simulink model "Project3_System_partA"  (R2018b)
settings: Solver=VariableStepAuto  StartTime=0.0  StopTime=10  FixedStep=.001  MaxStep=.001  RelTol=1e-6  EnableMultiTasking=on
values from neighbouring files (symbols this model uses):
  Kd = 700    [SimRun.m]
  Kp = 1000    [SimRun.m]
  n = link.inertia*(iwdot) + cross(iw, link.inertia*iw)    [newtonEuler.m]
  points = points3D    [SimRun.m]
  transPercent = 0.025    [SimRun.m]
(part 2 of 4)

== matlab function Project3_System_partA/ABB Arm Dynamics/MATLAB Function ==
  settings: updateMethod=DISCRETE
  data: torque input; theta_ddot output; theta input; theta_dot input
function theta_ddot = fcn(torque, theta, theta_dot )
%#codegen
coder.extrinsic('evalin');
persistent Sim_Exact;

if isempty(Sim_Exact)
    Sim_Exact = evalin('base','Sim_Exact');
end

th1 = theta(1);
th2 = theta(2);
th3 = theta(3);
th4 = theta(4);
th5 = theta(5);
th6 = theta(6);

th_dot1 = theta_dot(1);
th_dot2 = theta_dot(2);
th_dot3 = theta_dot(3);
th_dot4 = theta_dot(4);
th_dot5 = theta_dot(5);
th_dot6 = theta_dot(6);

CFG = zeros(6,1);
M = zeros(6,6);
if Sim_Exact
    CFG =  CFG_vec_exact(th1,th2,th3,th4,th5,th6,th_dot1,th_dot2,th_dot3,th_dot4,th_dot5,th_dot6);
    M = M_mat_exact(th1,th2,th3,th4,th5,th6);
else
    CFG =  CFG_vec_diff(th1,th2,th3,th4,th5,th6,th_dot1,th_dot2,th_dot3,th_dot4,th_dot5,th_dot6);
    M = M_mat_diff(th1,th2,th3,th4,th5,th6);
end

theta_ddot = M^-1 * (torque - CFG);

end

function CFG = CFG_vec_exact(th1,th2,th3,th4,th5,th6,thDot1,thDot2,thDot3,thDot4,thDot5,thDot6)
%CFG_VEC_EXACT
%    CFG = CFG_VEC_EXACT(TH1,TH2,TH3,TH4,TH5,TH6,THDOT1,THDOT2,THDOT3,THDOT4,THDOT5,THDOT6)

%    This function was generated by the Symbolic Math Toolbox version 7.0.
%    21-Nov-2018 15:36:09

t2 = th2+th3;
t3 = sin(t2);
t4 = sin(th6);
t5 = cos(th4);
t6 = cos(t2);
t7 = sin(th4);
t8 = cos(th6);
t9 = cos(th5);
t10 = sin(th1);
t11 = cos(th1);
t12 = sin(th5);
t13 = t6.*t12;
t14 = t3.*t5.*t9;
t15 = t13+t14;
t16 = t7.*t10;
t17 = t5.*t6.*t11;
t18 = t16+t17;
t19 = t9.*t18;
t47 = t3.*t11.*t12;
t20 = t19-t47;
t21 = t5.*t10;
t36 = t6.*t7.*t11;
t22 = t21-t36;
t23 = thDot2+thDot3;
t24 = t11.*t23;
t25 = t5.*t11;
t26 = t6.*t7.*t10;
t27 = t25+t26;
t28 = t27.*thDot5;
t33 = t3.*t10.*thDot4;
t29 = t24-t33;
t30 = t6.*thDot4;
t31 = t3.*t7.*thDot5;
t32 = t30+t31-thDot1;
t34 = t6.*t9;
t95 = t3.*t5.*t12;
t35 = t34-t95;
t37 = t5.*t10.*6.174272671239708e-4;
t49 = t6.*t7.*t11.*6.174272671239708e-4;
t38 = t37-t49;
t39 = t12.*t18.*2.88132724657853e-3;
t40 = t3.*t9.*t11.*2.88132724657853e-3;
t41 = t39+t40;
t42 = t12.*t18;
t43 = t3.*t9.*t11;
t44 = t42+t43;
t45 = t9.*t18.*2.88132724657853e-3;
t50 = t3.*t11.*t12.*2.88132724657853e-3;
t46 = t45-t50;
t48 = t24+t28-t33;
t51 = t7.*t11;
t53 = t5.*t6.*t10;
t52 = t51-t53;
t54 = t12.*t52;
t88 = t3.*t9.*t10;
t55 = t54-t88;
t56 = cos(th2);
t57 = t10.*t23;
t58 = t3.*t11.*thDot4;
t59 = t57+t58;
t60 = t30-thDot1;
t61 = thDot1.^2;
t62 = thDot2.^2;
t63 = cos(th3);
t64 = sin(th2);
t65 = sin(th3);
t66 = thDot3.^2;
t67 = t10.*t64.*thDot1.*thDot2.*(2.7e1./5.0e1);
t68 = t11.*t61.*t64.*t65.*(7.0./1.0e2);
t69 = t11.*t62.*t64.*t65.*(7.0./1.0e2);
t70 = t11.*t64.*t65.*t66.*(7.0./1.0e2);
t71 = t10.*t56.*t65.*thDot1.*thDot2.*(7.0./5.0e1);
t72 = t10.*t63.*t64.*thDot1.*thDot2.*(7.0./5.0e1);
t73 = t10.*t56.*t65.*thDot1.*thDot3.*(7.0./5.0e1);
t74 = t10.*t63.*t64.*thDot1.*thDot3.*(7.0./5.0e1);
t75 = t11.*t64.*t65.*thDot2.*thDot3.*(7.0./5.0e1);
t76 = t6.*7.0;
t77 = t56.*2.7e1;
t78 = t76+t77;
t79 = t11.*t56.*(2.7e1./1.0e2);
t80 = t6.*t11.*(7.0./2.0e2);
t132 = t11.*t78.*(1.0./1.0e2);
t81 = t79+t80-t132;
t82 = t10.*t56.*(2.7e1./1.0e2);
t83 = t6.*t10.*(7.0./2.0e2);
t168 = t10.*t78.*(1.0./1.0e2);
t84 = t82+t83-t168;
t85 = t9.*t52;
t86 = t3.*t10.*t12;
t87 = t85+t86;
t89 = t55.*thDot6;
t90 = t22.*thDot5;
t91 = t8.*t27.*(9.0./2.5e2);
t92 = t12.*t52.*(9.0./1.25e2);
t144 = t4.*t87.*(9.0./2.5e2);
t145 = t3.*t9.*t10.*(9.0./1.25e2);
t93 = t91+t92-t144-t145;
t94 = t24+t28-t33+t89;
t96 = t35.*thDot6;
t97 = t30+t31+t96-thDot1;
t98 = t8.*t22.*(9.0./2.5e2);
t99 = t12.*t18.*(9.0./1.25e2);
t100 = t3.*t9.*t11.*(9.0./1.25e2);
t133 = t4.*t20.*(9.0./2.5e2);
t101 = t98+t99+t100-t133;
t102 = t44.*thDot6;
t103 = t57+t58+t90+t102;
t104 = t4.*t15.*(9.0./2.5e2);
t105 = t6.*t9.*(9.0./1.25e2);
t106 = t3.*t7.*t8.*(9.0./2.5e2);
t147 = t3.*t5.*t12.*(9.0./1.25e2);
t107 = t104+t105+t106-t147;
t108 = t57+t58+t90;
t109 = t59.*thDot1;
t110 = t10.*t23.*thDot1;
t111 = t11.*t56.*t61.*t65.*(1.51e2./5.0e2);
t112 = t11.*t61.*t63.*t64.*(1.51e2./5.0e2);
t113 = t11.*t56.*t62.*t65.*(1.51e2./5.0e2);
t114 = t11.*t62.*t63.*t64.*(1.51e2./5.0e2);
t115 = t11.*t56.*t65.*t66.*(1.51e2./5.0e2);
t116 = t11.*t63.*t64.*t66.*(1.51e2./5.0e2);
t117 = t10.*t56.*t63.*thDot1.*thDot2.*(1.51e2./2.5e2);
t118 = t10.*t56.*t63.*thDot1.*thDot3.*(1.51e2./2.5e2);
t119 = t11.*t56.*t65.*thDot2.*thDot3.*(1.51e2./2.5e2);
t120 = t11.*t63.*t64.*thDot2.*thDot3.*(1.51e2./2.5e2);
t121 = t8.*t15.*6.694531704772773e-4;
t203 = t3.*t4.*t7.*6.694531704772773e-4;
t122 = t121-t203;
t123 = t4.*t15.*3.556381058634072e-4;
t124 = t3.*t7.*t8.*3.556381058634072e-4;
t125 = t123+t124;
t126 = t6.*t9.*6.694531704772773e-4;
t202 = t3.*t5.*t12.*6.694531704772773e-4;
t127 = t126-t202;
t128 = t32.*t59;
t129 = t97.*t108;
t130 = t10.*t23.*(t30-thDot1);
t227 = t60.*t108;
t288 = t32.*t103;
t131 = t109+t110+t128+t129+t130-t227-t288;
t134 = t3.*thDot2.*thDot4;
t135 = t3.*thDot3.*thDot4;
t136 = t3.*t9.*thDot2.*thDot6;
t137 = t3.*t9.*thDot3.*thDot6;
t138 = t6.*t12.*thDot5.*thDot6;
t139 = t5.*t6.*t12.*thDot2.*thDot6;
t140 = t5.*t6.*t12.*thDot3.*thDot6;
t141 = t3.*t5.*t9.*thDot5.*thDot6;
t209 = t6.*t7.*thDot2.*thDot5;
t210 = t6.*t7.*thDot3.*thDot5;
t211 = t3.*t5.*thDot4.*thDot5;
t212 = t3.*t7.*t12.*thDot4.*thDot6;
t142 = t134+t135+t136+t137+t138+t139+t140+t141-t209-t210-t211-t212;
t143 = t94.*t101;
t248 = t93.*t103;
t146 = t143-t248;
t148 = t29.*thDot1;
t149 = t29.*t32;
t150 = t48.*t97;
t151 = t11.*t23.*thDot1;
t152 = t11.*t23.*t60;
t153 = t3.*t11.*t29.*(1.51e2./1.0e3);
t154 = t3.*t10.*t59.*(1.51e2./1.0e3);
t155 = t153+t154;
t156 = t10.*t56.*t61.*(2.7e1./1.0e2);
t157 = t10.*t56.*t62.*(2.7e1./1.0e2);
t158 = t11.*t64.*thDot1.*thDot2.*(2.7e1./5.0e1);
t159 = t3.^2;
t160 = t10.*t56.*t61.*t63.*(7.0./1.0e2);
t161 = t10.*t56.*t62.*t63.*(7.0./1.0e2);
t162 = t10.*t56.*t63.*t66.*(7.0./1.0e2);
t163 = t11.*t56.*t65.*thDot1.*thDot2.*(7.0./5.0e1);
t164 = t11.*t63.*t64.*thDot1.*thDot2.*(7.0./5.0e1);
t165 = t11.*t56.*t65.*thDot1.*thDot3.*(7.0./5.0e1);
t166 = t11.*t63.*t64.*thDot1.*thDot3.*(7.0./5.0e1);
t167 = t10.*t56.*t63.*thDot2.*thDot3.*(7.0./5.0e1);
t169 = t11.*t23.*t81;
t170 = t10.*t23.*t84;
t171 = t169+t170;
t172 = t11.*t56.*t63.*thDot1.*thDot2.*(1.51e2./2.5e2);
t173 = t11.*t56.*t63.*thDot1.*thDot3.*(1.51e2./2.5e2);
t174 = t12.*t52.*6.694531704772773e-4;
t186 = t3.*t9.*t10.*6.694531704772773e-4;
t175 = t174-t186;
t176 = t8.*t87.*6.694531704772773e-4;
t177 = t4.*t27.*6.694531704772773e-4;
t178 = t176+t177;
t179 = t4.*t22;
t180 = t8.*t20;
t181 = t179+t180;
t182 = t8.*t27.*3.556381058634072e-4;
t183 = t4.*t20;
t243 = t8.*t22;
t184 = t183-t243;
t190 = t4.*t87.*3.556381058634072e-4;
t185 = t182-t190;
t187 = t8.*t87;
t188 = t4.*t27;
t189 = t187+t188;
t191 = t8.*t27;
t245 = t4.*t87;
t192 = t191-t245;
t193 = t5.*t11.*6.174272671239708e-4;
t194 = t6.*t7.*t10.*6.174272671239708e-4;
t195 = t193+t194;
t196 = t12.*t52.*2.88132724657853e-3;
t201 = t3.*t9.*t10.*2.88132724657853e-3;
t197 = t196-t201;
t198 = t9.*t52.*2.88132724657853e-3;
t199 = t3.*t10.*t12.*2.88132724657853e-3;
t200 = t198+t199;
t204 = t8.*t15;
t234 = t3.*t4.*t7;
t205 = t204-t234;
t206 = t4.*t15;
t207 = t3.*t7.*t8;
t208 = t206+t207;
t213 = t6.*t9.*2.88132724657853e-3;
t226 = t3.*t5.*t12.*2.88132724657853e-3;
t214 = t213-t226;
t215 = t6.*t12.*2.88132724657853e-3;
t216 = t3.*t5.*t9.*2.88132724657853e-3;
t217 = t215+t216;
t218 = t5.*t10.*1.570529909265897e-1;
t223 = t6.*t7.*t11.*1.570529909265897e-1;
t219 = t218-t223;
t220 = t7.*t10.*1.570529909265897e-1;
t221 = t5.*t6.*t11.*1.570529909265897e-1;
t222 = t220+t221;
t224 = t3.*t6.*t11.*2.386726843794421e-2;
t225 = t148+t151+t152;
t228 = t7.*t11.*1.570529909265897e-1;
t233 = t5.*t6.*t10.*1.570529909265897e-1;
t229 = t228-t233;
t230 = t5.*t11.*1.570529909265897e-1;
t231 = t6.*t7.*t10.*1.570529909265897e-1;
t232 = t230+t231;
t235 = t12.*t18.*6.694531704772773e-4;
t236 = t3.*t9.*t11.*6.694531704772773e-4;
t237 = t235+t236;
t238 = t4.*t22.*6.694531704772773e-4;
t239 = t8.*t20.*6.694531704772773e-4;
t240 = t238+t239;
t241 = t4.*t20.*3.556381058634072e-4;
t244 = t8.*t22.*3.556381058634072e-4;
t242 = t241-t244;
t246 = t3.*t6.*t10.*2.386726843794421e-2;
t247 = t101.*t142;
t249 = t93.*t97;
t274 = t94.*t107;
t250 = t249-t274;
t251 = t97.*t250;
t275 = t48.*t60;
t276 = t32.*t94;
t252 = t148+t149+t150+t151+t152-t275-t276;
t253 = t107.*t252;
t254 = t10.*t56.*t61.*t65.*(1.51e2./5.0e2);
t255 = t10.*t61.*t63.*t64.*(1.51e2./5.0e2);
t256 = t10.*t56.*t62.*t65.*(1.51e2./5.0e2);
t257 = t10.*t62.*t63.*t64.*(1.51e2./5.0e2);
t258 = t10.*t56.*t65.*t66.*(1.51e2./5.0e2);
t259 = t10.*t63.*t64.*t66.*(1.51e2./5.0e2);
t260 = t10.*t61.*t64.*t65.*(7.0./1.0e2);
t261 = t10.*t62.*t64.*t65.*(7.0./1.0e2);
t262 = t10.*t64.*t65.*t66.*(7.0./1.0e2);
t263 = t11.*t64.*t65.*thDot1.*thDot2.*(1.51e2./2.5e2);
t264 = t11.*t64.*t65.*thDot1.*thDot3.*(1.51e2./2.5e2);
t265 = t10.*t56.*t65.*thDot2.*thDot3.*(1.51e2./2.5e2);
t266 = t10.*t63.*t64.*thDot2.*thDot3.*(1.51e2./2.5e2);
t267 = t10.*t64.*t65.*thDot2.*thDot3.*(7.0./5.0e1);
t268 = t6.*t29.*(1.51e2./1.0e3);
t269 = t3.*t10.*t60.*(1.51e2./1.0e3);
t270 = t268+t269;
t271 = t11.*t23.*t159.*thDot4.*(1.51e2./1.0e3);
t272 = t6.*t225.*(1.51e2./1.0e3);
t273 = -t156-t157-t158-t160-t161-t162-t163-t164-t165-t166-t167-t172-t173+t254+t255+t256+t257+t258+t259+t260+t261+t262+t263+t264+t265+t266+t267;
t277 = t156+t157+t158+t160+t161+t162+t163+t164+t165+t166+t167+t172+t173+t247+t251+t253-t254-t255-t256-t257-t258-t259-t260-t261-t262-t263-t264-t265-t266-t267-t103.*t146;
t278 = t277.*pi.*3.6225e-1;
t297 = t59.*t155;
t298 = t60.*t270;
t279 = t156+t157+t158+t160+t161+t162+t163+t164+t165+t166+t167-t260-t261-t262-t267+t271+t272-t297-t298;
t280 = t279.*pi.*6.07775;
t281 = t10.^2;
t282 = t6.^2;
t283 = t11.^2;
t284 = -t91-t92+t144+t145;
t285 = t97.*t101;
t329 = t103.*t107;
t286 = t285-t329;
t287 = t97.*t286;
t289 = t107.*t131;
t290 = t56.^2;
t291 = t64.^2;
t292 = t10.*t11.*t282.*5.532148313430778e-3;
t293 = t10.*t11.*t159.*4.573242605769442e-3;
t407 = t10.*t11.*4.573242605769442e-3;
t294 = t292+t293-t407;
t295 = t103.*t284;
t296 = t143+t295;
t299 = t84.*thDot1;
t345 = t3.*t11.*t23.*(7.0./2.0e2);
t300 = t299-t345;
t301 = t3.*t11.*t23.*thDot1.*(7.0./2.0e2);
t346 = t300.*thDot1;
t347 = t10.*t23.*t171;
t302 = t156+t157+t158+t301-t346-t347;
t303 = t302.*pi.*1.40875;
t304 = t10.*t11.*t290.*1.080250746560099e-1;
t305 = t10.*t11.*t291.*2.873466985849863e-1;
t399 = t10.*t11.*2.873466985849863e-1;
t306 = t304+t305-t399;
t307 = t103.*t296;
t308 = t97.*t284;
t309 = t274+t308;
t310 = t97.*t309;
t311 = -t156-t157-t158-t160-t161-t162-t163-t164-t165-t166-t167-t172-t173-t247-t253+t254+t255+t256+t257+t258+t259+t260+t261+t262+t263+t264+t265+t266+t267+t307+t310;
t312 = t109+t110+t130;
t313 = t29.*t155;
t314 = t6.*t59.*(1.51e2./1.0e3);
t339 = t3.*t11.*t60.*(1.51e2./1.0e3);
t315 = t314-t339;
t316 = t10.*t23.*t159.*thDot4.*(1.51e2./1.0e3);
t324 = t11.*t56.*t61.*(2.7e1./1.0e2);
t325 = t11.*t56.*t62.*(2.7e1./1.0e2);
t330 = t11.*t56.*t61.*t63.*(7.0./1.0e2);
t331 = t11.*t56.*t62.*t63.*(7.0./1.0e2);
t332 = t11.*t56.*t63.*t66.*(7.0./1.0e2);
t333 = t11.*t56.*t63.*thDot2.*thDot3.*(7.0./5.0e1);
t334 = t10.*t64.*t65.*thDot1.*thDot2.*(1.51e2./2.5e2);
t335 = t10.*t64.*t65.*thDot1.*thDot3.*(1.51e2./2.5e2);
t317 = t67+t68+t69+t70+t71+t72+t73+t74+t75+t111+t112+t113+t114+t115+t116+t117+t118+t119+t120-t324-t325-t330-t331-t332-t333-t334-t335;
t318 = t317.*pi.*(1.61e2./2.56e2);
t319 = t81.*thDot1;
t320 = t3.*t10.*t23.*(7.0./2.0e2);
t321 = t319+t320;
t322 = t321.*thDot1;
t323 = t11.*t23.*t171;
t326 = t3.*t10.*t23.*thDot1.*(7.0./2.0e2);
t327 = t142.*t284;
t328 = t94.*t296;
t336 = t67+t68+t69+t70+t71+t72+t73+t74+t75+t111+t112+t113+t114+t115+t116+t117+t118+t119+t120+t287+t289-t324-t325+t327+t328-t330-t331-t332-t333-t334-t335;
t337 = t336.*pi.*3.6225e-1;
t338 = t6.*t312.*(1.51e2./1.0e3);
t342 = t60.*t315;
t340 = t67+t68+t69+t70+t71+t72+t73+t74+t75+t313+t316-t324-t325-t330-t331-t332-t333+t338-t342;
t341 = t340.*pi.*6.07775;
t343 = t318+t337+t341;
t344 = t311.*pi.*3.6225e-1;
t348 = t273.*pi.*(1.61e2./2.56e2);
t349 = t56.*t283.*thDot2.*(2.7e1./2.0e2);
t350 = t56.*t281.*thDot2.*(2.7e1./2.0e2);
t351 = t349+t350;
t352 = t67+t322+t323-t324-t325+t326;
t353 = t352.*pi.*1.40875;
t354 = t7.^2;
t355 = t205.*t240;
t356 = t208.*t242;
t586 = t35.*t237;
t357 = t355+t356-t586;
t358 = t44.*t237;
t359 = t181.*t240;
t360 = t184.*t242;
t361 = t358+t359+t360;
t362 = t103.*t361;
t363 = t55.*t237;
t364 = t189.*t240;
t558 = t192.*t242;
t365 = t363+t364-t558;
t366 = t94.*t365;
t605 = t97.*t357;
t367 = t362+t366-t605;
t368 = t35.*t197;
t369 = t3.*t7.*t195;
t549 = t15.*t200;
t370 = t368+t369-t549;
t371 = -t134-t135+t209+t210+t211;
t372 = t11.*t56.*thDot1.*(2.7e1./2.0e2);
t520 = t10.*t64.*thDot2.*(2.7e1./2.0e2);
t373 = t372-t520;
t374 = t373.*thDot1;
t375 = t11.*t351.*thDot2;
t376 = t374+t375-t10.*t64.*thDot1.*thDot2.*(2.7e1./2.0e2);
t377 = t318+t337+t341+t353-t376.*pi.*1.22259375e1;
t378 = t282.*2.386726843794421e-2;
t379 = t5.^2;
t380 = t159.*t379.*1.570529909265897e-1;
t381 = t159.*t354.*1.570529909265897e-1;
t382 = t378+t380+t381;
t383 = t3.*t7.*t22.*1.570529909265897e-1;
t555 = t3.*t5.*t18.*1.570529909265897e-1;
t384 = t224+t383-t555;
t385 = t3.*t5.*t52.*1.570529909265897e-1;
t557 = t3.*t7.*t27.*1.570529909265897e-1;
t386 = t246+t385-t557;
t387 = t22.*t195;
t388 = t44.*t197;
t389 = t20.*t200;
t390 = t387+t388+t389;
t391 = t44.*t175;
t392 = t178.*t181;
t573 = t184.*t185;
t393 = t391+t392-t573;
t394 = t11.*t23.*(t30-thDot1);
t395 = t159.*t281.*2.386726843794421e-2;
t396 = t27.*t232;
t397 = t52.*t229;
t398 = t395+t396+t397;
t400 = t11.*t306.*thDot2;
t401 = t281.*2.873466985849863e-1;
t402 = t283.*t290.*1.080250746560099e-1;
t403 = t283.*t291.*2.873466985849863e-1;
t404 = t401+t402+t403;
t405 = t11.*t56.*t64.*thDot1.*1.793216239289764e-1;
t406 = t400+t405-t10.*t404.*thDot2;
t408 = t281.*4.573242605769442e-3;
t409 = t282.*t283.*5.532148313430778e-3;
t410 = t159.*t283.*4.573242605769442e-3;
t411 = t408+t409+t410;
t412 = t10.*t23.*t411;
t413 = t3.*t6.*t11.*thDot1.*9.589057076613353e-4;
t610 = t11.*t23.*t294;
t414 = t412+t413-t610;
t415 = t35.*t127;
t416 = t122.*t205;
t417 = t125.*t208;
t418 = t415+t416+t417;
t419 = t122.*t181;
t420 = t125.*t184;
t569 = t44.*t127;
t421 = t419+t420-t569;
t422 = t125.*t192;
t423 = t55.*t127;
t570 = t122.*t189;
t424 = t422+t423-t570;
t425 = t15.*t217;
t426 = t35.*t214;
t427 = t159.*t354.*6.174272671239708e-4;
t428 = t425+t426+t427;
t429 = t44.*t214;
t430 = t3.*t7.*t22.*6.174272671239708e-4;
t563 = t20.*t217;
t431 = t429+t430-t563;
t432 = t55.*t214;
t433 = t3.*t7.*t27.*6.174272671239708e-4;
t565 = t87.*t217;
t434 = t432+t433-t565;
t435 = t27.*t195;
t436 = t87.*t200;
t437 = t55.*t197;
t438 = t435+t436+t437;
t439 = t109+t110+t128+t130-t227;
t440 = t318+t337+t341+t353;
t441 = t55.*t175;
t442 = t178.*t189;
t443 = t185.*t192;
t444 = t441+t442+t443;
t445 = t62.*t64.*(2.7e1./1.0e2);
t446 = t148+t149+t150+t151-t275-t276+t394;
t447 = t3.*t62.*(7.0./1.0e2);
t448 = t3.*t66.*(7.0./1.0e2);
t449 = t3.*thDot2.*thDot3.*(7.0./5.0e1);
t450 = t6.*t62.*(1.51e2./5.0e2);
t451 = t6.*t66.*(1.51e2./5.0e2);
t452 = t6.*thDot2.*thDot3.*(1.51e2./2.5e2);
t453 = t318+t337;
t454 = t18.*t229;
t455 = t22.*t232;
t465 = t10.*t11.*t159.*2.386726843794421e-2;
t456 = t454+t455-t465;
t457 = t148+t151+t394;
t458 = t159.*t283.*2.386726843794421e-2;
t459 = t18.*t222;
t460 = t22.*t219;
t461 = t458+t459+t460;
t462 = t59.*t461;
t463 = t27.*t219;
t464 = t52.*t222;
t466 = -t30+thDot1;
t467 = t3.*t7.*t219;
t604 = t3.*t5.*t222;
t468 = t224+t467-t604;
t469 = t35.*t41;
t470 = t3.*t7.*t38;
t592 = t15.*t46;
t471 = t469+t470-t592;
t472 = t32.*t471;
t473 = t22.*t38;
t474 = t41.*t44;
t475 = t20.*t46;
t476 = t473+t474+t475;
t477 = t108.*t476;
t478 = t27.*t38;
t479 = t46.*t87;
t480 = t41.*t55;
t481 = t478+t479+t480;
t482 = t48.*t481;
t483 = t472+t477+t482;
t484 = t185.*t208;
t485 = t35.*t175;
t572 = t178.*t205;
t486 = t484+t485-t572;
t495 = t10.*t23.*t466;
t487 = t109+t110-t495;
t488 = t6.*t487.*(1.51e2./1.0e3);
t489 = t3.*t11.*t466.*(1.51e2./1.0e3);
t490 = t314+t489;
t491 = t466.*t490;
t492 = t67+t68+t69+t70+t71+t72+t73+t74+t75+t313+t316-t324-t325-t330-t331-t332-t333+t488+t491;
t493 = t492.*pi.*6.07775;
t494 = t108.*t466;
t496 = t10.*t23.*t321;
t497 = t11.*t23.*t84.*thDot1;
t511 = t11.*t23.*t300;
t512 = t10.*t23.*t81.*thDot1;
t498 = t445+t496+t497-t511-t512+4.9e1./5.0;
t499 = t498.*pi.*1.40875;
t500 = t94.*t309;
t501 = t109+t110+t128+t129-t288+t494-t495;
t502 = t445+t447+t448+t449+t450+t451+t452+4.9e1./5.0;
t503 = t502.*pi.*(1.61e2./2.56e2);
t504 = t107.*t501;
t505 = t67+t68+t69+t70+t71+t72+t73+t74+t75+t111+t112+t113+t114+t115+t116+t117+t118+t119+t120+t287-t324-t325+t327+t328-t330-t331-t332-t333-t334-t335+t504;
t506 = t48.*t466;
t516 = t11.*t23.*t466;
t507 = t148+t149+t150+t151-t276+t506-t516;
t508 = t284.*t507;
t521 = t103.*t286;
t522 = t101.*t501;
t509 = t445+t447+t448+t449+t450+t451+t452+t500+t508-t521-t522+4.9e1./5.0;
t510 = t509.*pi.*3.6225e-1;
t513 = t59.*t490;
t523 = t3.*t10.*t466.*(1.51e2./1.0e3);
t514 = t268-t523;
t515 = t29.*t514;
t517 = t10.*t56.*thDot1.*(2.7e1./2.0e2);
t518 = t11.*t64.*thDot2.*(2.7e1./2.0e2);
t519 = t517+t518;
t524 = t148+t151-t516;
t525 = t3.*t10.*t524.*(1.51e2./1.0e3);
t528 = t3.*t11.*t487.*(1.51e2./1.0e3);
t526 = t445+t447+t448+t449+t513+t515+t525-t528+4.9e1./5.0;
t527 = t526.*pi.*6.07775;
t529 = t503+t510+t527;
t530 = t283.*4.573242605769442e-3;
t531 = t281.*t282.*5.532148313430778e-3;
t532 = t159.*t281.*4.573242605769442e-3;
t533 = t530+t531+t532;
t534 = t283.*2.873466985849863e-1;
t535 = t281.*t290.*1.080250746560099e-1;
t536 = t281.*t291.*2.873466985849863e-1;
t537 = t534+t535+t536;
t538 = t3.*t5.*t229;
t591 = t3.*t7.*t232;
t539 = t246+t538-t591;
t540 = t505.*pi.*3.6225e-1;
t541 = t318+t493+t540;
t547 = t107.*t507;
t542 = -t156-t157-t158-t160-t161-t162-t163-t164-t165-t166-t167-t172-t173-t247+t254+t255+t256+t257+t258+t259+t260+t261+t262+t263+t264+t265+t266+t267+t307+t310-t547;
t543 = t6.*t524.*(1.51e2./1.0e3);
t544 = t466.*t514;
t545 = t156+t157+t158+t160+t161+t162+t163+t164+t165+t166+t167-t260-t261-t262-t267+t271-t297+t543+t544;
t546 = t545.*pi.*6.07775;
t548 = t542.*pi.*3.6225e-1;
t550 = t32.*t370;
t551 = t108.*t390;
t552 = t48.*t438;
t553 = t550+t551+t552;
t554 = t348-t546+t548;
t556 = t59.*t384;
t559 = t11.*t537.*thDot2;
t560 = t10.*t56.*t64.*thDot1.*1.793216239289764e-1;
t561 = t559+t560-t10.*t306.*thDot2;
t562 = t32.*t428;
t564 = t108.*t431;
t566 = t48.*t434;
t567 = t562+t564+t566;
t568 = t97.*t418;
t571 = t94.*t424;
t574 = t103.*t393;
t575 = t94.*t444;
t576 = t97.*t486;
t577 = t574+t575+t576;
t578 = t519.*thDot1;
t579 = t10.*t351.*thDot2;
t580 = t11.*t64.*thDot1.*thDot2.*(2.7e1./2.0e2);
t581 = t578+t579+t580;
t582 = t581.*pi.*1.22259375e1;
t583 = t10.*t23.*t294;
t584 = t3.*t6.*t10.*thDot1.*9.589057076613353e-4;
t634 = t11.*t23.*t533;
t585 = t583+t584-t634;
t587 = t463+t464-t465;
t588 = t499+t503+t510+t527;
t589 = t29.*t398;
t590 = t59.*t456;
t593 = t503+t510;
t594 = t11.*t519.*thDot2;
t595 = t594-t10.*t373.*thDot2+4.9e1./5.0;
t596 = t595.*pi.*1.22259375e1;
t597 = t499+t503+t510+t527+t596;
t598 = t282.*4.573242605769442e-3;
t599 = t159.*5.532148313430778e-3;
t600 = t598+t599;
t601 = t290.*2.873466985849863e-1;
t602 = t291.*1.080250746560099e-1;
t603 = t601+t602;
t606 = t382.*t466;
t607 = t29.*t386;
t608 = -t556+t606+t607;
t609 = t148+t149+t151+t506-t516;
t611 = t414.*thDot1;
t632 = t103.*t421;
t612 = t568+t571-t632;
t613 = t103.*t612;
t614 = t108.*t567;
t615 = t109+t110+t128+t494-t495;
t616 = t29.*t587;
t651 = t466.*t468;
t617 = t462+t616-t651;
t618 = t466.*t617;
t619 = t142.*t486;
t620 = t6.*t541.*(1.51e2./1.0e3);
t621 = t3.*t541.*(7.0./2.0e2);
t622 = t107.*t505.*pi.*3.6225e-1;
t623 = t3.*t10.*thDot4.*(1.0./1.0e1);
t624 = t6.*t11.*t529.*(7.0./2.0e2);
t625 = t10.*t23.*t533.*thDot1;
t626 = t11.*t23.*t294.*thDot1;
t627 = t22.*thDot5.*(1.0./1.0e1);
t628 = t361.*t507;
t629 = t461.*t524;
t630 = t476.*t609;
t631 = t48.*t567;
t633 = t44.*thDot6.*(1.0./2.0e1);
t635 = t142.*t357;
t636 = t10.*thDot3.*3.0;
t637 = t348+t548;
t638 = t84.*t588;
t639 = t466.*t539;
t640 = t589+t590+t639;
t641 = t466.*t640;
t642 = t371.*t471;
t643 = t3.*t10.*t529.*(1.51e2./1.0e3);
t644 = t3.*t11.*thDot4.*(1.0./1.0e1);
t645 = t3.*t10.*t593.*(1.51e2./1.0e3);
t646 = t284.*t509.*pi.*3.6225e-1;
t647 = t10.*t23.*t294.*thDot1;
t648 = t11.*t23.*t411.*thDot1;
t649 = t48.*t483;
t650 = t142.*t418;
t652 = t94.*t367;
t653 = t318+t540;
t654 = t3.*t23.*t382.*thDot4;
t655 = t94.*(t568+t571-t632);
t656 = t97.*(t484+t485-t572);
t657 = (t182-t190).*(t191-t245);
t658 = t441+t442+t657;
t659 = t94.*t658;
t660 = t574+t656+t659;
t661 = t398.*t487;
t662 = t438.*t615;
t663 = t6.*t653.*(1.51e2./1.0e3);
t664 = t97.*t367;
t665 = t370.*t371;
t666 = t27.*thDot5.*(1.0./1.0e1);
t667 = t390.*t609;
t668 = t393.*t507;
t669 = t55.*thDot6.*(1.0./2.0e1);
t670 = t32.*t483;
t671 = t101.*t509.*pi.*3.6225e-1;
t672 = t103.*t660;
t673 = t108.*t553;
t674 = t371.*t428;
t675 = t431.*t609;
t676 = t35.*thDot6.*(1.0./2.0e1);
t677 = t3.*t7.*thDot5.*(1.0./1.0e1);
t678 = t101.*t542.*pi.*3.6225e-1;
t679 = t421.*t507;
t680 = t284.*t505.*pi.*3.6225e-1;
t681 = t424.*t501;
CFG = [t649+t650+t652+t654+thDot1.*3.0+t421.*(t148+t149+t150+t151+t152-t32.*(t24+t28+t89-t3.*t10.*thDot4)+(thDot1-t6.*thDot4).*(t24+t28-t3.*t10.*thDot4))+t131.*t424-t225.*t384-t108.*t553-t103.*t577-t312.*t386-t371.*t428+t434.*t439-t6.*thDot4.*(1.0./1.0e1)-t35.*thDot6.*(1.0./2.0e1)-t431.*(t148+t149+t151+t152-t48.*t60)-t59.*(t589+t590-t60.*t539)+t29.*(t462+t29.*(t463+t464-t10.*t11.*t159.*2.386726843794421e-2)+t468.*(t30-thDot1))+t84.*(t318+pi.*(t67+t68+t69+t70+t71+t72+t73+t74+t75+t111+t112+t113+t114+t115+t116+t117+t118+t119+t120+t287+t289-t93.*t142+t94.*t146-t11.*t56.*t61.*(2.7e1./1.0e2)-t11.*t56.*t62.*(2.7e1./1.0e2)-t11.*t56.*t61.*t63.*(7.0./1.0e2)-t11.*t56.*t62.*t63.*(7.0./1.0e2)-t11.*t56.*t63.*t66.*(7.0./1.0e2)-t11.*t56.*t63.*thDot2.*thDot3.*(7.0./5.0e1)-t10.*t64.*t65.*thDot1.*thDot2.*(1.51e2./2.5e2)-t10.*t64.*t65.*thDot1.*thDot3.*(1.51e2./2.5e2)).*3.6225e-1+pi.*(t67+t322+t323+t326-t11.*t56.*t61.*(2.7e1./1.0e2)-t11.*t56.*t62.*(2.7e1./1.0e2)).*1.40875+pi.*(t67+t68+t69+t70+t71+t72+t73+t74+t75+t313+t316-t60.*t315+t6.*(t109+t110+t10.*t23.*t60).*(1.51e2./1.0e3)-t11.*t56.*t61.*(2.7e1./1.0e2)-t11.*t56.*t62.*(2.7e1./1.0e2)-t11.*t56.*t61.*t63.*(7.0./1.0e2)-t11.*t56.*t62.*t63.*(7.0./1.0e2)-t11.*t56.*t63.*t66.*(7.0./1.0e2)-t11.*t56.*t63.*thDot2.*thDot3.*(7.0./5.0e1)).*6.07775)+t81.*(t303-t273.*pi.*(1.61e2./2.56e2)+pi.*(t156+t157+t158+t160+t161+t162+t163+t164+t165+t166+t167+t172+t173+t247+t251+t253-t103.*t146-t10.*t56.*t61.*t65.*(1.51e2./5.0e2)-t10.*t56.*t62.*t65.*(1.51e2./5.0e2)-t10.*t56.*t65.*t66.*(1.51e2./5.0e2)-t10.*t61.*t63.*t64.*(1.51e2./5.0e2)-t10.*t62.*t63.*t64.*(1.51e2./5.0e2)-t10.*t61.*t64.*t65.*(7.0./1.0e2)-t10.*t62.*t64.*t65.*(7.0./1.0e2)-t10.*t63.*t64.*t66.*(1.51e2./5.0e2)-t10.*t64.*t65.*t66.*(7.0./1.0e2)-t10.*t56.*t65.*thDot2.*thDot3.*(1.51e2./2.5e2)-t10.*t63.*t64.*thDot2.*thDot3.*(1.51e2./2.5e2)-t11.*t64.*t65.*thDot1.*thDot2.*(1.51e2./2.5e2)-t10.*t64.*t65.*thDot2.*thDot3.*(7.0./5.0e1)-t11.*t64.*t65.*thDot1.*thDot3.*(1.51e2./2.5e2)).*3.6225e-1+pi.*(t156+t157+t158+t160+t161+t162+t163+t164+t165+t166+t167+t271+t272-t59.*t155-t60.*t270-t10.*t61.*t64.*t65.*(7.0./1.0e2)-t10.*t62.*t64.*t65.*(7.0./1.0e2)-t10.*t64.*t65.*t66.*(7.0./1.0e2)-t10.*t64.*t65.*thDot2.*thDot3.*(7.0./5.0e1)).*6.07775)-t11.*t56.*(t280+t303-t344-t348).*(2.7e1./2.0e2)-t11.*t56.*(t280+t303+t582-t273.*pi.*(1.61e2./2.56e2)-t311.*pi.*3.6225e-1).*(2.7e1./2.0e2)-t3.*t11.*(t344+t348).*(1.51e2./1.0e3)-t101.*t311.*pi.*3.6225e-1+t3.*t11.*(t278+t280-t273.*pi.*(1.61e2./2.56e2)).*(1.51e2./1.0e3)-t6.*t11.*(t278+t280-t273.*pi.*(1.61e2./2.56e2)).*(7.0./2.0e2)+t3.*t10.*t343.*(1.51e2./1.0e3)-t6.*t10.*t343.*(7.0./2.0e2)-t10.*t56.*t377.*(2.7e1./2.0e2)+t11.*t23.*t414+t3.*t10.*t453.*(1.51e2./1.0e3)-t10.*t56.*t440.*(2.7e1./2.0e2)+t10.*t23.*t585-t3.*t7.*thDot5.*(1.0./1.0e1)-t11.*t406.*thDot2-t10.*t561.*thDot2+t284.*pi.*(t67+t68+t69+t70+t71+t72+t73+t74+t75+t111+t112+t113+t114+t115+t116+t117+t118+t119+t120+t287+t289+t327+t328-t11.*t56.*t61.*(2.7e1./1.0e2)-t11.*t56.*t62.*(2.7e1./1.0e2)-t11.*t56.*t61.*t63.*(7.0./1.0e2)-t11.*t56.*t62.*t63.*(7.0./1.0e2)-t11.*t56.*t63.*t66.*(7.0./1.0e2)-t11.*t56.*t63.*thDot2.*thDot3.*(7.0./5.0e1)-t10.*t64.*t65.*thDot1.*thDot2.*(1.51e2./2.5e2)-t10.*t64.*t65.*thDot1.*thDot3.*(1.51e2./2.5e2)).*3.6225e-1+t3.*t6.*t23.*t281.*thDot1.*9.589057076613353e-4+t3.*t6.*t23.*t283.*thDot1.*9.589057076613353e-4-t56.*t64.*t281.*thDot1.*thDot2.*1.793216239289764e-1-t56.*t64.*t283.*thDot1.*thDot2.*1.793216239289764e-1;t10.*(t627+t628+t629+t630+t631+t633+t635+t636+t638+t641+t642+t643+t644+t645+t646+t647+t648+t3.*(t303-t348+t546-t542.*pi.*3.6225e-1).*(7.0./2.0e2)+t64.*(t303-t348+t546-t548+t582).*(2.7e1./2.0e2)-t3.*t554.*(7.0./2.0e2)-t6.*t554.*(1.51e2./1.0e3)-t32.*t553-t29.*t608-t6.*t637.*(1.51e2./1.0e3)-t97.*t577+t94.*t612-t365.*t501-t487.*t587-t481.*t615+t10.*thDot2.*3.0+t561.*thDot1-t585.*thDot1+t64.*(t303-t348+t546-t548).*(2.7e1./2.0e2)-t107.*t542.*pi.*3.6225e-1-t6.*t10.*t529.*(7.0./2.0e2)-t10.*t56.*t588.*(2.7e1./2.0e2)-t10.*t56.*t597.*(2.7e1./2.0e2)-t3.*t23.*t468.*thDot4-t11.*t23.*t600.*thDot1+t10.*t306.*thDot1.*thDot2+t11.*t404.*thDot1.*thDot2-t11.*t603.*thDot1.*thDot2)-t11.*(t611+t613+t614+t618+t619+t620+t621+t622+t623+t624+t625+t626-t81.*(t499+t503+pi.*(t445+t447+t448+t449+t450+t451+t452+t500-t521-t101.*t131+t284.*t446+4.9e1./5.0).*3.6225e-1+pi.*(t445+t447+t448+t449+t29.*t270+t59.*t315-t3.*t11.*t312.*(1.51e2./1.0e3)+t3.*t10.*t457.*(1.51e2./1.0e3)+4.9e1./5.0).*6.07775)+t59.*(t556-t29.*t386+t60.*t382)+t64.*t377.*(2.7e1./2.0e2)+t3.*t440.*(7.0./2.0e2)+t6.*t453.*(1.51e2./1.0e3)-t97.*t367+t64.*t440.*(2.7e1./2.0e2)-t32.*t483+t131.*t444+t312.*t398-t370.*t371-t393.*t446+t438.*t439-t456.*t457-t11.*thDot2.*3.0-t11.*thDot3.*3.0-t27.*thDot5.*(1.0./1.0e1)-t55.*thDot6.*(1.0./2.0e1)-t406.*thDot1-t390.*(t148+t149+t151-t275+t394)-t101.*t509.*pi.*3.6225e-1-t3.*t11.*t529.*(1.51e2./1.0e3)-t3.*t11.*t593.*(1.51e2./1.0e3)+t11.*t56.*t588.*(2.7e1./2.0e2)+t11.*t56.*t597.*(2.7e1./2.0e2)-t3.*t23.*t539.*thDot4-t10.*t23.*t600.*thDot1+t11.*t306.*thDot1.*thDot2+t10.*t537.*thDot1.*thDot2-t10.*t603.*thDot1.*thDot2);t10.*(t627+t628+t629+t630+t631+t633+t635+t636+t638+t641+t642+t643+t644+t645+t646+t647+t648+t655-t3.*t554.*(7.0./2.0e2)-t6.*t554.*(1.51e2./1.0e3)-t32.*t553-t29.*t608-t6.*t637.*(1.51e2./1.0e3)-t97.*t577-t365.*t501-t487.*t587-t481.*t615-t585.*thDot1+t3.*(t303-t348+t546-t548).*(7.0./2.0e2)-t107.*t542.*pi.*3.6225e-1-t6.*t10.*t529.*(7.0./2.0e2)-t3.*t23.*t468.*thDot4-t11.*t23.*t600.*thDot1)-t11.*(t611+t613+t614+t618+t619+t620+t621+t622+t623+t624+t625+t626+t661+t662+t663+t3.*(t318+t353+t493+t540).*(7.0./2.0e2)-t97.*t367-t32.*t483-t59.*t608-t81.*t588-t370.*t371-t393.*t507+t444.*t501-t456.*t524-t390.*t609-t11.*thDot3.*3.0-t27.*thDot5.*(1.0./1.0e1)-t55.*thDot6.*(1.0./2.0e1)-t101.*t509.*pi.*3.6225e-1-t3.*t11.*t529.*(1.51e2./1.0e3)-t3.*t11.*t593.*(1.51e2./1.0e3)-t3.*t23.*t539.*thDot4-t10.*t23.*t600.*thDot1);t6.*(-t649-t650-t652-t654+t672+t673+t674+t675+t676+t677+t678-t29.*t617+t59.*t640+t386.*t487+t384.*t524-t424.*t501-t421.*t507-t434.*t615+t6.*thDot4.*(1.0./1.0e1)-t284.*t505.*pi.*3.6225e-1-t3.*t10.*t541.*(1.51e2./1.0e3)+t3.*t11.*t554.*(1.51e2./1.0e3)+t3.*t11.*t637.*(1.51e2./1.0e3)-t3.*t10.*t653.*(1.51e2./1.0e3))+t3.*t11.*(t627+t628+t629+t630+t631+t633+t635+t641+t642+t643+t644+t645+t646+t655-t6.*t554.*(1.51e2./1.0e3)-t32.*t553-t29.*t608-t6.*t637.*(1.51e2./1.0e3)-t97.*t660-t365.*t501-t487.*t587-t481.*t615-t107.*t542.*pi.*3.6225e-1-t3.*t23.*t468.*thDot4)-t3.*t10.*(-t613-t614-t618-t619-t620-t622-t623-t661-t662-t663+t664+t665+t666+t667+t668+t669+t670+t671+t59.*t608+t456.*t524-t501.*t658+t3.*t11.*t529.*(1.51e2./1.0e3)+t3.*t11.*t593.*(1.51e2./1.0e3)+t3.*t23.*t539.*thDot4);t27.*(-t613-t614-t619-t622-t662+t664+t665+t666+t667+t668+t669+t670+t671-t501.*t658)+t22.*(t627+t628+t630+t631+t633+t635+t642+t646+t655-t32.*t553-t97.*t660-t365.*t501-t481.*t615-t107.*t542.*pi.*3.6225e-1)-t3.*t7.*(t649+t650+t652-t672-t673-t674-t675-t676-t677-t678+t679+t680+t681+t434.*t615);-t55.*(t613+t619+t622-t664-t668-t669-t671+t501.*t658)+t44.*(t628+t633+t635+t646+t655-t97.*t660-t365.*t501-t107.*t542.*pi.*3.6225e-1)-t35.*(t650+t652-t672-t676-t678+t679+t680+t681)];
end
function M = M_mat_exact(th1,th2,th3,th4,th5,th6)
%M_MAT_EXACT
%    M = M_MAT_EXACT(TH1,TH2,TH3,TH4,TH5,TH6)

%    This function was generated by the Symbolic Math Toolbox version 7.0.
%    21-Nov-2018 15:42:48

t3 = th2+th3;
t2 = cos(t3);
t4 = cos(th5);
t5 = sin(t3);
t6 = cos(th4);
t7 = sin(th5);
t8 = cos(th6);
t9 = t2.*t7;
t10 = t4.*t5.*t6;
t11 = t9+t10;
t12 = sin(th4);
t13 = sin(th6);
t14 = cos(th1);
t15 = cos(th2);
t16 = sin(th1);
t17 = t12.*t16;
t18 = t2.*t6.*t14;
t19 = t17+t18;
t20 = t2.*7.0;
t21 = t15.*2.7e1;
t22 = t20+t21;
t23 = t2.*t14.*(7.0./2.0e2);
t24 = t5.*t14.*(1.51e2./5.0e2);
t25 = t2.*t4;
t191 = t5.*t6.*t7;
t26 = t25-t191;
t27 = sin(th2);
t28 = t5.^2;
t29 = t2.*t16.*(7.0./2.0e2);
t30 = t12.*t14;
t44 = t2.*t6.*t16;
t31 = t30-t44;
t32 = t16.*t22.*(1.0./1.0e2);
t33 = t4.*t19;
t64 = t5.*t7.*t14;
t34 = t33-t64;
t35 = t6.*t16;
t66 = t2.*t12.*t14;
t36 = t35-t66;
t37 = t8.*t36.*(9.0./2.5e2);
t38 = t7.*t19.*(9.0./1.25e2);
t39 = t4.*t5.*t14.*(9.0./1.25e2);
t42 = t14.*t22.*(1.0./1.0e2);
t65 = t13.*t34.*(9.0./2.5e2);
t40 = t24+t37+t38+t39-t42-t65;
t41 = t40.*pi.*3.6225e-1;
t43 = t5.*t14.*(1.51e2./1.0e3);
t45 = t4.*t31;
t46 = t5.*t7.*t16;
t47 = t45+t46;
t48 = t6.*t14;
t49 = t2.*t12.*t16;
t50 = t48+t49;
t51 = t8.*t50.*(9.0./2.5e2);
t52 = t7.*t31.*(9.0./1.25e2);
t55 = t5.*t16.*(1.51e2./5.0e2);
t58 = t13.*t47.*(9.0./2.5e2);
t59 = t4.*t5.*t16.*(9.0./1.25e2);
t53 = t32+t51+t52-t55-t58-t59;
t54 = t53.*pi.*3.6225e-1;
t62 = t5.*t16.*(1.51e2./1.0e3);
t56 = t32-t62;
t57 = t56.*pi.*6.07775;
t60 = t32-t55;
t61 = t60.*pi.*(1.61e2./2.56e2);
t63 = t54+t57+t61;
t67 = t23-t42;
t68 = t67.*pi.*1.40875;
t69 = t24-t42;
t70 = t69.*pi.*(1.61e2./2.56e2);
t71 = t42-t43;
t72 = t8.*t11.*6.694531704772773e-4;
t79 = t5.*t12.*t13.*6.694531704772773e-4;
t73 = t72-t79;
t74 = t11.*t13.*3.556381058634072e-4;
t75 = t5.*t8.*t12.*3.556381058634072e-4;
t76 = t74+t75;
t77 = t2.*t4.*6.694531704772773e-4;
t80 = t5.*t6.*t7.*6.694531704772773e-4;
t78 = t77-t80;
t81 = t2.*t4.*2.88132724657853e-3;
t89 = t5.*t6.*t7.*2.88132724657853e-3;
t82 = t81-t89;
t83 = t7.*t19;
t84 = t4.*t5.*t14;
t85 = t83+t84;
t86 = t2.*t7.*2.88132724657853e-3;
t87 = t4.*t5.*t6.*2.88132724657853e-3;
t88 = t86+t87;
t90 = t7.*t31;
t150 = t4.*t5.*t16;
t91 = t90-t150;
t92 = t15.*t16.*(2.7e1./1.0e2);
t93 = t29-t32+t92;
t94 = t2.*t14.*(1.51e2./5.0e2);
t95 = t5.*7.0;
t96 = t27.*2.7e1;
t97 = t95+t96;
t98 = t14.*t97.*(1.0./1.0e2);
t99 = t14.*t15.*(2.7e1./1.0e2);
t100 = t16.*t97.*(1.0./1.0e2);
t101 = t11.*t13.*(9.0./2.5e2);
t102 = t2.*t4.*(9.0./1.25e2);
t103 = t5.*t8.*t12.*(9.0./2.5e2);
t111 = t5.*t6.*t7.*(9.0./1.25e2);
t104 = t101+t102+t103-t111;
t105 = t2.*t16.*(1.51e2./5.0e2);
t106 = t100+t105;
t107 = t106.*pi.*(1.61e2./2.56e2);
t108 = t2.*t16.*(1.51e2./1.0e3);
t109 = t100+t108;
t110 = t109.*pi.*6.07775;
t112 = t16.*t104;
t113 = t100+t105+t112;
t114 = t113.*pi.*3.6225e-1;
t115 = t107+t110+t114;
t116 = t14.*t27.*(2.7e1./1.0e2);
t117 = t5.*t14.*(7.0./2.0e2);
t118 = t116+t117;
t119 = t118.*pi.*1.40875;
t120 = t14.*t104;
t121 = t94+t98+t120;
t122 = t121.*pi.*3.6225e-1;
t123 = t94+t98;
t124 = t123.*pi.*(1.61e2./2.56e2);
t125 = t2.*t14.*(1.51e2./1.0e3);
t126 = t98+t125;
t127 = t126.*pi.*6.07775;
t128 = t5.*t16.*(7.0./2.0e2);
t129 = t16.*t27.*(2.7e1./1.0e2);
t130 = t128+t129;
t131 = t130.*pi.*1.40875;
t132 = t107+t110+t114+t131;
t133 = t122+t124+t127;
t134 = t37+t38+t39-t65;
t135 = t119+t122+t124+t127;
t136 = t13.*t36;
t137 = t8.*t34;
t138 = t136+t137;
t139 = t8.*t36;
t213 = t13.*t34;
t140 = t139-t213;
t141 = t76.*t140;
t142 = t78.*t85;
t212 = t73.*t138;
t143 = t141+t142-t212;
t144 = t8.*t47;
t145 = t13.*t50;
t146 = t144+t145;
t147 = t8.*t50;
t218 = t13.*t47;
t148 = t147-t218;
t149 = t76.*t148;
t151 = t78.*t91;
t217 = t73.*t146;
t152 = t149+t151-t217;
t153 = t82.*t85;
t154 = t5.*t12.*t36.*6.174272671239708e-4;
t214 = t34.*t88;
t155 = t153+t154-t214;
t156 = t82.*t91;
t157 = t5.*t12.*t50.*6.174272671239708e-4;
t206 = t47.*t88;
t158 = t156+t157-t206;
t159 = t5.*t6.*t31.*1.570529909265897e-1;
t160 = t2.*t5.*t16.*2.386726843794421e-2;
t207 = t5.*t12.*t50.*1.570529909265897e-1;
t161 = t159+t160-t207;
t162 = t14.*t161;
t163 = t5.*t12.*t36.*1.570529909265897e-1;
t164 = t2.*t5.*t14.*2.386726843794421e-2;
t205 = t5.*t6.*t19.*1.570529909265897e-1;
t165 = t163+t164-t205;
t166 = t2.*1.51e2;
t167 = t5.*3.5e1;
t168 = t166+t167;
t169 = t23-t42+t99;
t170 = t14.*t168.*(1.0./5.0e2);
t171 = t120+t170;
t172 = t171.*pi.*3.6225e-1;
t173 = t5.*t14.*(7.0./1.0e2);
t174 = t125+t173;
t175 = t174.*pi.*6.07775;
t176 = t14.*t168.*pi.*1.2578125e-3;
t177 = t5.*t14.*pi.*4.930625e-2;
t178 = t172+t175+t176+t177;
t179 = t5.*t16.*(7.0./1.0e2);
t180 = t108+t179;
t181 = t180.*pi.*6.07775;
t182 = t16.*t168.*(1.0./5.0e2);
t183 = t112+t182;
t184 = t183.*pi.*3.6225e-1;
t185 = t16.*t168.*pi.*1.2578125e-3;
t186 = t5.*t16.*pi.*4.930625e-2;
t187 = t181+t184+t185+t186;
t188 = t172+t175+t176;
t189 = t181+t184+t185;
t190 = t11.*t88;
t192 = t26.*t82;
t193 = t12.^2;
t194 = t26.*t78;
t195 = t8.*t11;
t224 = t5.*t12.*t13;
t196 = t195-t224;
t197 = t73.*t196;
t198 = t11.*t13;
t199 = t5.*t8.*t12;
t200 = t198+t199;
t201 = t76.*t200;
t202 = t2.^2;
t203 = t6.^2;
t204 = t28.*t203.*1.570529909265897e-1;
t208 = t51+t52-t58-t59;
t209 = t2.*t208;
t210 = t5.*t16.*t104;
t211 = t209+t210;
t215 = t2.*t134;
t219 = t5.*t14.*t104;
t216 = t215-t219;
t220 = t28.*t193.*6.174272671239708e-4;
t221 = t190+t192+t220;
t222 = t36.*t104;
t228 = t5.*t12.*t134;
t223 = t222-t228;
t225 = t194+t197+t201;
t226 = t50.*t104;
t229 = t5.*t12.*t208;
t227 = t226-t229;
t230 = t26.*t134;
t235 = t85.*t104;
t231 = t230-t235;
t232 = t91.*t104;
t234 = t26.*t208;
t233 = t232-t234;
t236 = t29-t32;
t239 = t236.*pi.*1.40875;
t237 = t54+t57+t61-t239;
t238 = t54+t61;
t240 = t15.*t16.*pi.*1.6505015625;
t242 = t71.*pi.*6.07775;
t241 = t41+t68+t70-t242-t14.*t15.*pi.*1.6505015625;
t243 = t41+t68+t70-t242;
t244 = t41+t70-t242;
t245 = pi.*(t24-t42).*(1.61e2./2.56e2);
t246 = t41+t245;
t247 = t107+t114;
t248 = t16.*t27.*pi.*1.6505015625;
t249 = t107+t110+t114+t131+t248;
t250 = t7.*t19.*6.694531704772773e-4;
t251 = t4.*t5.*t14.*6.694531704772773e-4;
t252 = t250+t251;
t253 = t13.*t36.*6.694531704772773e-4;
t254 = t8.*t34.*6.694531704772773e-4;
t255 = t253+t254;
t256 = t8.*t36.*3.556381058634072e-4;
t257 = t6.*t16.*1.570529909265897e-1;
t279 = t2.*t12.*t14.*1.570529909265897e-1;
t258 = t257-t279;
t259 = t12.*t16.*1.570529909265897e-1;
t260 = t2.*t6.*t14.*1.570529909265897e-1;
t261 = t259+t260;
t262 = t14.^2;
t263 = t16.^2;
t264 = t15.^2;
t265 = t27.^2;
t266 = t15.*(2.7e1./1.0e2);
t267 = 1.550032257728851e2;
t268 = atan(1.51e2./3.5e1);
t269 = t268+th2+th3;
t270 = cos(t269);
t271 = t267.*t270.*(1.0./5.0e2);
t272 = t6.*t16.*6.174272671239708e-4;
t280 = t2.*t12.*t14.*6.174272671239708e-4;
t273 = t272-t280;
t274 = t7.*t19.*2.88132724657853e-3;
t275 = t4.*t5.*t14.*2.88132724657853e-3;
t276 = t274+t275;
t277 = t4.*t19.*2.88132724657853e-3;
t281 = t5.*t7.*t14.*2.88132724657853e-3;
t278 = t277-t281;
t282 = t2.*(7.0./1.0e2);
t290 = t5.*t262.*(1.51e2./1.0e3);
t291 = t5.*t263.*(1.51e2./1.0e3);
t283 = t266+t282-t290-t291;
t284 = t283.*pi.*6.07775;
t285 = t266+t271;
t286 = t285.*pi.*(1.61e2./2.56e2);
t287 = t14.*t169;
t288 = t16.*t93;
t289 = -t266+t287+t288;
t292 = t16.*(t51+t52-t58-t59);
t295 = t14.*t134;
t293 = t266+t271+t292-t295;
t294 = t293.*pi.*3.6225e-1;
t296 = -t51-t52+t58+t59;
t298 = t16.*t296;
t297 = t266+t271-t295-t298;
t299 = t297.*pi.*3.6225e-1;
t300 = t284+t286+t299;
t301 = t12.*t14.*1.570529909265897e-1;
t315 = t2.*t6.*t16.*1.570529909265897e-1;
t302 = t301-t315;
t303 = t6.*t14.*1.570529909265897e-1;
t304 = t2.*t12.*t16.*1.570529909265897e-1;
t305 = t303+t304;
t306 = t7.*t31.*6.694531704772773e-4;
t312 = t4.*t5.*t16.*6.694531704772773e-4;
t307 = t306-t312;
t308 = t8.*t47.*6.694531704772773e-4;
t309 = t13.*t50.*6.694531704772773e-4;
t310 = t308+t309;
t311 = t8.*t50.*3.556381058634072e-4;
t313 = t14.*t27.*pi.*1.6505015625;
t314 = t119+t122+t124+t127+t313;
t316 = t122+t124;
t317 = t14.*t16.*t202.*5.532148313430778e-3;
t318 = t14.*t16.*t28.*4.573242605769442e-3;
t367 = t14.*t16.*4.573242605769442e-3;
t319 = t317+t318-t367;
t320 = t6.*t14.*6.174272671239708e-4;
t321 = t2.*t12.*t16.*6.174272671239708e-4;
t322 = t320+t321;
t323 = t7.*t31.*2.88132724657853e-3;
t331 = t4.*t5.*t16.*2.88132724657853e-3;
t324 = t323-t331;
t325 = t4.*t31.*2.88132724657853e-3;
t326 = t5.*t7.*t16.*2.88132724657853e-3;
t327 = t325+t326;
t328 = t14.*t16.*t264.*1.080250746560099e-1;
t329 = t14.*t16.*t265.*2.873466985849863e-1;
t330 = t328+t329-t14.*t16.*2.873466985849863e-1;
t332 = t286+t299;
t333 = t15.*t262.*(2.7e1./2.0e2);
t334 = t15.*t263.*(2.7e1./2.0e2);
t335 = t333+t334;
t336 = t335.*pi.*1.22259375e1;
t474 = t289.*pi.*1.40875;
t337 = t284+t286+t299-t474;
t338 = t184+t185;
t339 = t85.*t252;
t340 = t138.*t255;
t355 = t13.*t34.*3.556381058634072e-4;
t430 = t256-t355;
t341 = t430.*(t139-t213);
t342 = t339+t340+t341;
t343 = t16.*t342;
t344 = t50.*t258;
t345 = t31.*t261;
t385 = t14.*t16.*t28.*2.386726843794421e-2;
t346 = t344+t345-t385;
t347 = t14.*t346;
t348 = t263.*4.573242605769442e-3;
t349 = t202.*t262.*5.532148313430778e-3;
t350 = t28.*t262.*4.573242605769442e-3;
t351 = t348+t349+t350;
t352 = t16.*t351;
t353 = t91.*t252;
t354 = t146.*t255;
t356 = t5.*(1.51e2./5.0e2);
t357 = t36.*t273;
t358 = t85.*t276;
t359 = t34.*t278;
t360 = t357+t358+t359;
t361 = t16.*t360;
t362 = t28.*t262.*2.386726843794421e-2;
t363 = t19.*t261;
t364 = t36.*t258;
t365 = t362+t363+t364;
t366 = t16.*t365;
t368 = t50.*t273;
t369 = t47.*t278;
t370 = t91.*t276;
t371 = t368+t369+t370;
t372 = t14.*t371;
t373 = t282-t356;
t374 = -t282+t295+t298+t356;
t375 = t374.*pi.*3.6225e-1;
t376 = -t282+t290+t291;
t377 = t376.*pi.*6.07775;
t381 = t373.*pi.*(1.61e2./2.56e2);
t378 = t375+t377-t381;
t379 = t287+t288;
t380 = t379.*pi.*1.40875;
t382 = t375+t377+t380-t381;
t383 = t19.*t302;
t384 = t36.*t305;
t386 = t262.*4.573242605769442e-3;
t387 = t202.*t263.*5.532148313430778e-3;
t388 = t28.*t263.*4.573242605769442e-3;
t389 = t386+t387+t388;
t390 = t14.*t389;
t391 = t85.*t307;
t392 = t138.*t310;
t398 = t13.*t47.*3.556381058634072e-4;
t416 = t311-t398;
t393 = t416.*(t139-t213);
t394 = t391+t392+t393;
t395 = t16.*t394;
t396 = t91.*t307;
t397 = t146.*t310;
t399 = t28.*t263.*2.386726843794421e-2;
t400 = t50.*t305;
t401 = t31.*t302;
t402 = t399+t400+t401;
t403 = t14.*t402;
t404 = t172+t176;
t405 = t36.*t322;
t406 = t85.*t324;
t407 = t34.*t327;
t408 = t405+t406+t407;
t409 = t16.*t408;
t410 = t50.*t322;
t411 = t47.*t327;
t412 = t91.*t324;
t413 = t410+t411+t412;
t414 = t14.*t413;
t415 = t196.*t310;
t417 = t5.*t6.*t302;
t418 = t11.*t327;
t419 = (t147-t218).*(t311-t398);
t420 = t396+t397+t419;
t422 = t2.*t296;
t421 = t210-t422;
t423 = t5.*t16.*t134;
t426 = t5.*t14.*t296;
t424 = t423-t426;
t425 = t383+t384-t385;
t427 = t5.*t6.*t261;
t428 = t11.*t278;
t429 = t196.*t255;
t431 = (t147-t218).*(t256-t355);
t432 = t353+t354+t431;
t433 = t5.*t12.*t296;
t434 = t226+t433;
t435 = t36.*t296;
t436 = t50.*t134;
t437 = t435+t436;
t438 = t26.*t324;
t439 = t5.*t12.*t322;
t440 = -t418+t438+t439;
t441 = t200.*t416;
t442 = t26.*t307;
t443 = t26.*t276;
t444 = t5.*t12.*t273;
t445 = -t428+t443+t444;
t446 = t200.*t430;
t447 = t26.*t252;
t448 = (t139-t213).*(t311-t398);
t449 = t391+t392+t448;
t450 = t26.*t296;
t451 = t232+t450;
t452 = t91.*t134;
t453 = t85.*t296;
t454 = t452+t453;
t455 = (t139-t213).*(t256-t355);
t456 = t339+t340+t455;
t457 = t5.*t243.*(7.0./2.0e2);
t458 = t2.*t244.*(1.51e2./1.0e3);
t459 = t5.*t244.*(7.0./2.0e2);
t460 = t2.*t246.*(1.51e2./1.0e3);
t461 = t40.*t104.*pi.*3.6225e-1;
t462 = t5.*t12.*t258;
t463 = t5.*t237.*(7.0./2.0e2);
t464 = t2.*t63.*(1.51e2./1.0e3);
t465 = t2.*t238.*(1.51e2./1.0e3);
t466 = t5.*t63.*(7.0./2.0e2);
t467 = t53.*t104.*pi.*3.6225e-1;
t468 = t2.*t5.*t16.*2.290836273028288e-2;
t469 = t2.*t247.*(1.51e2./1.0e3);
t470 = t2.*t115.*(1.51e2./1.0e3);
t471 = t5.*t115.*(7.0./2.0e2);
t472 = t14.*t432;
t473 = t5.*t132.*(7.0./2.0e2);
t475 = t104.*t113.*pi.*3.6225e-1;
t476 = t2.*t16.*t300.*(7.0./2.0e2);
t477 = t16.*t425;
t478 = t14.*t420;
t479 = t2.*t133.*(1.51e2./1.0e3);
t480 = t5.*t133.*(7.0./2.0e2);
t481 = t2.*t316.*(1.51e2./1.0e3);
t482 = t5.*t135.*(7.0./2.0e2);
t483 = t2.*t14.*t300.*(7.0./2.0e2);
t484 = t104.*t121.*pi.*3.6225e-1;
t485 = t5.*t178.*(7.0./2.0e2);
t486 = t169.*t382;
t487 = t16.*t449;
t488 = t2.*t188.*(1.51e2./1.0e3);
t489 = t5.*t188.*(7.0./2.0e2);
t490 = t2.*t404.*(1.51e2./1.0e3);
t491 = t134.*t374.*pi.*3.6225e-1;
t492 = t5.*t14.*t378.*(1.51e2./1.0e3);
t493 = t104.*t171.*pi.*3.6225e-1;
t494 = t5.*t14.*(t375-t381).*(1.51e2./1.0e3);
t495 = t2.*t338.*(1.51e2./1.0e3);
t496 = t2.*t189.*(1.51e2./1.0e3);
t497 = t5.*t189.*(7.0./2.0e2);
t498 = t16.*t456;
t499 = t5.*t187.*(7.0./2.0e2);
t500 = t296.*t374.*pi.*3.6225e-1;
t501 = t5.*t16.*t378.*(1.51e2./1.0e3);
t502 = t104.*t183.*pi.*3.6225e-1;
t503 = t5.*t16.*(t375-t381).*(1.51e2./1.0e3);
t504 = t164-t427+t462;
t505 = -t429+t446+t447;
t506 = t104.*t216.*pi.*3.6225e-1;
t507 = t5.*t16.*t346;
t508 = t5.*t16.*t432;
t509 = t2.*t216.*pi.*1.093995e-1;
t510 = t5.*t216.*pi.*2.53575e-2;
t511 = t5.*t16.*t371;
t512 = t93.*t424.*pi.*3.6225e-1;
t513 = t296.*t424.*pi.*3.6225e-1;
t514 = t5.*t16.*t424.*pi.*1.093995e-1;
t515 = -t415+t441+t442;
t566 = t5.*t12.*t305;
t516 = t160+t417-t566;
t517 = t2.*t516;
t518 = t5.*t16.*t420;
t519 = t5.*t16.*t402;
t520 = t5.*t16.*t413;
t521 = t169.*t424.*pi.*3.6225e-1;
t522 = t134.*t424.*pi.*3.6225e-1;
t523 = t5.*t14.*t424.*pi.*1.093995e-1;
t524 = t2.*t421.*pi.*1.093995e-1;
t525 = t5.*t421.*pi.*2.53575e-2;
t526 = t104.*t421.*pi.*3.6225e-1;
t527 = t36.*t408;
t528 = t50.*t413;
t529 = t36.*t449;
t530 = t50.*t420;
t531 = t2.*t434.*pi.*1.093995e-1;
t532 = t169.*t437.*pi.*3.6225e-1;
t533 = t5.*t434.*pi.*2.53575e-2;
t534 = t134.*t437.*pi.*3.6225e-1;
t535 = t5.*t12.*t440;
t536 = t104.*t434.*pi.*3.6225e-1;
t537 = t5.*t14.*t437.*pi.*1.093995e-1;
t538 = t36.*t360;
t539 = t50.*t371;
t540 = t36.*t456;
t541 = t50.*t432;
t542 = t2.*t223.*pi.*1.093995e-1;
t543 = t5.*t223.*pi.*2.53575e-2;
t544 = t93.*t437.*pi.*3.6225e-1;
t545 = t296.*t437.*pi.*3.6225e-1;
t546 = t5.*t12.*t445;
t547 = t104.*t223.*pi.*3.6225e-1;
t548 = t5.*t16.*t437.*pi.*1.093995e-1;
t549 = t85.*t449;
t550 = t91.*t420;
t551 = t169.*t454.*pi.*3.6225e-1;
t552 = t2.*t451.*pi.*1.093995e-1;
t553 = t5.*t451.*pi.*2.53575e-2;
t554 = t134.*t454.*pi.*3.6225e-1;
t555 = t104.*t451.*pi.*3.6225e-1;
t556 = t5.*t14.*t454.*pi.*1.093995e-1;
t557 = t85.*t456;
t558 = t91.*t432;
t559 = t93.*t454.*pi.*3.6225e-1;
t560 = t296.*t454.*pi.*3.6225e-1;
t561 = t5.*t16.*t454.*pi.*1.093995e-1;
t562 = t202.*2.386726843794421e-2;
t563 = t28.*t193.*1.576704181937136e-1;
t564 = t5.*t14.*t246.*(1.51e2./1.0e3);
t565 = t40.*t134.*pi.*3.6225e-1;
t567 = t5.*t14.*t247.*(1.51e2./1.0e3);
t568 = t5.*t14.*t115.*(1.51e2./1.0e3);
t569 = t113.*t134.*pi.*3.6225e-1;
t570 = t16.*t143;
t571 = t14.*t152;
t572 = t16.*t155;
t573 = t14.*t158;
t574 = t16.*t165;
t575 = t134.*t183.*pi.*3.6225e-1;
t576 = t5.*t14.*t338.*(1.51e2./1.0e3);
t577 = t5.*t14.*t189.*(1.51e2./1.0e3);
t578 = t28.*t193.*1.570529909265897e-1;
t579 = t204+t562+t578;
t580 = t5.*t16.*t158;
t581 = t134.*t223.*pi.*3.6225e-1;
t582 = t5.*t14.*t223.*pi.*1.093995e-1;
t583 = t5.*t12.*(-t429+t446+t447);
t584 = t5.*t12.*(-t415+t441+t442);
t585 = t26.*(-t415+t441+t442);
t586 = t26.*(-t429+t446+t447);
t587 = t121.*t296.*pi.*3.6225e-1;
t588 = t171.*t296.*pi.*3.6225e-1;
t589 = t104.*pi.*(t210-t422).*3.6225e-1;
t590 = t2.*t221;
t591 = t2.*t225;
t592 = t5.*t14.*(t141+t142-t212);
t593 = t5.*t14.*t155;
t594 = t134.*t216.*pi.*3.6225e-1;
t595 = t36.*(t141+t142-t212);
t596 = t36.*t155;
t597 = t50.*(t149+t151-t217);
t598 = t50.*t158;
t599 = t5.*t12.*t221;
t600 = t5.*t12.*t225;
t601 = t296.*t434.*pi.*3.6225e-1;
t602 = t26.*t225;
t603 = t91.*t152;
t604 = t85.*t143;
t605 = t134.*t231.*pi.*3.6225e-1;
t606 = t296.*t451.*pi.*3.6225e-1;
t607 = t549+t550+t554+t555+t585;
t608 = t557+t558+t560+t586-t104.*t231.*pi.*3.6225e-1;
M = reshape([t28.*5.532148313430778e-3+t190+t192+t194+t197+t201+t202.*2.844051104371366e-2+t204+t264.*2.873466985849863e-1+t265.*1.080250746560099e-1+t563+t564+t565+pi.*1.16725e-1-t93.*(t54+t57-t236.*pi.*1.40875+pi.*(t32-t5.*t16.*(1.51e2./5.0e2)).*(1.61e2./2.56e2))+(t23+t99-t14.*t22.*(1.0./1.0e2)).*(t41+pi.*(t23-t14.*t22.*(1.0./1.0e2)).*1.40875+pi.*(t24-t14.*t22.*(1.0./1.0e2)).*(1.61e2./2.56e2)+pi.*(t43-t14.*t22.*(1.0./1.0e2)).*6.07775)-t14.*t15.*(t41+t68+t70-t71.*pi.*6.07775).*(2.7e1./2.0e2)+t208.*pi.*(t32+t51+t52-t55-t58-t59).*3.6225e-1+t15.*t16.*(t54+t57+t61+t240-t236.*pi.*1.40875).*(2.7e1./2.0e2)-t2.*t14.*(t41+t70-t71.*pi.*6.07775).*(7.0./2.0e2)+t5.*t14.*(t41+t70-t71.*pi.*6.07775).*(1.51e2./1.0e3)+t2.*t16.*t63.*(7.0./2.0e2)-t5.*t16.*t63.*(1.51e2./1.0e3)-t5.*t16.*t238.*(1.51e2./1.0e3)+t15.*t16.*t237.*(2.7e1./2.0e2)-t14.*t15.*t241.*(2.7e1./2.0e2),t16.*(t427+t428+t429+t457+t458+t459+t460+t461+t27.*t241.*(2.7e1./2.0e2)+t27.*t243.*(2.7e1./2.0e2)-t26.*t252-t26.*t276-t200.*(t256-t13.*t34.*3.556381058634072e-4)-t2.*t5.*t14.*2.290836273028288e-2-t14.*t15.*t27.*1.793216239289764e-1-t5.*t12.*t258-t5.*t12.*t273)+t14.*(t415+t417+t418+t463+t464+t465+t466+t467+t468+t27.*t237.*(2.7e1./2.0e2)-t26.*t307-t26.*t324-t200.*(t311-t13.*t47.*3.556381058634072e-4)+t27.*(t54+t57+t61-t239+t240).*(2.7e1./2.0e2)+t15.*t16.*t27.*1.793216239289764e-1-t5.*t12.*t305-t5.*t12.*t322),t16.*(t427+t428+t429-t443-t444-t447+t457+t458+t459+t460+t461-t462-t200.*(t256-t355)-t2.*t5.*t14.*2.290836273028288e-2)+t14.*(t415+t417+t418-t438-t439-t442+t463+t464+t465+t466+t467+t468-t200.*(t311-t398)-t5.*t12.*t305),-t2.*(t190+t192+t194+t197+t201+t204+t562+t563+t564+t565-t53.*t296.*pi.*3.6225e-1-t5.*t16.*t63.*(1.51e2./1.0e3)-t5.*t16.*t238.*(1.51e2./1.0e3)+t5.*t14.*t244.*(1.51e2./1.0e3))-t5.*t14.*(t164-t427-t428-t429+t443+t444+t446+t447-t458-t460-t461+t462)-t5.*t16.*(t160+t415+t417+t418-t438-t439-t441-t442+t464+t465+t467-t566),-t50.*(-t415-t418+t438+t439+t441+t442-t467)-t36.*(-t428-t429+t443+t444+t446+t447-t461)-t5.*t12.*(t190+t192+t194+t197+t201+t220+t565-t53.*t296.*pi.*3.6225e-1),-t26.*(t194+t197+t201+t565-t53.*t296.*pi.*3.6225e-1)+t91.*(t415-t441-t442+t104.*pi.*(t32+t51+t52-t55-t58-t59).*3.6225e-1)+t85.*(t429-t446-t447+t461),t162+t567+t568+t569-t16.*t143-t14.*t152-t16.*t155-t14.*t158-t16.*t165-t93.*t135+t132.*t169+t121.*t208.*pi.*3.6225e-1-t2.*t14.*t115.*(7.0./2.0e2)+t2.*t16.*t133.*(7.0./2.0e2)-t5.*t16.*t133.*(1.51e2./1.0e3)-t14.*t15.*t132.*(2.7e1./2.0e2)+t15.*t16.*t135.*(2.7e1./2.0e2)-t14.*t15.*t249.*(2.7e1./2.0e2)-t5.*t16.*t316.*(1.51e2./1.0e3)+t15.*t16.*t314.*(2.7e1./2.0e2),t16.*(t343+t347+t352+t361+t366+t372+t469+t470+t471+t473+t475+t476+t16.*(t263.*2.873466985849863e-1+t262.*t264.*1.080250746560099e-1+t262.*t265.*2.873466985849863e-1)+t27.*t132.*(2.7e1./2.0e2)+t27.*t249.*(2.7e1./2.0e2)-t14.*t319-t14.*t330-t93.*(t284+t286-t289.*pi.*1.40875+pi.*(t266+t271-t14.*t134+t16.*t208).*3.6225e-1)+t14.*(t353+t354+(t147-t218).*(t256-t13.*t34.*3.556381058634072e-4))+t15.*t16.*(t284+t286+t294-t289.*pi.*1.40875).*(2.7e1./2.0e2)-t296.*t297.*pi.*3.6225e-1+t15.*t16.*(t284+t286+t294+t336-t289.*pi.*1.40875).*(2.7e1./2.0e2)-t5.*t16.*t300.*(1.51e2./1.0e3)-t5.*t16.*t332.*(1.51e2./1.0e3))+t14.*(t390+t395+t403+t409+t414+t479+t480+t481+t482+t483+t484+t14.*(t262.*2.873466985849863e-1+t263.*t264.*1.080250746560099e-1+t263.*t265.*2.873466985849863e-1)+t27.*t135.*(2.7e1./2.0e2)-t16.*t319+t27.*t314.*(2.7e1./2.0e2)-t16.*t330-t169.*t337+t16.*(t383+t384-t14.*t16.*t28.*2.386726843794421e-2)+t14.*(t396+t397+(t147-t218).*(t311-t13.*t47.*3.556381058634072e-4))-t134.*t297.*pi.*3.6225e-1+t14.*t15.*(t284+t286+t299+t336-t289.*pi.*1.40875).*(2.7e1./2.0e2)-t5.*t14.*t300.*(1.51e2./1.0e3)-t5.*t14.*t332.*(1.51e2./1.0e3)+t14.*t15.*t337.*(2.7e1./2.0e2)),t16.*(t347+t352+t361+t366+t372+t469+t470+t471+t472+t473+t475+t476+t498-t14.*t319-t93.*t337-t296.*t297.*pi.*3.6225e-1-t5.*t16.*t300.*(1.51e2./1.0e3)-t5.*t16.*t332.*(1.51e2./1.0e3))+t14.*(t390+t403+t409+t414+t477+t478+t479+t480+t481+t482+t483+t484+t487-t16.*t319-t169.*t337-t134.*t297.*pi.*3.6225e-1-t5.*t14.*t300.*(1.51e2./1.0e3)-t5.*t14.*t332.*(1.51e2./1.0e3)),t2.*(-t162-t567-t568-t569+t570+t571+t572+t573+t574+t587+t5.*t16.*t133.*(1.51e2./1.0e3)+t5.*t16.*t316.*(1.51e2./1.0e3))+t5.*t14.*(t347+t361+t366+t372+t469+t470+t472+t475+t498-t296.*t297.*pi.*3.6225e-1-t5.*t16.*t300.*(1.51e2./1.0e3)-t5.*t16.*t332.*(1.51e2./1.0e3))-t5.*t16.*(t403+t409+t414+t477+t478+t479+t481+t484+t487-t134.*t297.*pi.*3.6225e-1-t5.*t14.*t300.*(1.51e2./1.0e3)-t5.*t14.*t332.*(1.51e2./1.0e3)),t50.*(t409+t414+t478+t484+t487-t134.*t297.*pi.*3.6225e-1)+t36.*(t361+t372+t472+t475+t498-t296.*t297.*pi.*3.6225e-1)+t5.*t12.*(-t569+t570+t571+t572+t573+t587),t91.*(t478+t484+t487-t134.*t297.*pi.*3.6225e-1)+t85.*(t472+t475+t498-t296.*t297.*pi.*3.6225e-1)+t26.*(-t569+t570+t571+t587),t162+t575+t576+t577-t16.*t143-t14.*t152-t16.*t155-t14.*t158-t16.*t165-t93.*t178+t169.*t187+t171.*t208.*pi.*3.6225e-1-t2.*t14.*t189.*(7.0./2.0e2)+t2.*t16.*t188.*(7.0./2.0e2)-t5.*t16.*t188.*(1.51e2./1.0e3)+t15.*t16.*t178.*(2.7e1./1.0e2)-t14.*t15.*t187.*(2.7e1./1.0e2)-t5.*t16.*t404.*(1.51e2./1.0e3),t14.*(t390+t395+t403+t409+t414+t477+t478+t485+t486+t488+t489+t490+t491+t492+t493+t494+t27.*t178.*(2.7e1./1.0e2)-t16.*t319-t2.*t14.*t378.*(7.0./2.0e2)-t14.*t15.*t382.*(2.7e1./1.0e2))+t16.*(t343+t347+t352+t361+t366+t372+t472+t495+t496+t497+t499+t500+t501+t502+t503+t27.*t187.*(2.7e1./1.0e2)-t14.*t319+t93.*(t375+t377+t380-t373.*pi.*(1.61e2./2.56e2))-t2.*t16.*t378.*(7.0./2.0e2)-t15.*t16.*t382.*(2.7e1./1.0e2)),t16.*(t347+t352+t361+t366+t372+t472+t495+t496+t497+t498+t499+t500+t501+t502+t503-t14.*t319+t93.*t382-t2.*t16.*t378.*(7.0./2.0e2))+t14.*(t390+t403+t409+t414+t477+t478+t485+t486+t487+t488+t489+t490+t491+t492+t493+t494-t16.*t319-t2.*t14.*t378.*(7.0./2.0e2)),t2.*(-t162+t570+t571+t572+t573+t574-t575-t576-t577+t588+t5.*t16.*t188.*(1.51e2./1.0e3)+t5.*t16.*t404.*(1.51e2./1.0e3))+t5.*t14.*(t347+t361+t366+t372+t472+t495+t496+t498+t500+t501+t502+t503)-t5.*t16.*(t403+t409+t414+t477+t478+t487+t488+t490+t491+t492+t493+t494),t36.*(t361+t372+t472+t498+t500+t502)+t50.*(t409+t414+t478+t487+t491+t493)+t5.*t12.*(t570+t571+t572+t573-t575+t588),t91.*(t478+t487+t491+t493)+t85.*(t472+t498+t500+t502)+t26.*(t570+t571-t575+t588),t580-t2.*t221-t2.*t225-t2.*t579+t5.*t16.*(t149+t151-t217)+t93.*t211.*pi.*3.6225e-1-t134.*t216.*pi.*3.6225e-1-t169.*t216.*pi.*3.6225e-1-t208.*t211.*pi.*3.6225e-1-t5.*t14.*t143-t5.*t14.*t155-t5.*t16.*t161-t5.*t14.*t165-t2.*t16.*t211.*pi.*1.267875e-2+t2.*t14.*t216.*pi.*1.267875e-2-t5.*t14.*t216.*pi.*1.093995e-1-t15.*t16.*t211.*pi.*9.78075e-2+t14.*t15.*t216.*pi.*9.78075e-2+t5.*t16.*pi.*(t209+t210).*1.093995e-1,-t16.*(t506+t507+t508+t509+t510+t511+t512+t513+t514-t2.*t445-t2.*t504-t2.*t505+t27.*t216.*pi.*9.78075e-2-t5.*t14.*t360-t5.*t14.*t365-t5.*t14.*(t339+t340+t140.*t430)-t2.*t16.*t424.*pi.*1.267875e-2-t15.*t16.*t424.*pi.*9.78075e-2)-t14.*(t517+t518+t519+t520+t521+t522+t523+t524+t525+t526-t2.*t440-t2.*t515+t27.*t421.*pi.*9.78075e-2-t5.*t14.*t408-t5.*t14.*t425-t5.*t14.*(t391+t392+t140.*t416)-t2.*t14.*t424.*pi.*1.267875e-2-t14.*t15.*t424.*pi.*9.78075e-2),-t16.*(t506+t507+t508+t509+t510+t511+t512+t513+t514-t2.*t445-t2.*t504-t2.*t505-t5.*t14.*t360-t5.*t14.*t365-t5.*t14.*t456-t2.*t16.*t424.*pi.*1.267875e-2)-t14.*(t517+t518+t519+t520+t521+t522+t523+t524+t525+t526-t2.*t440-t2.*t515-t5.*t14.*t408-t5.*t14.*t425-t5.*t14.*t449-t2.*t14.*t424.*pi.*1.267875e-2),t2.*(-t580+t590+t591+t592+t593+t594+t2.*t579-t296.*t421.*pi.*3.6225e-1-t5.*t16.*t152+t5.*t16.*t161+t5.*t14.*t165+t5.*t14.*t216.*pi.*1.093995e-1-t5.*t16.*t421.*pi.*1.093995e-1)+t5.*t16.*(t517+t518+t519+t520+t522+t523+t589-t2.*t440-t2.*t515-t5.*t14.*t408-t5.*t14.*t425-t5.*t14.*t449+t2.*pi.*(t210-t422).*1.093995e-1)-t5.*t14.*(t506+t507+t508+t509+t511+t513+t514-t2.*t445-t2.*t504-t2.*t505-t5.*t14.*t360-t5.*t14.*t365-t5.*t14.*t456),-t36.*(t506+t508+t511+t513-t2.*t445-t2.*t505-t5.*t14.*t360-t5.*t14.*t456)-t50.*(t518+t520+t522+t589-t2.*t440-t2.*t515-t5.*t14.*t408-t5.*t14.*t449)+t5.*t12.*(-t580+t590+t591+t592+t593+t594-t296.*t421.*pi.*3.6225e-1-t5.*t16.*t152),-t85.*(t506+t508+t513-t2.*t505-t5.*t14.*t456)-t91.*(t518+t522+t589-t2.*t515-t5.*t14.*t449)+t26.*(t591+t592+t594-t296.*t421.*pi.*3.6225e-1-t5.*t16.*t152),t581+t582-t36.*t143-t36.*t155-t50.*t152-t50.*t158+t227.*pi.*(t51+t52-t58-t59).*3.6225e-1-t93.*t227.*pi.*3.6225e-1+t169.*t223.*pi.*3.6225e-1-t5.*t12.*t221-t5.*t12.*t225-t2.*t14.*t223.*pi.*1.267875e-2+t2.*t16.*t227.*pi.*1.267875e-2-t5.*t16.*t227.*pi.*1.093995e-1-t14.*t15.*t223.*pi.*9.78075e-2+t15.*t16.*t227.*pi.*9.78075e-2,t16.*(t538+t539+t540+t541+t542+t543+t544+t545+t546+t547+t548+t27.*t223.*pi.*9.78075e-2+t5.*t12.*t505-t2.*t16.*t437.*pi.*1.267875e-2-t15.*t16.*t437.*pi.*9.78075e-2)+t14.*(t527+t528+t529+t530+t531+t532+t533+t534+t535+t536+t537+t27.*t434.*pi.*9.78075e-2+t5.*t12.*t515-t2.*t14.*t437.*pi.*1.267875e-2-t14.*t15.*t437.*pi.*9.78075e-2),t14.*(t527+t528+t529+t530+t531+t532+t533+t534+t535+t536+t537+t584-t2.*t14.*t437.*pi.*1.267875e-2)+t16.*(t538+t539+t540+t541+t542+t543+t544+t545+t546+t547+t548+t583-t2.*t16.*t437.*pi.*1.267875e-2),t2.*(-t581-t582+t595+t596+t597+t598+t599+t600+t601+t5.*t16.*t434.*pi.*1.093995e-1)-t5.*t16.*(t527+t528+t529+t530+t531+t534+t535+t536+t537+t584)+t5.*t14.*(t538+t539+t540+t541+t542+t545+t546+t547+t548+t583),t50.*(t527+t528+t529+t530+t534+t535+t536+t584)+t36.*(t538+t539+t540+t541+t545+t546+t547+t583)+t5.*t12.*(-t581+t595+t596+t597+t598+t599+t600+t601),t91.*(t529+t530+t534+t536+t584)+t85.*(t540+t541+t545+t547+t583)+t26.*(-t581+t600+t601+t36.*t143+t50.*t152),-t85.*t143-t91.*t152-t26.*t225+t233.*pi.*(t51+t52-t58-t59).*3.6225e-1-t93.*t233.*pi.*3.6225e-1-t134.*t231.*pi.*3.6225e-1-t169.*t231.*pi.*3.6225e-1-t5.*t14.*t231.*pi.*1.093995e-1+t2.*t16.*t233.*pi.*1.267875e-2-t5.*t16.*t233.*pi.*1.093995e-1+t15.*t16.*t233.*pi.*9.78075e-2+t2.*t14.*pi.*(t230-t235).*1.267875e-2+t14.*t15.*pi.*(t230-t235).*9.78075e-2,t16.*(t557+t558+t559+t560+t561+t26.*t505-t2.*t231.*pi.*1.093995e-1-t5.*t231.*pi.*2.53575e-2-t27.*t231.*pi.*9.78075e-2-t104.*t231.*pi.*3.6225e-1-t2.*t16.*t454.*pi.*1.267875e-2-t15.*t16.*t454.*pi.*9.78075e-2)+t14.*(t549+t550+t551+t552+t553+t554+t555+t556+t26.*t515+t27.*t451.*pi.*9.78075e-2-t2.*t14.*t454.*pi.*1.267875e-2-t14.*t15.*t454.*pi.*9.78075e-2),t14.*(t549+t550+t551+t552+t553+t554+t555+t556+t585-t2.*t14.*t454.*pi.*1.267875e-2)+t16.*(t557+t558+t559+t560+t561+t586-t2.*t231.*pi.*1.093995e-1-t5.*t231.*pi.*2.53575e-2-t104.*t231.*pi.*3.6225e-1-t2.*t16.*t454.*pi.*1.267875e-2),t2.*(t602+t603+t604+t605+t606+t5.*t14.*t231.*pi.*1.093995e-1+t5.*t16.*t451.*pi.*1.093995e-1)+t5.*t14.*(t557+t558+t560+t561+t586-t2.*t231.*pi.*1.093995e-1-t104.*t231.*pi.*3.6225e-1)-t5.*t16.*(t549+t550+t552+t554+t555+t556+t585),t36.*t608+t50.*t607+t5.*t12.*(t602+t603+t604+t605+t606),t85.*t608+t91.*t607+t26.*(t602+t603+t604+t605+t606)],[6,6]);
end

function M = M_mat_diff(th1,th2,th3,th4,th5,th6)
%M_MAT_DIFF
%    M = M_MAT_DIFF(TH1,TH2,TH3,TH4,TH5,TH6)

%    This function was generated by the Symbolic Math Toolbox version 7.0.
%    21-Nov-2018 16:46:40

t2 = th2+th3;
t3 = cos(t2);
t4 = sin(th5);
t5 = sin(t2);
t6 = cos(th4);
t7 = cos(th5);
t8 = sin(th1);
t9 = sin(th4);
t10 = t8.*t9;
t11 = cos(th1);
t12 = t3.*t6.*t11;
t13 = t10+t12;
t14 = sin(th6);
t15 = t6.*t8;
t40 = t3.*t9.*t11;
t16 = t15-t40;
t17 = cos(th6);
t18 = t7.*t13;
t39 = t4.*t5.*t11;
t19 = t18-t39;
t20 = cos(th2);
t21 = t9.*t11;
t26 = t3.*t6.*t8;
t22 = t21-t26;
t23 = t7.*t22;
t24 = t4.*t5.*t8;
t25 = t23+t24;
t27 = t6.*t11;
t28 = t3.*t8.*t9;
t29 = t27+t28;
t30 = sin(th2);
t31 = sin(th3);
t32 = cos(th3);
t33 = t17.*t25.*1.2484505755283e-3;
t34 = t7.*t22.*2.409929378080134e-3;
t35 = t17.*t29.*3.850433196866315e-2;
t36 = t4.*t22.*8.028971461054102e-2;
t37 = t14.*t29.*1.2484505755283e-3;
t38 = t4.*t5.*t8.*2.409929378080134e-3;
t41 = t16.*t17.*3.850433196866315e-2;
t42 = t14.*t16.*1.2484505755283e-3;
t43 = t17.*t19.*1.2484505755283e-3;
t44 = t6.*t8.*6.84614609275178e-2;
t45 = t7.*t13.*2.409929378080134e-3;
t46 = t4.*t13.*8.028971461054102e-2;
t47 = t5.*t7.*t11.*8.028971461054102e-2;
t48 = t5.*t8.*4.915167130564437e-3;
t49 = t3.*t8.*3.689996292735745e-2;
t50 = t6.*t11.*6.84614609275178e-2;
t51 = t3.*t6.*t8.*2.272477191789019e-2;
t52 = t3.*t8.*t9.*6.84614609275178e-2;
t53 = t8.*t20.*t32.*1.85449568806793;
t54 = t11.*t30.*3.219519910626345e-4;
t55 = t3.*t11.*1.618000866946239e-1;
t56 = t5.*t11.*3.813159268614815;
t57 = t11.*t30.*t31.*1.85449568806793;
t58 = t11.*1.25890039900759e-2;
t59 = t8.*8.018329442092692e-2;
t63 = t14.*t19.*3.850433196866315e-2;
t64 = t8.*t9.*2.272477191789019e-2;
t65 = t3.*t6.*t11.*2.272477191789019e-2;
t66 = t3.*t9.*t11.*6.84614609275178e-2;
t67 = t4.*t5.*t11.*2.409929378080134e-3;
t68 = t11.*t20.*t32.*1.85449568806793;
t83 = t11.*t20.*1.247534853861598e1;
t84 = t11.*t30.*1.227529861371644e-2;
t60 = t41+t42+t43+t44+t45+t46+t47+t55+t56+t57+t58+t59-t63-t64-t65-t66-t67-t68-t83-t84;
t61 = t11.*5.164630050170653e-3;
t62 = t8.*6.271590127205854e-2;
t69 = t3.*t4;
t70 = t5.*t6.*t7;
t71 = t69+t70;
t72 = t3.*t7;
t392 = t4.*t5.*t6;
t73 = t72-t392;
t74 = t11.*5.391415465873457e-3;
t75 = t6.*t11.*3.104999007011269e-3;
t76 = t8.*t20.*8.455164471901305e-1;
t77 = t9.*t11.*1.865719029901695e-3;
t78 = t3.*t8.*t9.*3.104999007011269e-3;
t79 = t8.*t20.*t32.*2.191879307959464e-1;
t88 = t14.*t25.*3.850433196866315e-2;
t115 = t5.*t7.*t8.*8.028971461054102e-2;
t443 = t8.*6.104217881481557e-4;
t444 = t5.*t8.*9.450145625450081e-1;
t445 = t8.*t30.*t31.*2.191879307959464e-1;
t446 = t3.*t6.*t8.*1.865719029901695e-3;
t80 = t33+t34+t35+t36+t37+t38+t74+t75+t76+t77+t78+t79-t88-t115-t443-t444-t445-t446;
t81 = t3.*t9.*t11.*3.439231171461361e-3;
t82 = t8.*3.038635549296489e-3;
t85 = t5.*t7.*t8.*2.061478095729509e-3;
t86 = t11.*1.960554684600962e-3;
t87 = t6.*t11.*2.265025256144936e-4;
t89 = t8.*t20.*3.074667945623095e-1;
t90 = t9.*t11.*6.784571152745185e-4;
t91 = t4.*t22.*8.440206545624689e-2;
t92 = t3.*t8.*t9.*2.265025256144936e-4;
t93 = t8.*t20.*t32.*7.970632707682899e-2;
t94 = t5.^2;
t95 = t3.*t11.*3.689996292735745e-2;
t96 = t5.*t11.*4.915167130564437e-3;
t97 = t11.*4.310799465649219e-3;
t98 = t8.*3.807418306592183e-2;
t99 = t5.*t11.*3.791607093361699;
t100 = t11.*t30.*t31.*1.547905453732908;
t101 = t11.*2.219760847427988e-4;
t102 = t8.*1.960554684600962e-3;
t103 = t6.*t8.*2.265025256144936e-4;
t104 = t8.*t9.*6.784571152745185e-4;
t105 = t4.*t13.*8.440206545624689e-2;
t106 = t5.*t11.*3.436486650567527e-1;
t107 = t11.*t30.*t31.*7.970632707682899e-2;
t108 = t3.*t6.*t11.*6.784571152745185e-4;
t109 = t5.*t7.*t11.*8.440206545624689e-2;
t110 = t4.*t5.*t11.*1.199966622536514e-4;
t111 = t6.*t11.*3.439231171461361e-3;
t112 = t3.*t8.*t9.*3.439231171461361e-3;
t113 = t11.*3.807418306592183e-2;
t114 = t8.*t20.*5.971038255043736;
t116 = t8.*t20.*t32.*1.547905453732908;
t117 = t11.*6.271590127205854e-2;
t118 = t8.*t20.*7.153708691033507;
t119 = t4.*t13.*2.061478095729509e-3;
t120 = t5.*t7.*t11.*2.061478095729509e-3;
t121 = t11.*6.104217881481557e-4;
t122 = t8.*5.391415465873457e-3;
t123 = t6.*t8.*3.104999007011269e-3;
t124 = t8.*t9.*1.865719029901695e-3;
t125 = t5.*t11.*9.450145625450081e-1;
t126 = t11.*t30.*t31.*2.191879307959464e-1;
t127 = t3.*t6.*t11.*1.865719029901695e-3;
t462 = t11.*t20.*8.455164471901305e-1;
t463 = t3.*t9.*t11.*3.104999007011269e-3;
t464 = t11.*t20.*t32.*2.191879307959464e-1;
t128 = t41+t42+t43+t45+t46+t47-t63-t67+t121+t122+t123+t124+t125+t126+t127-t462-t463-t464;
t129 = t11.*3.038635549296489e-3;
t130 = t8.*t20.*1.247534853861598e1;
t131 = t8.*t30.*1.227529861371644e-2;
t132 = t11.*8.018329442092692e-2;
t441 = t9.*t11.*2.272477191789019e-2;
t454 = t5.*t8.*3.813159268614815;
t455 = t3.*t8.*1.618000866946239e-1;
t456 = t8.*t30.*t31.*1.85449568806793;
t457 = t8.*1.25890039900759e-2;
t133 = t33+t34+t35+t36+t37+t38+t50+t51+t52+t53-t88-t115+t130+t131+t132-t441-t454-t455-t456-t457;
t134 = t3.*t6.*t8.*1.294017156131404e-3;
t350 = t5.*t8.*1.497952838441835e-1;
t351 = t9.*t11.*1.294017156131404e-3;
t135 = t111+t112+t134-t350-t351;
t136 = t3.*3.014583803046025e-1;
t166 = t5.*t6.*5.951618727895023e-4;
t137 = t136-t166;
t138 = t5.*t9.*1.986944558488843e-4;
t139 = t3.*t4.*1.052644841177257e-4;
t140 = t5.*t6.*t7.*1.052644841177257e-4;
t141 = t138+t139+t140;
t142 = t11.*t141.*1.139953928995173;
t143 = t5.*1.259578569946919e15;
t144 = t30.*4.858818610819424e15;
t145 = t143+t144;
t146 = t14.*t71.*3.37770948362828e-2;
t147 = t3.*t7.*7.403989170917124e-2;
t148 = t5.*t9.*t17.*3.37770948362828e-2;
t149 = t5.*t9.*t14.*1.095176343335877e-3;
t174 = t17.*t71.*1.095176343335877e-3;
t175 = t4.*t5.*t6.*7.403989170917124e-2;
t150 = t146+t147+t148+t149-t174-t175;
t151 = t11.*t150.*1.139953928995173;
t152 = t17.*t25.*1.095176343335877e-3;
t153 = t17.*t29.*3.37770948362828e-2;
t154 = t4.*t22.*7.403989170917124e-2;
t155 = t14.*t29.*1.095176343335877e-3;
t331 = t14.*t25.*3.37770948362828e-2;
t332 = t5.*t7.*t8.*7.403989170917124e-2;
t156 = t152+t153+t154+t155-t331-t332;
t157 = t3.*t7.*6.715374732587727e-4;
t201 = t4.*t5.*t6.*6.715374732587727e-4;
t158 = t157-t201;
t159 = t14.*t71.*3.565423831595737e-4;
t160 = t5.*t9.*t17.*3.565423831595737e-4;
t161 = t159+t160;
t162 = t17.*t71.*6.715374732587727e-4;
t202 = t5.*t9.*t14.*6.715374732587727e-4;
t163 = t162-t202;
t164 = t8.*3.99066170156947e-3;
t165 = t129+t164;
t167 = t11.*t137.*3.134809394219319;
t168 = t11.*t145.*1.228907422423152e-15;
t169 = t3.*1.497952838441835e-1;
t170 = t5.*t9.*3.439231171461361e-3;
t171 = t5.*t6.*1.294017156131404e-3;
t172 = t169+t170+t171;
t173 = t11.*t172.*1.900321864457165e1;
t176 = t3.*t7.*2.061478095729509e-3;
t177 = t3.*t4.*1.268225234578345e-3;
t178 = t5.*t6.*t7.*1.268225234578345e-3;
t195 = t5.*t9.*1.442959919441252e-3;
t196 = t4.*t5.*t6.*2.061478095729509e-3;
t179 = t176+t177+t178-t195-t196;
t180 = t16.*t17.*3.37770948362828e-2;
t181 = t4.*t13.*7.403989170917124e-2;
t182 = t14.*t16.*1.095176343335877e-3;
t183 = t17.*t19.*1.095176343335877e-3;
t184 = t5.*t7.*t11.*7.403989170917124e-2;
t325 = t14.*t19.*3.37770948362828e-2;
t185 = t180+t181+t182+t183+t184-t325;
t186 = t11.*4.581283258289218e-4;
t187 = t8.*t20.*1.395740012982637e-1;
t188 = t8.*t30.*3.219519910626345e-4;
t189 = t186+t187+t188;
t190 = t11.*t30.*1.182670435989771;
t191 = t3.*4.915167130564437e-3;
t192 = t5.*3.302069355661744e-2;
t193 = t191+t192;
t194 = t11.*t193.*4.38483060303202;
t197 = t20.*3.219519910626345e-4;
t198 = t30.*1.395740012982637e-1;
t199 = t197-t198;
t207 = t11.*t179.*1.994855465224146;
t258 = t11.*t199.*3.812773007925995e1;
t200 = t142+t151+t167+t168+t173+t190+t194-t207-t258;
t203 = t11.*4.185385434780744e-3;
t204 = t8.*t141.*1.139953928995173;
t205 = t8.*t150.*1.139953928995173;
t206 = t82-t203;
t208 = t5.*t8.*1.51663096460419e-1;
t209 = t3.*t6.*t8.*1.889179028920907e-3;
t345 = t9.*t11.*1.889179028920907e-3;
t210 = t111+t112+t208+t209-t345;
t211 = t11.*t137.*1.139953928995173;
t212 = t11.*t145.*6.32801549491176e-17;
t213 = t142+t151+t211+t212;
t214 = t6.*t11.*1.244265463592368e-3;
t215 = t7.*t22.*1.37348971869607e-3;
t216 = t3.*t8.*t9.*1.244265463592368e-3;
t217 = t4.*t5.*t8.*1.37348971869607e-3;
t253 = t4.*t22.*2.061478095729509e-3;
t218 = t85+t214+t215+t216+t217-t253;
t219 = t8.*t9.*1.294017156131404e-3;
t220 = t3.*t6.*t11.*1.294017156131404e-3;
t234 = t6.*t8.*3.439231171461361e-3;
t313 = t5.*t11.*1.497952838441835e-1;
t221 = t81+t219+t220-t234-t313;
t222 = t8.*t137.*3.134809394219319;
t223 = t8.*t145.*1.228907422423152e-15;
t224 = t8.*t172.*1.900321864457165e1;
t225 = t11.*3.540643940569388e-4;
t226 = t8.*t20.*1.301446134121834e-1;
t227 = t8.*t137.*1.139953928995173;
t228 = t8.*t145.*6.32801549491176e-17;
t229 = t204+t205+t227+t228;
t230 = t3.*t9.*t11.*1.244265463592368e-3;
t231 = t4.*t5.*t11.*1.37348971869607e-3;
t337 = t6.*t8.*1.244265463592368e-3;
t338 = t7.*t13.*1.37348971869607e-3;
t232 = t119+t120+t230+t231-t337-t338;
t330 = t11.*3.899910832955465e-3;
t233 = t48+t49-t330;
t235 = t8.*t9.*1.889179028920907e-3;
t236 = t5.*t11.*1.51663096460419e-1;
t237 = t3.*t6.*t11.*1.889179028920907e-3;
t238 = t8.*t30.*t31.*6.992065648397489e-2;
t341 = t11.*4.807572428874383e-3;
t342 = t8.*t20.*t32.*6.992065648397489e-2;
t239 = t48+t49+t238-t341-t342;
t240 = t142+t151+t167+t168+t173+t190+t194-t207;
t241 = t11.*t20.*1.395740012982637e-1;
t333 = t8.*4.581283258289218e-4;
t242 = t54+t241-t333;
t243 = t8.*t30.*1.182670435989771;
t244 = t8.*t193.*4.38483060303202;
t247 = t8.*t179.*1.994855465224146;
t248 = t8.*t199.*3.812773007925995e1;
t245 = t204+t205+t222+t223+t224+t243+t244-t247-t248;
t246 = t11.*3.99066170156947e-3;
t249 = t11.*t145.*1.740168783636763e-16;
t250 = t142+t151+t167-t207+t249;
t251 = t6.*t11.*1.442959919441252e-3;
t252 = t7.*t22.*1.268225234578345e-3;
t254 = t3.*t8.*t9.*1.442959919441252e-3;
t255 = t4.*t5.*t8.*1.268225234578345e-3;
t256 = t8.*4.185385434780744e-3;
t257 = t129+t256;
t259 = t8.*3.540643940569388e-4;
t346 = t11.*t20.*1.301446134121834e-1;
t260 = t54+t259-t346;
t261 = t3.*t7.*2.923071757101621e-3;
t275 = t4.*t5.*t6.*2.923071757101621e-3;
t262 = t261-t275;
t263 = t4.*t13;
t264 = t5.*t7.*t11;
t265 = t263+t264;
t266 = t3.*t4.*2.923071757101621e-3;
t267 = t5.*t6.*t7.*2.923071757101621e-3;
t268 = t266+t267;
t269 = t8.*3.899910832955465e-3;
t270 = t95+t96+t269;
t271 = t8.*t145.*1.740168783636763e-16;
t272 = t3.*t9.*t11.*1.442959919441252e-3;
t273 = t4.*t5.*t11.*1.268225234578345e-3;
t328 = t6.*t8.*1.442959919441252e-3;
t329 = t7.*t13.*1.268225234578345e-3;
t274 = t119+t120+t272+t273-t328-t329;
t276 = t4.*t22;
t315 = t5.*t7.*t8;
t277 = t276-t315;
t278 = t8.*4.807572428874383e-3;
t279 = t11.*t30.*t31.*6.992065648397489e-2;
t356 = t11.*t20.*t32.*6.992065648397489e-2;
t280 = t95+t96+t278+t279-t356;
t281 = t204+t205+t222+t223+t224+t243+t244-t247;
t282 = t81-t234+t235+t236+t237;
t283 = t3.*1.112185118070801e19;
t284 = t5.*2.57961691125129e18;
t285 = t5.*t9.*7.330531551818703e15;
t286 = t3.*t4.*3.8835739971415e15;
t287 = t5.*t6.*t7.*3.8835739971415e15;
t290 = t5.*t6.*2.195759749955526e16;
t288 = t283+t284+t285+t286+t287-t290;
t289 = t8.*t137.*1.994855465224146;
t291 = t8.*t288.*3.089851315874883e-20;
t292 = t5.*t6.*t22.*1.557550994534973e-1;
t293 = t3.*t5.*t8.*2.36837910197578e-2;
t411 = t5.*t9.*t29.*1.557550994534973e-1;
t294 = t292+t293-t411;
t295 = t11.*t294;
t296 = t5.*t9.*t16.*1.557550994534973e-1;
t297 = t3.*t5.*t11.*2.36837910197578e-2;
t408 = t5.*t6.*t13.*1.557550994534973e-1;
t298 = t296+t297-t408;
t299 = t11.*t137.*1.994855465224146;
t300 = t11.*t288.*3.089851315874883e-20;
t301 = t5.*t11.*1.468199126656079;
t302 = t151+t173+t194-t207+t299+t300+t301;
t303 = t14.*t19;
t410 = t16.*t17;
t304 = t303-t410;
t305 = t161.*t304;
t306 = t14.*t16;
t307 = t17.*t19;
t308 = t306+t307;
t309 = t163.*t308;
t409 = t158.*t265;
t310 = t305+t309-t409;
t311 = t8.*t310;
t312 = t85+t251+t252-t253+t254+t255;
t314 = t5.*t8.*1.468199126656079;
t316 = t14.*t25;
t405 = t17.*t29;
t317 = t316-t405;
t318 = t161.*t317;
t319 = t17.*t25;
t320 = t14.*t29;
t321 = t319+t320;
t322 = t163.*t321;
t404 = t158.*t277;
t323 = t318+t322-t404;
t324 = t11.*t323;
t326 = t5.*t8.*1.394816037191174e-1;
t327 = t205-t247+t289+t291+t326;
t334 = t205+t224+t244-t247+t289+t291+t314;
t335 = -t188+t225+t226;
t336 = t205+t291;
t339 = t151+t300;
t340 = t205+t224-t247+t289+t291+t314;
t343 = t5.*t11.*1.394816037191174e-1;
t344 = t151-t207+t299+t300+t343;
t347 = t262.*t265;
t348 = t5.*t9.*t16.*6.280147091832467e-4;
t406 = t19.*t268;
t349 = t347+t348-t406;
t352 = t151+t173-t207+t299+t300+t301;
t353 = t262.*t277;
t354 = t5.*t9.*t29.*6.280147091832467e-4;
t407 = t25.*t268;
t355 = t353+t354-t407;
t357 = t6.*t11.*1.865719029901695e-3;
t358 = t3.*t185.*1.139953928995173;
t359 = t5.*t11.*t179.*1.994855465224146;
t360 = t3.*t6.*t8.*2.265025256144936e-4;
t361 = t3.*t8.*t9.*1.865719029901695e-3;
t362 = t8.*t9.*2.265025256144936e-4;
t363 = t3.*t312.*1.994855465224146;
t364 = t3.*t156.*1.139953928995173;
t365 = t3.*t135.*1.900321864457165e1;
t366 = t5.*t8.*t172.*1.900321864457165e1;
t367 = t5.*t8.*t150.*1.139953928995173;
t368 = t3.*t6.*t11.*2.265025256144936e-4;
t369 = t3.*t9.*t11.*1.865719029901695e-3;
t370 = t6.*t7.*t8.*1.199966622536514e-4;
t380 = t6.*t8.*1.865719029901695e-3;
t381 = t5.*t8.*t179.*1.994855465224146;
t382 = t3.*t7.*t9.*t11.*1.199966622536514e-4;
t371 = t362+t363+t364+t365+t366+t367+t368+t369+t370-t380-t381-t382;
t372 = t9.*t11.*2.265025256144936e-4;
t373 = t3.*t274.*1.994855465224146;
t374 = t3.*t221.*1.900321864457165e1;
t375 = t5.*t11.*t172.*1.900321864457165e1;
t376 = t5.*t11.*t150.*1.139953928995173;
t377 = t6.*t7.*t11.*1.199966622536514e-4;
t378 = t3.*t7.*t8.*t9.*1.199966622536514e-4;
t379 = -t357-t358-t359-t360-t361+t372+t373+t374+t375+t376+t377+t378;
t383 = t3.^2;
t384 = t6.^2;
t385 = t94.*t384.*1.557550994534973e-1;
t386 = t9.^2;
t387 = t362+t363+t364+t367+t368+t369+t370-t380-t381-t382;
t388 = t14.*t71;
t389 = t5.*t9.*t17;
t390 = t388+t389;
t391 = t161.*t390;
t393 = t73.*t158;
t394 = t17.*t71;
t430 = t5.*t9.*t14;
t395 = t394-t430;
t396 = t163.*t395;
t397 = t71.*t268;
t398 = t73.*t262;
t399 = t6.*t11.*6.784571152745185e-4;
t400 = t3.*t8.*t9.*6.784571152745185e-4;
t401 = t358+t360-t372-t376-t377-t378+t399+t400;
t402 = t3.*t9.*t11.*6.784571152745185e-4;
t686 = t6.*t8.*6.784571152745185e-4;
t403 = t362+t364+t367+t368+t370-t382+t402-t686;
t412 = t16.*t150.*1.139953928995173;
t413 = t5.*t9.*t274.*1.994855465224146;
t414 = t5.*t7.*t8.*1.199966622536514e-4;
t415 = t3.*t4.*t6.*t8.*1.199966622536514e-4;
t422 = t16.*t179.*1.994855465224146;
t423 = t4.*t9.*t11.*1.199966622536514e-4;
t424 = t5.*t9.*t185.*1.139953928995173;
t416 = t412+t413+t414+t415-t422-t423-t424;
t417 = t29.*t150.*1.139953928995173;
t418 = t4.*t8.*t9.*1.199966622536514e-4;
t419 = t5.*t7.*t11.*1.199966622536514e-4;
t420 = t3.*t4.*t6.*t11.*1.199966622536514e-4;
t425 = t29.*t179.*1.994855465224146;
t426 = t5.*t9.*t312.*1.994855465224146;
t427 = t5.*t9.*t156.*1.139953928995173;
t421 = t417+t418+t419+t420-t425-t426-t427;
t428 = t412+t414+t415-t423-t424;
t429 = t417+t418+t419+t420-t427;
t431 = t391+t393+t396;
t432 = t94.*t386.*6.280147091832467e-4;
t433 = t397+t398+t432;
t434 = t73.*t185.*1.139953928995173;
t435 = t73.*t156.*1.139953928995173;
t438 = t150.*t277.*1.139953928995173;
t436 = t435-t438;
t439 = t150.*t265.*1.139953928995173;
t437 = t434-t439;
t440 = t82-t246;
t447 = t8.*2.219760847427988e-4;
t448 = t5.*t8.*3.436486650567527e-1;
t449 = t7.*t22.*1.199966622536514e-4;
t450 = t8.*t30.*t31.*7.970632707682899e-2;
t451 = t3.*t6.*t8.*6.784571152745185e-4;
t452 = t5.*t7.*t8.*8.440206545624689e-2;
t453 = t4.*t5.*t8.*1.199966622536514e-4;
t442 = t33+t35+t37+t86+t87-t88+t89+t90+t91+t92+t93-t447-t448-t449-t450-t451-t452-t453;
t716 = t8.*5.164630050170653e-3;
t458 = t33+t34+t35+t36+t37+t38+t50+t51+t52+t53-t88-t115+t117+t118-t441-t454-t455-t456-t716;
t710 = t8.*4.310799465649219e-3;
t711 = t5.*t8.*3.791607093361699;
t712 = t8.*t30.*t31.*1.547905453732908;
t459 = t33+t34+t35+t36+t37+t38+t50+t51+t52-t88+t113+t114-t115+t116-t441-t710-t711-t712;
t460 = t5.*t6.*1.889179028920907e-3;
t482 = t3.*1.51663096460419e-1;
t461 = t170+t460-t482;
t465 = t3.*t4.*1.37348971869607e-3;
t466 = t5.*t6.*t7.*1.37348971869607e-3;
t529 = t5.*t9.*1.244265463592368e-3;
t467 = t176-t196+t465+t466-t529;
t478 = t11.*t20.*3.074667945623095e-1;
t479 = t7.*t13.*1.199966622536514e-4;
t480 = t3.*t9.*t11.*2.265025256144936e-4;
t481 = t11.*t20.*t32.*7.970632707682899e-2;
t468 = t41+t42+t43-t63+t101+t102+t103+t104+t105+t106+t107+t108+t109+t110-t478-t479-t480-t481;
t472 = t11.*t20.*7.153708691033507;
t469 = t41+t42+t43+t44+t45+t46+t47+t55+t56+t57+t61+t62-t63-t64-t65-t66-t67-t68-t472;
t470 = t30.*1.301446134121834e-1;
t471 = t197+t470;
t473 = t5.*3.689996292735745e-2;
t474 = t191-t473;
t476 = t11.*t20.*5.971038255043736;
t477 = t11.*t20.*t32.*1.547905453732908;
t475 = t41+t42+t43+t44+t45+t46+t47-t63-t64-t65-t66-t67+t97+t98+t99+t100-t476-t477;
t483 = t204+t205+t222-t247+t271;
t484 = t20.*t32.*2.191879307959464e-1;
t485 = t11.*t274.*1.994855465224146;
t486 = t8.*t312.*1.994855465224146;
t487 = t8.*t156.*1.139953928995173;
t488 = t6.*t30.*t31.*1.865719029901695e-3;
t489 = t9.*t20.*t32.*2.265025256144936e-4;
t490 = t6.*t7.*t20.*t32.*1.199966622536514e-4;
t491 = t20.^2;
t492 = t30.^2;
t493 = t14.*t16.*6.715374732587727e-4;
t494 = t17.*t19.*6.715374732587727e-4;
t495 = t493+t494;
t496 = t4.*t13.*6.715374732587727e-4;
t497 = t5.*t7.*t11.*6.715374732587727e-4;
t498 = t496+t497;
t499 = t14.*t19.*3.565423831595737e-4;
t514 = t16.*t17.*3.565423831595737e-4;
t500 = t499-t514;
t501 = t11.*t185.*1.139953928995173;
t502 = t4.*t20.*t31.*1.199966622536514e-4;
t503 = t4.*t30.*t32.*1.199966622536514e-4;
t504 = t9.*t30.*t31.*2.265025256144936e-4;
t505 = t6.*t7.*t30.*t31.*1.199966622536514e-4;
t506 = t3.*1.328717522936961;
t507 = t20.*t31.*9.450145625450081e-1;
t508 = t30.*t32.*9.450145625450081e-1;
t509 = t8.*t135.*1.900321864457165e1;
t510 = t30.*t31.*2.191879307959464e-1;
t511 = t11.*t221.*1.900321864457165e1;
t512 = t6.*t20.*t32.*1.865719029901695e-3;
t513 = t20.*7.153708691033507;
t515 = t4.*t13.*2.923071757101621e-3;
t516 = t5.*t7.*t11.*2.923071757101621e-3;
t517 = t515+t516;
t518 = t7.*t13.*2.923071757101621e-3;
t528 = t4.*t5.*t11.*2.923071757101621e-3;
t519 = t518-t528;
t520 = t6.*t8.*6.280147091832467e-4;
t527 = t3.*t9.*t11.*6.280147091832467e-4;
t521 = t520-t527;
t522 = t8.*t9.*1.557550994534973e-1;
t523 = t3.*t6.*t11.*1.557550994534973e-1;
t524 = t522+t523;
t525 = t6.*t8.*1.557550994534973e-1;
t536 = t3.*t9.*t11.*1.557550994534973e-1;
t526 = t525-t536;
t530 = t204+t205+t222+t223+t224-t247;
t531 = t11.^2;
t543 = t20.*8.455164471901305e-1;
t532 = -t484-t485-t486-t487-t488-t489-t490+t501+t502+t503+t504+t505+t507+t508+t510+t512-t543;
t533 = t20.*5.971038255043736;
t534 = t484+t485+t486+t487+t488+t489+t490-t501-t502-t503-t504-t505+t506-t507-t508+t509-t510+t511-t512+t533;
t535 = t8.^2;
t537 = t20.*t31.*3.436486650567527e-1;
t538 = t30.*t32.*3.436486650567527e-1;
t539 = t30.*t31.*7.970632707682899e-2;
t540 = t6.*t20.*t32.*6.784571152745185e-4;
t544 = t20.*3.074667945623095e-1;
t545 = t20.*t32.*7.970632707682899e-2;
t546 = t6.*t30.*t31.*6.784571152745185e-4;
t541 = -t487-t489-t490+t501+t502+t503+t504+t505+t537+t538+t539+t540-t544-t545-t546;
t548 = t11.*t280.*4.38483060303202;
t549 = t8.*t239.*4.38483060303202;
t542 = t484+t485+t486+t487+t488+t489+t490-t501-t502-t503-t504-t505+t506-t507-t508+t509-t510+t511-t512+t513-t548-t549;
t547 = t142+t151+t167+t168+t173-t207;
t550 = t8.*t11.*t491.*1.065602502591819e-1;
t551 = t8.*t11.*t492.*2.844235507266242e-1;
t552 = t550+t551-t8.*t11.*2.844235507266242e-1;
t553 = t11.*t242.*3.812773007925995e1;
t554 = t8.*t189.*3.812773007925995e1;
t555 = t8.*t11.*t383.*5.436562614985332e-3;
t556 = t8.*t11.*t94.*4.50469717884937e-3;
t591 = t8.*t11.*4.50469717884937e-3;
t557 = t555+t556-t591;
t558 = t6.*t11.*1.557550994534973e-1;
t559 = t3.*t8.*t9.*1.557550994534973e-1;
t560 = t558+t559;
t561 = t9.*t11.*1.557550994534973e-1;
t581 = t3.*t6.*t8.*1.557550994534973e-1;
t562 = t561-t581;
t563 = t17.*t25.*6.715374732587727e-4;
t564 = t14.*t29.*6.715374732587727e-4;
t565 = t563+t564;
t566 = t4.*t22.*6.715374732587727e-4;
t579 = t5.*t7.*t8.*6.715374732587727e-4;
t567 = t566-t579;
t568 = t14.*t25.*3.565423831595737e-4;
t578 = t17.*t29.*3.565423831595737e-4;
t569 = t568-t578;
t570 = t6.*t11.*6.280147091832467e-4;
t571 = t3.*t8.*t9.*6.280147091832467e-4;
t572 = t570+t571;
t573 = t4.*t22.*2.923071757101621e-3;
t580 = t5.*t7.*t8.*2.923071757101621e-3;
t574 = t573-t580;
t575 = t7.*t22.*2.923071757101621e-3;
t576 = t4.*t5.*t8.*2.923071757101621e-3;
t577 = t575+t576;
t582 = t3.*1.547905453732908;
t583 = t3.*t9.*2.265025256144936e-4;
t584 = t3.*t6.*t7.*1.199966622536514e-4;
t585 = t308.*t495;
t586 = t265.*t498;
t587 = t304.*t500;
t588 = t585+t586+t587;
t589 = t8.*t588;
t602 = t4.*t5.*1.199966622536514e-4;
t613 = t5.*9.450145625450081e-1;
t614 = t3.*t6.*1.865719029901695e-3;
t590 = t485+t486+t487-t501+t509+t511-t548-t549+t582+t583+t584-t602-t613-t614;
t592 = t321.*t495;
t593 = t277.*t498;
t594 = t317.*t500;
t595 = t592+t593+t594;
t596 = t11.*t595;
t597 = t265.*t517;
t598 = t19.*t519;
t599 = t16.*t521;
t600 = t597+t598+t599;
t601 = t8.*t600;
t603 = t94.*t531.*2.36837910197578e-2;
t604 = t13.*t524;
t605 = t16.*t526;
t606 = t603+t604+t605;
t607 = t8.*t606;
t608 = t29.*t521;
t609 = t25.*t519;
t610 = t277.*t517;
t611 = t608+t609+t610;
t612 = t11.*t611;
t615 = t3.*7.970632707682899e-2;
t616 = t5.*3.436486650567527e-1;
t629 = t3.*t6.*6.784571152745185e-4;
t617 = t487-t501+t583+t584-t602+t615-t616-t629;
t618 = t535.*4.50469717884937e-3;
t619 = t383.*t531.*5.436562614985332e-3;
t620 = t94.*t531.*4.50469717884937e-3;
t621 = t618+t619+t620;
t622 = t8.*t621;
t623 = t29.*t526;
t624 = t22.*t524;
t663 = t8.*t11.*t94.*2.36837910197578e-2;
t625 = t623+t624-t663;
t626 = t11.*t625;
t627 = t3.*2.191879307959464e-1;
t628 = t485+t486+t487-t501+t509+t511+t582+t583+t584-t602-t613-t614;
t630 = t485+t486+t487-t501+t583+t584-t602-t613-t614+t627;
t631 = t94.*t535.*2.36837910197578e-2;
t632 = t29.*t560;
t633 = t22.*t562;
t634 = t631+t632+t633;
t635 = t11.*t634;
t636 = t308.*t565;
t637 = t265.*t567;
t638 = t304.*t569;
t639 = t636+t637+t638;
t640 = t8.*t639;
t641 = t16.*t572;
t642 = t265.*t574;
t643 = t19.*t577;
t644 = t641+t642+t643;
t645 = t8.*t644;
t646 = t317.*t569;
t647 = t321.*t565;
t648 = t277.*t567;
t649 = t646+t647+t648;
t650 = t11.*t649;
t651 = t29.*t572;
t652 = t25.*t577;
t653 = t277.*t574;
t654 = t651+t652+t653;
t655 = t11.*t654;
t656 = t531.*4.50469717884937e-3;
t657 = t383.*t535.*5.436562614985332e-3;
t658 = t94.*t535.*4.50469717884937e-3;
t659 = t656+t657+t658;
t660 = t11.*t659;
t661 = t13.*t562;
t662 = t16.*t560;
t664 = t357+t358+t359+t360+t361-t372-t373-t376-t377-t378;
t665 = t73.*t517;
t666 = t5.*t9.*t521;
t667 = t6.*7.330531551818703e15;
t668 = t9.*2.195759749955526e16;
t674 = t7.*t9.*3.8835739971415e15;
t669 = t667+t668-t674;
t670 = t5.*t669.*3.089851315874883e-20;
t671 = t5.*t8.*t185.*1.139953928995173;
t672 = t5.*t11.*t156.*1.139953928995173;
t673 = t5.*t9.*1.187261914627176e-3;
t675 = t5.*t11.*t312.*1.994855465224146;
t676 = t5.*t11.*t135.*1.900321864457165e1;
t678 = t5.*t8.*t274.*1.994855465224146;
t679 = t5.*t8.*t221.*1.900321864457165e1;
t677 = t670+t671+t672+t673+t675+t676-t678-t679;
t680 = t5.*t9.*t526;
t681 = t670+t671+t672+t673+t675-t678;
t682 = t670+t671+t672;
t683 = t73.*t498;
t684 = t390.*t569;
t685 = t395.*t565;
t687 = t71.*t577;
t688 = t5.*t6.*t562;
t689 = t661+t662-t663;
t690 = t16.*t156.*1.139953928995173;
t691 = t29.*t274.*1.994855465224146;
t692 = t3.*t7.*1.199966622536514e-4;
t693 = t16.*t312.*1.994855465224146;
t695 = t29.*t185.*1.139953928995173;
t696 = t4.*t5.*t6.*1.199966622536514e-4;
t694 = t690+t691+t692+t693-t695-t696;
t697 = t690+t692-t695-t696;
t709 = t73.*t567;
t698 = t684+t685-t709;
t699 = t73.*t574;
t700 = t5.*t9.*t572;
t701 = -t687+t699+t700;
t722 = t71.*t519;
t702 = t665+t666-t722;
t703 = t390.*t500;
t704 = t395.*t495;
t705 = -t683+t703+t704;
t706 = t156.*t265.*1.139953928995173;
t708 = t185.*t277.*1.139953928995173;
t707 = t706-t708;
t713 = t172.*t459;
t714 = t150.*t442;
t715 = t442.*t467;
t717 = t193.*t458;
t718 = t3.*t5.*t8.*2.275192558362184e-2;
t719 = t128.*t461;
t720 = t474.*t475;
t721 = t128.*t179;
t723 = t3.*t5.*t11.*2.275192558362184e-2;
t724 = t218.*t541;
t725 = t135.*t534;
t726 = t229.*t467;
t727 = t172.*t530;
t728 = t210.*t532;
t729 = t233.*t534;
t730 = t193.*t281;
t731 = t150.*t229;
t732 = t232.*t541;
t733 = t213.*t467;
t734 = t221.*t534;
t735 = t193.*t240;
t736 = t172.*t547;
t737 = t150.*t213;
t738 = t282.*t532;
t739 = t270.*t534;
t740 = t185.*t541;
t741 = t8.*t689;
t742 = t150.*t339;
t743 = t270.*t628;
t744 = t172.*t352;
t745 = t274.*t630;
t746 = t193.*t302;
t747 = t339.*t467;
t748 = t221.*t628;
t749 = t150.*t336;
t750 = t156.*t617;
t751 = t172.*t340;
t752 = t135.*t628;
t753 = t336.*t467;
t754 = t193.*t334;
t755 = t461.*t664;
t756 = t3.*t702;
t757 = t233.*t677;
t758 = t179.*t664;
t759 = t172.*t379;
t823 = t5.*t6.*t524;
t760 = t297+t680-t823;
t761 = t3.*t760;
t762 = t135.*t677;
t763 = t312.*t681;
t764 = t156.*t682;
t765 = t193.*t379;
t766 = t5.*t11.*t600;
t767 = t5.*t11.*t606;
t768 = t5.*t11.*t588;
t769 = t3.*t698;
t770 = t403.*t467;
t771 = t282.*t681;
t772 = t172.*t371;
t773 = t280.*t677;
t774 = t193.*t371;
t775 = t185.*t682;
t776 = t150.*t403;
t822 = t5.*t9.*t560;
t777 = t293+t688-t822;
t778 = t3.*t777;
t779 = t232.*t682;
t780 = t5.*t8.*t634;
t781 = t5.*t8.*t649;
t782 = t5.*t8.*t654;
t783 = t29.*t649;
t784 = t29.*t654;
t785 = t270.*t694;
t786 = t150.*t429;
t787 = t221.*t694;
t788 = t172.*t421;
t789 = t16.*t639;
t790 = t429.*t467;
t791 = t16.*t644;
t792 = t274.*t694;
t793 = t193.*t421;
t794 = t5.*t9.*t701;
t795 = t312.*t694;
t796 = t233.*t694;
t797 = t150.*t428;
t798 = t172.*t416;
t799 = t135.*t694;
t800 = t16.*t588;
t801 = t193.*t416;
t802 = t156.*(t690+t692-t695-t696);
t803 = t428.*t467;
t804 = t16.*t600;
t805 = t29.*t595;
t806 = t29.*t611;
t807 = t5.*t9.*t702;
t808 = t265.*t588;
t809 = t277.*t595;
t810 = t232.*t707;
t811 = t282.*t707;
t812 = t436.*t467;
t813 = t73.*t698;
t814 = t185.*t707;
t815 = t172.*t436;
t816 = t280.*t707;
t817 = t150.*t436;
t818 = t193.*t436;
t819 = t383.*2.36837910197578e-2;
t820 = t185.*t468;
t821 = t94.*t386.*1.563831141626805e-1;
t824 = t156.*t213;
t825 = t185.*t229;
t826 = t229.*t232;
t827 = t250.*t312;
t828 = t282.*t327;
t829 = t312.*t344;
t830 = t185.*t336;
t831 = t156.*t339;
t832 = t232.*t336;
t833 = t135.*t352;
t834 = t312.*t630;
t835 = t210.*t387;
t836 = t218.*t403;
t837 = t94.*t386.*1.557550994534973e-1;
t838 = t385+t819+t837;
t839 = t5.*t8.*t355;
t840 = t5.*t11.*t310;
t841 = t282.*t416;
t842 = t185.*t428;
t843 = t135.*t421;
t844 = t16.*t310;
t845 = t29.*t323;
t846 = t156.*t429;
t847 = t232.*t428;
t848 = t312.*t421;
t849 = t277.*t323;
t850 = t218.*t436;
t851 = t210.*t436;
t852 = t274.*(t434-t439);
t853 = t265.*t310;
t854 = t179.*(t434-t439);
t855 = t135.*(t706-t708);
t856 = t312.*(t706-t708);
t857 = t461.*(t434-t439);
t858 = t156.*(t706-t708);
t859 = t232.*t468;
t860 = t156.*t442;
t861 = t80.*t312;
t862 = t185.*t401;
t863 = t312.*t387;
t864 = t3.*t431;
t865 = t3.*t433;
t866 = t232.*t401;
t867 = t156.*t403;
t868 = t5.*t8.*t323;
t869 = t5.*t11.*t349;
t870 = t232.*t437;
t871 = t156.*t436;
t872 = t73.*t431;
t873 = t185.*t437;
t874 = t312.*t436;
t875 = t150.*t468;
M = reshape([t94.*5.436562614985332e-3+t383.*2.818848819860717e-2+t385+t391+t393+t396+t397+t398+t491.*2.844235507266242e-1+t492.*1.065602502591819e-1+t820+t821-t221.*(t41+t42+t43+t44+t45+t46+t47+t97+t98+t99+t100-t8.*t9.*2.272477191789019e-2-t11.*t20.*5.971038255043736-t14.*t19.*3.850433196866315e-2-t3.*t6.*t11.*2.272477191789019e-2-t4.*t5.*t11.*2.409929378080134e-3-t3.*t9.*t11.*6.84614609275178e-2-t11.*t20.*t32.*1.547905453732908)+t135.*(t8.*(-4.310799465649219e-3)+t33+t34+t35+t36+t37+t38+t50+t51+t52-t88+t113+t114-t115+t116-t5.*t8.*3.791607093361699-t9.*t11.*2.272477191789019e-2-t8.*t30.*t31.*1.547905453732908)-t257.*(t8.*(-3.21359622633761e-1)-t11.*1.439875479087047e-1+t33+t34+t35+t36+t37+t38+t50+t51+t52+t53+t130+t131-t3.*t8.*1.618000866946239e-1-t5.*t8.*3.813159268614815-t9.*t11.*2.272477191789019e-2-t14.*t25.*3.850433196866315e-2-t5.*t7.*t8.*8.028971461054102e-2-t8.*t30.*t31.*1.85449568806793)-t80.*t210+t133.*t165-t60.*t242+t133.*t189-t128.*t274+t60.*t440-t218.*t442-t270.*t475+t280.*t469-t239.*(t8.*(-5.164630050170653e-3)+t33+t34+t35+t36+t37+t38+t50+t51+t52+t53+t117+t118-t3.*t8.*1.618000866946239e-1-t5.*t8.*3.813159268614815-t9.*t11.*2.272477191789019e-2-t14.*t25.*3.850433196866315e-2-t5.*t7.*t8.*8.028971461054102e-2-t8.*t30.*t31.*1.85449568806793)+t260.*(t41+t42+t43+t44+t45+t46+t47+t55+t56+t57+t61+t62-t8.*t9.*2.272477191789019e-2-t11.*t20.*7.153708691033507-t14.*t19.*3.850433196866315e-2-t3.*t6.*t11.*2.272477191789019e-2-t4.*t5.*t11.*2.409929378080134e-3-t3.*t9.*t11.*6.84614609275178e-2-t11.*t20.*t32.*1.85449568806793)+t233.*(t8.*(-4.310799465649219e-3)+t33+t34+t35+t36+t37+t38+t50+t51+t52+t113+t114+t116-t5.*t8.*3.791607093361699-t9.*t11.*2.272477191789019e-2-t14.*t25.*3.850433196866315e-2-t5.*t7.*t8.*8.028971461054102e-2-t8.*t30.*t31.*1.547905453732908)+t128.*(t81+t235+t236+t237-t6.*t8.*3.439231171461361e-3)-t206.*(t8.*(-1.439875479087047e-1)+t11.*3.21359622633761e-1+t41+t42+t43+t44+t45+t46+t47+t55+t56+t57-t63-t64-t65-t66-t67-t68-t83-t84)+(t225+t226-t8.*t30.*3.219519910626345e-4).*(t8.*(-5.164630050170653e-3)+t33+t34+t35+t36+t37+t38+t50+t51+t52+t53-t88-t115+t117+t118-t3.*t8.*1.618000866946239e-1-t5.*t8.*3.813159268614815-t9.*t11.*2.272477191789019e-2-t8.*t30.*t31.*1.85449568806793)+t80.*(t85+t251+t252+t254+t255-t4.*t22.*2.061478095729509e-3)+t232.*(t41+t42+t43+t101+t102+t103+t104+t105+t106+t107+t108+t109+t110-t7.*t13.*1.199966622536514e-4-t11.*t20.*3.074667945623095e-1-t14.*t19.*3.850433196866315e-2-t3.*t9.*t11.*2.265025256144936e-4-t11.*t20.*t32.*7.970632707682899e-2)+t156.*(t8.*(-2.219760847427988e-4)+t33+t35+t37+t86+t87+t89+t90+t91+t92+t93-t5.*t8.*3.436486650567527e-1-t7.*t22.*1.199966622536514e-4-t14.*t25.*3.850433196866315e-2-t3.*t6.*t8.*6.784571152745185e-4-t4.*t5.*t8.*1.199966622536514e-4-t5.*t7.*t8.*8.440206545624689e-2-t8.*t30.*t31.*7.970632707682899e-2)+3.719750583795892e-1,t11.*(t684+t685+t687+t688+t713+t714+t715+t717+t718-t80.*t179-t133.*t199-t80.*t461-t73.*t567-t73.*t574+t458.*t471-t459.*t474+t8.*t20.*t30.*1.778633004674423e-1-t5.*t9.*t560-t5.*t9.*t572)-t8.*(t665+t666+t680+t683+t719+t720+t721+t723+t60.*t199-t71.*t519-t150.*t468-t172.*t475-t193.*t469-t390.*t500-t395.*t495-t467.*t468-t469.*t471+t11.*t20.*t30.*1.778633004674423e-1-t5.*t6.*t524),-t8.*(t665+t666+t680+t683-t703-t704+t719+t720+t721-t722+t723-t150.*t468-t172.*t475-t193.*t469-t467.*t468-t5.*t6.*t524)+t11.*(t684+t685+t687+t688-t699-t700-t709+t713+t714+t715+t717+t718-t80.*t179-t80.*t461-t459.*t474-t5.*t9.*t560),-t3.*(t385+t391+t393+t396+t397+t398+t819+t820+t821+t859+t860+t861-t80.*t210-t128.*t274+t128.*t282+t135.*t459-t218.*t442-t221.*t475)-t5.*t8.*(t293+t684+t685+t687+t688-t699-t700-t709+t713+t714+t715-t822-t80.*t179-t80.*t461)-t5.*t11.*(t297+t665+t666+t680+t683-t703-t704+t719+t721-t722-t823-t150.*t468-t172.*t475-t467.*t468),t29.*(t684+t685+t687-t699-t700-t709+t714+t715-t80.*t179)+t16.*(-t665-t666-t683+t703+t704-t721+t722+t875+t467.*t468)-t5.*t9.*(t391+t393+t396+t397+t398+t432+t820+t859+t860+t861-t128.*t274-t218.*t442),t277.*(t684+t685-t709+t714)+t265.*(-t683+t703+t704+t875)-t73.*(t391+t393+t396+t820+t860),t295+t311+t324+t824+t825+t826+t827+t135.*(t142+t151+t167+t168+t173-t11.*t179.*1.994855465224146)-t221.*(t204+t205+t222+t223+t224-t8.*t179.*1.994855465224146)-t8.*t298-t8.*t349+t165.*t200-t11.*t355+t189.*t200-t213.*t218-t206.*t245-t200.*t257-t210.*t250-t239.*t240-t242.*t245+t260.*t281+t280.*t281+t240.*t335+t245.*t440-t274.*t483+t233.*t547-t270.*t530+t282.*(t204+t205+t222+t271-t8.*t179.*1.994855465224146),t8.*(t589+t596+t601+t607+t612+t622+t626+t724+t725+t726+t727+t728+t729+t730+t731+t335.*(t484+t485+t486+t487+t488+t489+t490+t506+t509+t511+t513-t20.*t31.*9.450145625450081e-1-t30.*t31.*2.191879307959464e-1-t30.*t32.*9.450145625450081e-1-t11.*t185.*1.139953928995173-t8.*t239.*4.38483060303202-t11.*t280.*4.38483060303202-t4.*t20.*t31.*1.199966622536514e-4-t6.*t20.*t32.*1.865719029901695e-3-t4.*t30.*t32.*1.199966622536514e-4-t9.*t30.*t31.*2.265025256144936e-4-t6.*t7.*t30.*t31.*1.199966622536514e-4)+t189.*(t484+t485+t486+t487+t488+t489+t490-t501-t502-t503-t504-t505+t506-t507-t508+t509-t510+t511-t512+t513+t553+t554-t8.*t239.*4.38483060303202-t11.*t280.*4.38483060303202)-t199.*t245-t11.*t552-t11.*t557-t179.*t483-t156.*t541+t281.*t471-t239.*t542-t312.*t532-t461.*t483-t474.*t530+t8.*(t535.*2.844235507266242e-1+t491.*t531.*1.065602502591819e-1+t492.*t531.*2.844235507266242e-1))+t11.*(t635+t640+t645+t650+t655+t660+t732+t733+t734+t735+t736+t737+t738+t739+t740+t8.*(t661+t662-t8.*t11.*t94.*2.36837910197578e-2)+t242.*(t484+t485+t486+t487+t488+t489+t490-t501-t502-t503-t504-t505+t506-t507-t508+t509-t510+t511-t512+t513-t548-t549+t553+t554)-t199.*t200-t179.*t250-t8.*t552-t8.*t557+t240.*t471-t250.*t461-t260.*t542-t274.*t532-t280.*t542-t474.*t547+t11.*(t531.*2.844235507266242e-1+t491.*t535.*1.065602502591819e-1+t492.*t535.*2.844235507266242e-1)),t11.*(t635+t640+t645+t650+t655+t660+t732+t733+t734+t735+t736+t737+t738+t739+t740+t741-t179.*t250-t8.*t557-t250.*t461-t274.*t532-t280.*t542-t474.*t547)+t8.*(t589+t596+t601+t607+t612+t622+t626+t724+t725+t726+t727+t728+t729+t730+t731-t11.*t557-t179.*t483-t156.*t541-t239.*t542-t312.*t532-t461.*t483-t474.*t530),-t3.*(t295+t311+t324+t824+t825+t826+t827-t8.*t298-t8.*t349-t11.*t355-t213.*t218-t210.*t250+t135.*t547-t221.*t530-t274.*t483+t282.*t483)+t5.*t11.*(t589+t596+t601+t607+t612+t626+t724+t725+t726+t727+t728+t731-t179.*t483-t156.*t541-t312.*t532-t461.*t483)-t5.*t8.*(t635+t640+t645+t650+t655+t732+t733+t734+t736+t737+t738+t740+t741-t179.*t250-t250.*t461-t274.*t532),t16.*(t589+t596+t601+t612+t724+t726+t731-t179.*t483-t156.*t541-t312.*t532)+t29.*(t640+t645+t650+t655+t732+t733+t737+t740-t179.*t250-t274.*t532)-t5.*t9.*(t311+t324+t824+t825+t826+t827-t8.*t349-t11.*t355-t213.*t218-t274.*t483),-t73.*(t311+t324+t824+t825)+t277.*(t640+t650+t737+t740)+t265.*(t589+t596+t731-t156.*t541),t295+t311+t324+t828+t829+t830+t831+t832+t833-t8.*t298-t8.*t349-t11.*t355+t165.*t302+t189.*t302-t206.*t334-t239.*t302-t210.*t344-t218.*t339-t257.*t302-t221.*t340-t242.*t334+t233.*t352+t260.*t334-t274.*t327-t270.*t340+t280.*t334+t302.*t335+t334.*t440,t8.*(t589+t596+t601+t607+t612+t622+t626+t749+t750+t751+t752+t753+t754-t179.*t327-t199.*t334-t11.*t557+t189.*t590-t327.*t461+t334.*t471-t340.*t474-t239.*t590-t218.*t617-t210.*t630+t335.*t590+t233.*(t5.*(-9.450145625450081e-1)+t485+t486+t487-t501+t509+t511+t582+t583+t584-t3.*t6.*1.865719029901695e-3-t4.*t5.*1.199966622536514e-4)+t312.*(t5.*(-9.450145625450081e-1)+t485+t486+t487-t501+t583+t584+t627-t3.*t6.*1.865719029901695e-3-t4.*t5.*1.199966622536514e-4))+t11.*(t635+t640+t645+t650+t655+t660+t741+t742+t743+t744+t745+t746+t747+t748-t199.*t302-t179.*t344-t8.*t557+t302.*t471-t185.*t617-t344.*t461-t352.*t474+t242.*t590-t232.*t617-t260.*t590-t280.*t590-t282.*t630),t8.*(t589+t596+t601+t607+t612+t622+t626+t749+t750+t751+t752+t753+t754+t834-t179.*t327-t11.*t557-t327.*t461-t340.*t474-t239.*t590-t218.*t617-t210.*t630+t233.*t628)+t11.*(t635+t640+t645+t650+t655+t660+t741+t742+t743+t744+t745+t746+t747+t748-t179.*t344-t8.*t557-t185.*t617-t344.*t461-t352.*t474-t232.*t617-t280.*t590-t282.*t630),-t3.*(t295+t311+t324+t828+t829+t830+t831+t832+t833-t8.*t298-t8.*t349-t11.*t355-t210.*t344-t218.*t339-t221.*t340-t274.*t327)-t5.*t8.*(t635+t640+t645+t650+t655+t741+t742+t744+t745+t747+t748-t179.*t344-t185.*t617-t344.*t461-t232.*t617-t282.*t630)+t5.*t11.*(t589+t596+t601+t607+t612+t626+t749+t750+t751+t752+t753+t834-t179.*t327-t327.*t461-t218.*t617-t210.*t630),t29.*(t640+t645+t650+t655+t742+t745+t747-t179.*t344-t185.*t617-t232.*t617)+t16.*(t589+t596+t601+t612+t749+t750+t753+t834-t179.*t327-t218.*t617)-t5.*t9.*(t311+t324+t829+t830+t831+t832-t8.*t349-t11.*t355-t218.*t339-t274.*t327),-t73.*(t311+t324+t830+t831)+t265.*(t589+t596+t749+t750)+t277.*(t640+t650+t742-t185.*t617),t835+t836+t839+t840-t3.*t431-t3.*t433-t135.*t371-t165.*t371-t156.*t403-t189.*t371-t206.*t379-t185.*t401-t221.*t379-t233.*t371+t239.*t371-t242.*t379+t257.*t371-t232.*t401+t260.*t379-t270.*t379+t280.*t379-t312.*t387-t335.*t371+t379.*t440-t3.*t838-t282.*t664+t274.*(t357+t358+t359+t360+t361-t9.*t11.*2.265025256144936e-4-t3.*t274.*1.994855465224146-t6.*t7.*t11.*1.199966622536514e-4-t5.*t11.*t150.*1.139953928995173-t3.*t7.*t8.*t9.*1.199966622536514e-4)-t5.*t8.*t294-t5.*t11.*t298-t5.*t8.*t323-t5.*t11.*t349,t8.*(t755+t756+t757+t758+t759+t761+t762+t763+t764+t765+t766+t767+t768-t150.*t401-t199.*t379-t3.*t705+t379.*t471-t379.*t474+t189.*t677-t401.*t467-t210.*t681-t218.*t682-t239.*t677+t335.*t677-t5.*t8.*t595-t5.*t8.*t611-t5.*t8.*t625)-t11.*(t769+t770+t771+t772+t773+t774+t775+t776+t778+t779+t780+t781+t782-t179.*t387-t199.*t371-t3.*t701+t371.*t471-t371.*t474-t387.*t461-t221.*t677-t242.*t677+t260.*t677-t270.*t677-t274.*t681-t5.*t11.*t639-t5.*t11.*t644-t5.*t11.*t689),t8.*(t755+t756+t757+t758+t759+t761+t762+t763+t764+t765+t766+t767+t768-t150.*t401-t3.*t705-t379.*t474-t401.*t467-t210.*t681-t218.*t682-t239.*t677-t5.*t8.*t595-t5.*t8.*t611-t5.*t8.*t625)-t11.*(t769+t770+t771+t772+t773+t774+t775+t776+t778+t779+t780+t781+t782-t179.*t387-t3.*t701-t371.*t474-t387.*t461-t221.*t677-t270.*t677-t274.*t681-t5.*t11.*t639-t5.*t11.*t644-t5.*t11.*t689),t3.*(-t835-t836-t839-t840+t862+t863+t864+t865+t866+t867+t868+t869+t135.*t371+t221.*t379+t3.*t838-t274.*t664+t282.*t664+t5.*t8.*t294+t5.*t11.*t298)+t5.*t11.*(t755+t756+t758+t759+t761+t762+t763+t764+t766+t767+t768-t150.*t401-t3.*t705-t401.*t467-t210.*t681-t218.*t682-t5.*t8.*t595-t5.*t8.*t611-t5.*t8.*t625)+t5.*t8.*(t769+t770+t771+t772+t775+t776+t778+t779+t780+t781+t782-t179.*t387-t3.*t701-t387.*t461-t221.*t677-t274.*t681-t5.*t11.*t639-t5.*t11.*t644-t5.*t11.*t689),t16.*(t756+t758+t763+t764+t766+t768-t150.*t401-t3.*t705-t401.*t467-t218.*t682-t5.*t8.*t595-t5.*t8.*t611)-t29.*(t769+t770+t775+t776+t779+t781+t782-t179.*t387-t3.*t701-t274.*t681-t5.*t11.*t639-t5.*t11.*t644)+t5.*t9.*(-t836-t839-t840+t862+t863+t864+t865+t866+t867+t868+t869-t274.*t664),-t265.*(-t764-t768+t150.*t401+t3.*t705+t5.*t8.*t595)-t277.*(t769+t775+t776+t781-t5.*t11.*t639)+t73.*(-t840+t862+t864+t867+t868),t841+t842+t843+t844+t845+t846+t847+t848-t16.*t349-t29.*t355+t165.*t421+t189.*t421-t206.*t416-t210.*t421-t221.*t416-t218.*t429+t233.*t421-t242.*t416-t239.*t421+t260.*t416-t257.*t421-t270.*t416-t274.*t416+t280.*t416+t335.*t421+t416.*t440-t5.*t9.*t431-t5.*t9.*t433,t11.*(t783+t784+t785+t786+t787+t788+t789+t790+t791+t792+t793+t794-t179.*t421-t199.*t421-t185.*t697-t421.*t461+t421.*t471-t421.*t474-t232.*t697+t242.*t694-t260.*t694-t280.*t694-t282.*t694-t5.*t9.*t698)+t8.*(t795+t796+t797+t798+t799+t800+t801+t802+t803+t804+t805+t806+t807-t179.*t416-t199.*t416-t416.*t461+t189.*t694+t416.*t471-t416.*t474-t210.*t694-t218.*t697-t239.*t694+t335.*t694-t5.*t9.*t705),t11.*(t783+t784+t785+t786+t787+t788+t789+t790+t791+t792+t793+t794-t179.*t421-t185.*t697-t421.*t461-t421.*t474-t232.*t697-t280.*t694-t282.*t694-t5.*t9.*t698)+t8.*(t795+t796+t797+t798+t799+t800+t801+t802+t803+t804+t805+t806+t807-t179.*t416-t416.*t461-t416.*t474-t210.*t694-t218.*t697-t239.*t694-t5.*t9.*t705),-t3.*(t841+t842+t843+t844+t845+t846+t847+t848-t16.*t349-t29.*t355-t210.*t421-t221.*t416-t218.*t429-t274.*t416-t5.*t9.*t431-t5.*t9.*t433)-t5.*t8.*(t783+t784+t786+t787+t788+t789+t790+t791+t792+t794-t179.*t421-t185.*t697-t421.*t461-t232.*t697-t282.*t694-t5.*t9.*t698)+t5.*t11.*(t795+t797+t798+t799+t800+t802+t803+t804+t805+t806+t807-t179.*t416-t416.*t461-t210.*t694-t218.*t697-t5.*t9.*t705),t29.*(t783+t784+t786+t789+t790+t791+t792+t794-t179.*t421-t185.*t697-t232.*t697-t5.*t9.*t698)+t16.*(t795+t797+t800+t802+t803+t804+t805+t806+t807-t179.*t416-t218.*t697-t5.*t9.*t705)-t5.*t9.*(t842+t844+t845+t846+t847+t848-t16.*t349-t29.*t355-t218.*t429-t274.*t416-t5.*t9.*t431-t5.*t9.*t433),t277.*(t783+t786+t789-t185.*t697-t5.*t9.*t698)-t73.*(t842+t844+t845+t846-t5.*t9.*t431)+t265.*(t797+t800+t802+t805-t5.*t9.*t705),t849+t850+t851+t852+t853-t73.*t431-t135.*t436-t156.*t436-t165.*t436-t185.*t437-t189.*t436+t221.*t437-t232.*t437-t233.*t436+t239.*t436+t257.*t436-t260.*t437-t280.*t437-t282.*t437-t312.*t436-t335.*t436-t437.*t440+t242.*(t434-t439)+t270.*(t434-t439)+(t82-t203).*(t434-t439),-t11.*(t810+t811+t812+t813+t814+t815+t816+t817+t818-t179.*t436-t199.*t436-t436.*t461-t265.*t639+t436.*t471-t436.*t474-t277.*t649-t221.*t707-t242.*t707+t260.*t707-t270.*t707-t274.*t707)+t8.*(t808+t809+t179.*t437+t199.*t437-t73.*t705+t135.*t707+t156.*t707+t189.*t707+t437.*t461+t437.*t474+t233.*t707+t312.*t707+t335.*t707-t150.*(t434-t439)-t172.*(t434-t439)-t193.*(t434-t439)-t467.*(t434-t439)-t471.*(t434-t439)-t210.*(t706-t708)-t218.*(t706-t708)-t239.*(t706-t708)),-t11.*(t810+t811+t812+t813+t814+t815+t816+t817+t818-t179.*t436-t436.*t461-t265.*t639-t436.*t474-t277.*t649-t221.*t707-t270.*t707-t274.*t707)+t8.*(t808+t809+t854+t855+t856+t857+t858-t150.*t437-t172.*t437-t193.*t437-t73.*t705-t437.*t467-t210.*t707-t218.*t707-t239.*t707+t474.*(t434-t439)+t233.*(t706-t708)),t3.*(-t849-t850-t851-t852-t853+t870+t871+t872+t873+t874+t135.*t436+t282.*t437-t221.*(t434-t439))+t5.*t11.*(t808+t809+t854+t855+t856+t857+t858-t150.*t437-t172.*t437-t73.*t705-t437.*t467-t210.*t707-t218.*t707)+t5.*t8.*(t810+t811+t812+t813+t814+t815+t817-t179.*t436-t436.*t461-t265.*t639-t277.*t649-t221.*(t706-t708)-t274.*(t706-t708)),t16.*(t808+t809+t854+t856+t858-t150.*t437-t73.*t705-t437.*t467-t218.*t707)-t29.*(t810+t812+t813+t814+t817-t179.*t436-t265.*t639-t277.*t649-t274.*t707)+t5.*t9.*(-t849-t850-t852-t853+t870+t871+t872+t873+t874),t265.*(t808+t809+t858-t150.*t437-t73.*t705)-t277.*(t813+t814+t817-t265.*t639-t277.*t649)+t73.*(-t849-t853+t871+t872+t873)],[6,6]);
end

function CFG = CFG_vec_diff(th1,th2,th3,th4,th5,th6,thDot1,thDot2,thDot3,thDot4,thDot5,thDot6)
%CFG_VEC_DIFF
%    CFG = CFG_VEC_DIFF(TH1,TH2,TH3,TH4,TH5,TH6,THDOT1,THDOT2,THDOT3,THDOT4,THDOT5,THDOT6)

%    This function was generated by the Symbolic Math Toolbox version 7.0.
%    21-Nov-2018 16:22:39

t2 = sin(th1);
t3 = cos(th4);
t4 = sin(th4);
t5 = t2.*t4;
t6 = th2+th3;
t7 = cos(t6);
t8 = cos(th1);
t9 = t3.*t7.*t8;
t10 = t5+t9;
t11 = cos(th5);
t12 = sin(t6);
t13 = sin(th5);
t14 = thDot1.^2;
t15 = sin(th6);
t16 = t2.*t3;
t44 = t4.*t7.*t8;
t17 = t16-t44;
t18 = cos(th6);
t19 = t10.*t11;
t43 = t8.*t12.*t13;
t20 = t19-t43;
t21 = t4.*t7.*thDot2.*thDot5;
t22 = t4.*t7.*thDot3.*thDot5;
t23 = t3.*t12.*thDot4.*thDot5;
t24 = t7.*t13;
t25 = t3.*t11.*t12;
t26 = t24+t25;
t27 = thDot2+thDot3;
t28 = t8.*t27;
t29 = t3.*t8;
t30 = t2.*t4.*t7;
t31 = t29+t30;
t32 = t31.*thDot5;
t37 = t2.*t12.*thDot4;
t33 = t28-t37;
t34 = t7.*thDot4;
t35 = t4.*t12.*thDot5;
t36 = t34+t35-thDot1;
t38 = t4.*t8;
t51 = t2.*t3.*t7;
t39 = t38-t51;
t40 = t13.*t39;
t72 = t2.*t11.*t12;
t41 = t40-t72;
t42 = t41.*thDot6;
t45 = t17.*t18.*3.37770948362828e-2;
t46 = t10.*t13.*7.403989170917124e-2;
t47 = t15.*t17.*1.095176343335877e-3;
t48 = t18.*t20.*1.095176343335877e-3;
t49 = t8.*t11.*t12.*7.403989170917124e-2;
t103 = t15.*t20.*3.37770948362828e-2;
t50 = t45+t46+t47+t48+t49-t103;
t52 = t11.*t39;
t53 = t2.*t12.*t13;
t54 = t52+t53;
t55 = t17.*thDot5;
t56 = t10.*t13;
t57 = t8.*t11.*t12;
t58 = t56+t57;
t59 = t58.*thDot6;
t60 = t2.*t27;
t61 = t8.*t12.*thDot4;
t62 = t55+t59+t60+t61;
t63 = t7.*t11;
t79 = t3.*t12.*t13;
t64 = t63-t79;
t65 = t64.*thDot6;
t66 = t34+t35+t65-thDot1;
t67 = t18.*t54.*1.095176343335877e-3;
t68 = t18.*t31.*3.37770948362828e-2;
t69 = t13.*t39.*7.403989170917124e-2;
t70 = t15.*t31.*1.095176343335877e-3;
t115 = t15.*t54.*3.37770948362828e-2;
t116 = t2.*t11.*t12.*7.403989170917124e-2;
t71 = t67+t68+t69+t70-t115-t116;
t73 = t28+t32-t37+t42;
t74 = t15.*t26.*3.37770948362828e-2;
t75 = t7.*t11.*7.403989170917124e-2;
t76 = t4.*t12.*t18.*3.37770948362828e-2;
t77 = t4.*t12.*t15.*1.095176343335877e-3;
t101 = t18.*t26.*1.095176343335877e-3;
t102 = t3.*t12.*t13.*7.403989170917124e-2;
t78 = t74+t75+t76+t77-t101-t102;
t80 = t4.*t12.*1.986944558488843e-4;
t81 = t7.*t13.*1.052644841177257e-4;
t82 = t3.*t11.*t12.*1.052644841177257e-4;
t83 = t80+t81+t82;
t84 = thDot2.^2;
t85 = cos(th2);
t86 = thDot3.^2;
t87 = thDot4.^2;
t88 = cos(th3);
t89 = sin(th2);
t90 = sin(th3);
t91 = t7.^2;
t92 = t12.^2;
t93 = t10.*t13.*2.061478095729509e-3;
t94 = t8.*t11.*t12.*2.061478095729509e-3;
t95 = t3.*t8.*1.986944558488843e-4;
t96 = t2.*t4.*t7.*1.986944558488843e-4;
t97 = t2.*t3.*t7.*t11.*1.052644841177257e-4;
t246 = t2.*t12.*t13.*1.052644841177257e-4;
t247 = t4.*t8.*t11.*1.052644841177257e-4;
t98 = t95+t96+t97-t246-t247;
t99 = t12.*thDot2.*thDot4;
t100 = t12.*thDot3.*thDot4;
t104 = t28+t32-t37;
t105 = t4.*t7.*t8.*1.442959919441252e-3;
t106 = t8.*t12.*t13.*1.268225234578345e-3;
t217 = t2.*t3.*1.442959919441252e-3;
t218 = t10.*t11.*1.268225234578345e-3;
t107 = t93+t94+t105+t106-t217-t218;
t108 = t55+t60+t61;
t109 = -t34+thDot1;
t110 = t2.*t4.*1.294017156131404e-3;
t111 = t3.*t7.*t8.*1.294017156131404e-3;
t112 = t4.*t7.*t8.*3.439231171461361e-3;
t205 = t2.*t3.*3.439231171461361e-3;
t206 = t8.*t12.*1.497952838441835e-1;
t113 = t110+t111+t112-t205-t206;
t114 = t60+t61;
t117 = t11.*t12.*thDot2.*thDot6;
t118 = t11.*t12.*thDot3.*thDot6;
t119 = t7.*t13.*thDot5.*thDot6;
t120 = t3.*t7.*t13.*thDot2.*thDot6;
t121 = t3.*t7.*t13.*thDot3.*thDot6;
t122 = t3.*t11.*t12.*thDot5.*thDot6;
t212 = t4.*t12.*t13.*thDot4.*thDot6;
t123 = -t21-t22-t23+t99+t100+t117+t118+t119+t120+t121+t122-t212;
t124 = t108.*t109;
t125 = t114.*thDot1;
t126 = t36.*t114;
t127 = t2.*t27.*thDot1;
t128 = t7.*t11.*2.061478095729509e-3;
t129 = t7.*t13.*1.268225234578345e-3;
t130 = t3.*t11.*t12.*1.268225234578345e-3;
t214 = t4.*t12.*1.442959919441252e-3;
t215 = t3.*t12.*t13.*2.061478095729509e-3;
t131 = t128+t129+t130-t214-t215;
t132 = t50.*t73;
t242 = t62.*t71;
t133 = t132-t242;
t134 = t21+t22+t23-t99-t100;
t135 = t3.*t8.*1.442959919441252e-3;
t136 = t11.*t39.*1.268225234578345e-3;
t137 = t2.*t4.*t7.*1.442959919441252e-3;
t138 = t2.*t11.*t12.*2.061478095729509e-3;
t139 = t2.*t12.*t13.*1.268225234578345e-3;
t216 = t13.*t39.*2.061478095729509e-3;
t140 = t135+t136+t137+t138+t139-t216;
t141 = t8.*thDot2;
t142 = t8.*thDot3;
t143 = t3.*t8.*thDot5;
t144 = t2.*t4.*t7.*thDot5;
t145 = -t37+t141+t142+t143+t144;
t146 = t7.*t11.*thDot5.*1.052644841177257e-4;
t147 = t4.*t7.*thDot2.*1.986944558488843e-4;
t148 = t4.*t7.*thDot3.*1.986944558488843e-4;
t149 = t3.*t12.*thDot4.*1.986944558488843e-4;
t150 = t3.*t7.*t11.*thDot2.*1.052644841177257e-4;
t151 = t3.*t7.*t11.*thDot3.*1.052644841177257e-4;
t255 = t12.*t13.*thDot2.*1.052644841177257e-4;
t256 = t12.*t13.*thDot3.*1.052644841177257e-4;
t257 = t4.*t11.*t12.*thDot4.*1.052644841177257e-4;
t258 = t3.*t12.*t13.*thDot5.*1.052644841177257e-4;
t152 = t146+t147+t148+t149+t150+t151-t255-t256-t257-t258;
t153 = t2.*t4.*t11.*1.052644841177257e-4;
t154 = t4.*t7.*t8.*1.986944558488843e-4;
t155 = t3.*t7.*t8.*t11.*1.052644841177257e-4;
t203 = t2.*t3.*1.986944558488843e-4;
t204 = t8.*t12.*t13.*1.052644841177257e-4;
t156 = t153+t154+t155-t203-t204;
t157 = t2.*thDot2;
t158 = t2.*thDot3;
t159 = t2.*t3.*thDot5;
t254 = t4.*t7.*t8.*thDot5;
t160 = t61+t157+t158+t159-t254;
t161 = t7.*1.497952838441835e-1;
t162 = t4.*t12.*3.439231171461361e-3;
t163 = t3.*t12.*1.294017156131404e-3;
t164 = t161+t162+t163;
t165 = t8.*t85.*1.395740012982637e-1;
t166 = t8.*t89.*3.219519910626345e-4;
t267 = t2.*4.581283258289218e-4;
t167 = t165+t166-t267;
t168 = t2.*4.807572428874383e-3;
t169 = t7.*t8.*3.689996292735745e-2;
t170 = t8.*t12.*4.915167130564437e-3;
t171 = t8.*t89.*t90.*6.992065648397489e-2;
t264 = t8.*t85.*t88.*6.992065648397489e-2;
t172 = t168+t169+t170+t171-t264;
t173 = t7.*4.915167130564437e-3;
t174 = t12.*3.302069355661744e-2;
t175 = t173+t174;
t176 = t3.*t8.*3.439231171461361e-3;
t177 = t2.*t3.*t7.*1.294017156131404e-3;
t178 = t2.*t4.*t7.*3.439231171461361e-3;
t208 = t2.*t12.*1.497952838441835e-1;
t209 = t4.*t8.*1.294017156131404e-3;
t179 = t176+t177+t178-t208-t209;
t180 = t85.*3.219519910626345e-4;
t181 = t89.*1.395740012982637e-1;
t182 = t180-t181;
t183 = t33.*thDot1;
t184 = t33.*t36;
t185 = t66.*t104;
t186 = t8.*t27.*thDot1;
t187 = t15.*t17.*6.715374732587727e-4;
t188 = t18.*t20.*6.715374732587727e-4;
t189 = t187+t188;
t190 = t15.*t17;
t191 = t18.*t20;
t192 = t190+t191;
t193 = t10.*t13.*6.715374732587727e-4;
t194 = t8.*t11.*t12.*6.715374732587727e-4;
t195 = t193+t194;
t196 = t15.*t20.*3.565423831595737e-4;
t200 = t17.*t18.*3.565423831595737e-4;
t197 = t196-t200;
t198 = t15.*t20;
t424 = t17.*t18;
t199 = t198-t424;
t201 = t2.*3.038635549296489e-3;
t202 = t8.*4.185385434780744e-3-t201;
t207 = t33.*t113;
t210 = t114.*t179;
t211 = t207+t210;
t213 = t50.*t123.*1.139953928995173;
t219 = t104.*t107;
t220 = t108.*t140;
t221 = t219+t220;
t222 = t104.*t109;
t223 = t8.*4.581283258289218e-4;
t224 = t2.*t85.*1.395740012982637e-1;
t225 = t2.*t89.*3.219519910626345e-4;
t226 = t223+t224+t225;
t227 = t2.*t12.*4.915167130564437e-3;
t228 = t2.*t7.*3.689996292735745e-2;
t229 = t2.*t89.*t90.*6.992065648397489e-2;
t261 = t8.*4.807572428874383e-3;
t262 = t2.*t85.*t88.*6.992065648397489e-2;
t230 = t227+t228+t229-t261-t262;
t260 = t8.*t27.*t109;
t282 = t36.*t73;
t231 = t183+t184+t185+t186+t222-t260-t282;
t232 = t8.*thDot1.*thDot2;
t233 = t8.*thDot1.*thDot3;
t234 = t7.*t8.*thDot2.*thDot4;
t235 = t7.*t8.*thDot3.*thDot4;
t236 = t3.*t8.*thDot1.*thDot5;
t237 = t2.*t4.*t7.*thDot1.*thDot5;
t238 = t4.*t8.*t12.*thDot2.*thDot5;
t239 = t4.*t8.*t12.*thDot3.*thDot5;
t284 = t2.*t4.*thDot4.*thDot5;
t285 = t2.*t12.*thDot1.*thDot4;
t286 = t3.*t7.*t8.*thDot4.*thDot5;
t240 = t232+t233+t234+t235+t236+t237+t238+t239-t284-t285-t286;
t241 = t83.*t240.*1.139953928995173;
t243 = t66.*t71;
t288 = t73.*t78;
t244 = t243-t288;
t245 = t66.*t244.*1.139953928995173;
t248 = t36.*t98;
t289 = t83.*t145;
t249 = t248-t289;
t250 = t36.*t249.*1.139953928995173;
t251 = t8.*3.038635549296489e-3;
t252 = t2.*4.185385434780744e-3;
t253 = t251+t252;
t259 = t152.*t160.*1.139953928995173;
t263 = t2.*t27.*t230;
t265 = t8.*t27.*t172;
t266 = t263+t265;
t268 = t8.*t167.*thDot2;
t269 = t2.*t226.*thDot2;
t270 = t268+t269;
t271 = t134.*t156.*1.139953928995173;
t272 = t114.*t211.*1.900321864457165e1;
t273 = t104.*t131;
t274 = t36.*t140;
t275 = t273+t274;
t276 = t36.*t275.*1.994855465224146;
t277 = t108.*t221.*1.994855465224146;
t278 = t109.*t179;
t279 = t33.*t164;
t280 = t278+t279;
t281 = t109.*t280.*1.900321864457165e1;
t283 = t78.*t231.*1.139953928995173;
t287 = t107.*t134.*1.994855465224146;
t290 = t183+t186-t260;
t291 = t164.*t290.*1.900321864457165e1;
t292 = t4.*t8.*t14.*1.865719029901695e-3;
t293 = t4.*t8.*t87.*t92.*1.865719029901695e-3;
t294 = t2.*t14.*t85.*t88.*1.547905453732908;
t295 = t2.*t84.*t85.*t88.*1.547905453732908;
t296 = t2.*t85.*t86.*t88.*1.547905453732908;
t297 = t7.*t8.*thDot1.*thDot2.*1.890029125090016;
t298 = t7.*t8.*thDot1.*thDot3.*1.890029125090016;
t299 = t4.*t8.*t87.*t91.*1.865719029901695e-3;
t300 = t2.*t3.*t91.*thDot1.*thDot4.*3.73143805980339e-3;
t301 = t2.*t3.*t92.*thDot1.*thDot4.*3.73143805980339e-3;
t302 = t2.*t4.*t12.*thDot2.*thDot4.*3.73143805980339e-3;
t303 = t2.*t4.*t12.*thDot3.*thDot4.*3.73143805980339e-3;
t304 = t8.*t85.*t90.*thDot1.*thDot2.*3.095810907465815;
t305 = t8.*t88.*t89.*thDot1.*thDot2.*3.095810907465815;
t306 = t8.*t85.*t90.*thDot1.*thDot3.*3.095810907465815;
t307 = t8.*t88.*t89.*thDot1.*thDot3.*3.095810907465815;
t308 = t2.*t85.*t88.*thDot2.*thDot3.*3.095810907465815;
t309 = t7.*t11.*2.923071757101621e-3;
t409 = t3.*t12.*t13.*2.923071757101621e-3;
t310 = t309-t409;
t311 = t7.*t13.*2.923071757101621e-3;
t312 = t3.*t11.*t12.*2.923071757101621e-3;
t313 = t311+t312;
t314 = t183+t184+t186+t222-t260;
t315 = t3.*t8.*6.280147091832467e-4;
t316 = t2.*t4.*t7.*6.280147091832467e-4;
t317 = t315+t316;
t318 = t11.*t39.*2.923071757101621e-3;
t319 = t2.*t12.*t13.*2.923071757101621e-3;
t320 = t318+t319;
t321 = t13.*t39.*2.923071757101621e-3;
t323 = t2.*t11.*t12.*2.923071757101621e-3;
t322 = t321-t323;
t324 = t7.*t11.*6.715374732587727e-4;
t413 = t3.*t12.*t13.*6.715374732587727e-4;
t325 = t324-t413;
t326 = t15.*t26.*3.565423831595737e-4;
t327 = t4.*t12.*t18.*3.565423831595737e-4;
t328 = t326+t327;
t329 = t18.*t31;
t427 = t15.*t54;
t330 = t329-t427;
t331 = t18.*t26.*6.715374732587727e-4;
t414 = t4.*t12.*t15.*6.715374732587727e-4;
t332 = t331-t414;
t333 = t18.*t54;
t334 = t15.*t31;
t335 = t333+t334;
t336 = t66.*t108;
t345 = t36.*t62;
t346 = t2.*t27.*t109;
t337 = t124+t125+t126+t127+t336-t345-t346;
t338 = t36.*t107;
t387 = t108.*t131;
t339 = t338-t387;
t340 = t98.*t134.*1.139953928995173;
t341 = t50.*t66;
t392 = t62.*t78;
t602 = t341-t392;
t342 = t66.*t602.*1.139953928995173;
t343 = t109.*t113;
t393 = t114.*t164;
t344 = t343-t393;
t347 = t78.*t337.*1.139953928995173;
t348 = t73.*t133.*1.139953928995173;
t349 = t134.*t140.*1.994855465224146;
t350 = t36.*t156;
t351 = t83.*t160;
t352 = t350+t351;
t353 = t2.*thDot1.*thDot2;
t354 = t2.*thDot1.*thDot3;
t355 = t2.*t3.*thDot1.*thDot5;
t356 = t4.*t8.*thDot4.*thDot5;
t357 = t8.*t12.*thDot1.*thDot4;
t358 = t2.*t7.*thDot2.*thDot4;
t359 = t2.*t7.*thDot3.*thDot4;
t360 = t2.*t4.*t12.*thDot2.*thDot5;
t361 = t2.*t4.*t12.*thDot3.*thDot5;
t395 = t4.*t7.*t8.*thDot1.*thDot5;
t396 = t2.*t3.*t7.*thDot4.*thDot5;
t362 = t353+t354+t355+t356+t357+t358+t359+t360+t361-t395-t396;
t363 = t83.*t362.*1.139953928995173;
t364 = t2.*t4.*t14.*1.865719029901695e-3;
t365 = t8.*t12.*t14.*9.450145625450081e-1;
t366 = t8.*t12.*t84.*9.450145625450081e-1;
t367 = t8.*t12.*t86.*9.450145625450081e-1;
t368 = t2.*t4.*t87.*t91.*1.865719029901695e-3;
t369 = t2.*t4.*t87.*t92.*1.865719029901695e-3;
t370 = t3.*t7.*t8.*t14.*1.865719029901695e-3;
t371 = t3.*t7.*t8.*t84.*1.865719029901695e-3;
t372 = t3.*t7.*t8.*t86.*1.865719029901695e-3;
t373 = t3.*t7.*t8.*t87.*1.865719029901695e-3;
t374 = t8.*t14.*t89.*t90.*1.547905453732908;
t375 = t8.*t84.*t89.*t90.*1.547905453732908;
t376 = t8.*t86.*t89.*t90.*1.547905453732908;
t377 = t2.*t7.*thDot1.*thDot2.*1.890029125090016;
t378 = t2.*t7.*thDot1.*thDot3.*1.890029125090016;
t379 = t8.*t12.*thDot2.*thDot3.*1.890029125090016;
t380 = t3.*t7.*t8.*thDot2.*thDot3.*3.73143805980339e-3;
t381 = t2.*t85.*t90.*thDot1.*thDot2.*3.095810907465815;
t382 = t2.*t88.*t89.*thDot1.*thDot2.*3.095810907465815;
t383 = t2.*t85.*t90.*thDot1.*thDot3.*3.095810907465815;
t384 = t2.*t88.*t89.*thDot1.*thDot3.*3.095810907465815;
t385 = t8.*t89.*t90.*thDot2.*thDot3.*3.095810907465815;
t386 = t2.*t14.*4.163551055963717e-2;
t388 = t172.*thDot1;
t389 = t2.*t27.*t175;
t390 = t388+t389;
t391 = t390.*thDot1.*4.38483060303202;
t394 = t124+t125+t126+t127-t346;
t397 = t125+t127-t346;
t398 = t164.*t397.*1.900321864457165e1;
t399 = t8.*t27.*t266.*4.38483060303202;
t400 = t2.*t89.*thDot1.*thDot2.*1.430741738206701e1;
t401 = t2.*t27.*t175.*thDot1.*4.38483060303202;
t402 = t8.*t14.*4.163551055963717e-2;
t403 = t230.*thDot1;
t437 = t8.*t27.*t175;
t404 = t403-t437;
t405 = t2.*t14.*t85.*7.153708691033507;
t406 = t2.*t84.*t85.*7.153708691033507;
t407 = t8.*t89.*thDot1.*thDot2.*1.430741738206701e1;
t408 = t8.*t27.*t175.*thDot1.*4.38483060303202;
t410 = t15.*t26;
t411 = t4.*t12.*t18;
t412 = t410+t411;
t415 = t18.*t26;
t417 = t4.*t12.*t15;
t416 = t415-t417;
t418 = t18.*t54.*6.715374732587727e-4;
t419 = t15.*t31.*6.715374732587727e-4;
t420 = t418+t419;
t421 = t13.*t39.*6.715374732587727e-4;
t428 = t2.*t11.*t12.*6.715374732587727e-4;
t422 = t421-t428;
t423 = t18.*t31.*3.565423831595737e-4;
t426 = t15.*t54.*3.565423831595737e-4;
t425 = t423-t426;
t429 = t8.*t14.*1.25890039900759e-2;
t430 = t167.*thDot1;
t431 = t2.*t182.*thDot2;
t432 = t430+t431;
t434 = t71.*t123.*1.139953928995173;
t435 = t145.*t152.*1.139953928995173;
t436 = t36.*t352.*1.139953928995173;
t486 = t33.*t211.*1.900321864457165e1;
t487 = t36.*t339.*1.994855465224146;
t488 = t104.*t221.*1.994855465224146;
t489 = t109.*t344.*1.900321864457165e1;
t490 = t131.*t394.*1.994855465224146;
t491 = t8.*t14.*t85.*7.153708691033507;
t492 = t8.*t84.*t85.*7.153708691033507;
t493 = t12.*t27.*t179.*thDot4.*1.900321864457165e1;
t494 = t8.*t14.*t85.*t88.*1.547905453732908;
t495 = t8.*t84.*t85.*t88.*1.547905453732908;
t496 = t8.*t85.*t86.*t88.*1.547905453732908;
t497 = t3.*t8.*t91.*thDot1.*thDot4.*3.73143805980339e-3;
t498 = t3.*t8.*t92.*thDot1.*thDot4.*3.73143805980339e-3;
t499 = t2.*t3.*t12.*thDot1.*thDot2.*3.73143805980339e-3;
t500 = t2.*t3.*t12.*thDot1.*thDot3.*3.73143805980339e-3;
t501 = t2.*t4.*t7.*thDot1.*thDot4.*3.73143805980339e-3;
t502 = t4.*t8.*t12.*thDot2.*thDot4.*3.73143805980339e-3;
t503 = t4.*t8.*t12.*thDot3.*thDot4.*3.73143805980339e-3;
t504 = t8.*t85.*t88.*thDot2.*thDot3.*3.095810907465815;
t738 = t432.*thDot1.*3.812773007925995e1;
t739 = t8.*t270.*thDot2.*3.812773007925995e1;
t740 = t2.*t182.*thDot1.*thDot2.*3.812773007925995e1;
t433 = t340+t342+t347+t348+t349+t363+t364+t365+t366+t367+t368+t369+t370+t371+t372+t373+t374+t375+t376+t377+t378+t379+t380+t381+t382+t383+t384+t385+t386+t391+t398+t399+t400+t401+t429-t434-t435-t436-t486-t487-t488-t489-t490-t491-t492-t493-t494-t495-t496-t497-t498-t499-t500-t501-t502-t503-t504-t738-t739-t740;
t439 = t131.*t314.*1.994855465224146;
t443 = t404.*thDot1.*4.38483060303202;
t444 = t62.*t133.*1.139953928995173;
t445 = t2.*t27.*t266.*4.38483060303202;
t447 = t2.*t12.*t14.*9.450145625450081e-1;
t448 = t2.*t12.*t84.*9.450145625450081e-1;
t449 = t2.*t12.*t86.*9.450145625450081e-1;
t450 = t2.*t3.*t7.*t14.*1.865719029901695e-3;
t451 = t2.*t3.*t7.*t84.*1.865719029901695e-3;
t452 = t2.*t3.*t7.*t86.*1.865719029901695e-3;
t453 = t2.*t3.*t7.*t87.*1.865719029901695e-3;
t454 = t12.*t27.*t113.*thDot4.*1.900321864457165e1;
t455 = t2.*t14.*t89.*t90.*1.547905453732908;
t456 = t2.*t84.*t89.*t90.*1.547905453732908;
t457 = t2.*t86.*t89.*t90.*1.547905453732908;
t458 = t2.*t12.*thDot2.*thDot3.*1.890029125090016;
t459 = t3.*t8.*t12.*thDot1.*thDot2.*3.73143805980339e-3;
t460 = t3.*t8.*t12.*thDot1.*thDot3.*3.73143805980339e-3;
t461 = t4.*t7.*t8.*thDot1.*thDot4.*3.73143805980339e-3;
t462 = t2.*t3.*t7.*thDot2.*thDot3.*3.73143805980339e-3;
t463 = t2.*t89.*t90.*thDot2.*thDot3.*3.095810907465815;
t918 = t2.*t14.*5.164630050170653e-3;
t438 = t213+t241+t245+t250+t259+t271+t272+t276+t277+t281+t283+t287+t291+t292+t293+t294+t295+t296+t297+t298+t299+t300+t301+t302+t303+t304+t305+t306+t307+t308+t402+t405+t406+t407+t408-t439-t443-t444-t445-t447-t448-t449-t450-t451-t452-t453-t454-t455-t456-t457-t458-t459-t460-t461-t462-t463-t918;
t440 = t226.*thDot1;
t505 = t8.*t182.*thDot2;
t441 = t440-t505;
t442 = t441.*thDot1.*3.812773007925995e1;
t446 = t2.*t270.*thDot2.*3.812773007925995e1;
t464 = t8.*t14.*1.960554684600962e-3;
t465 = t2.*t14.*t85.*3.074667945623095e-1;
t466 = t2.*t84.*t85.*3.074667945623095e-1;
t467 = t4.*t8.*t14.*6.784571152745185e-4;
t468 = t8.*t89.*thDot1.*thDot2.*6.149335891246189e-1;
t469 = t4.*t8.*t87.*t92.*6.784571152745185e-4;
t470 = t2.*t14.*t85.*t88.*7.970632707682899e-2;
t471 = t2.*t84.*t85.*t88.*7.970632707682899e-2;
t472 = t2.*t85.*t86.*t88.*7.970632707682899e-2;
t473 = t7.*t8.*thDot1.*thDot2.*6.872973301135055e-1;
t474 = t7.*t8.*thDot1.*thDot3.*6.872973301135055e-1;
t475 = t4.*t8.*t87.*t91.*6.784571152745185e-4;
t476 = t2.*t3.*t91.*thDot1.*thDot4.*1.356914230549037e-3;
t477 = t2.*t3.*t92.*thDot1.*thDot4.*1.356914230549037e-3;
t478 = t2.*t4.*t12.*thDot2.*thDot4.*1.356914230549037e-3;
t479 = t2.*t4.*t12.*thDot3.*thDot4.*1.356914230549037e-3;
t480 = t8.*t85.*t90.*thDot1.*thDot2.*1.59412654153658e-1;
t481 = t8.*t88.*t89.*thDot1.*thDot2.*1.59412654153658e-1;
t482 = t8.*t85.*t90.*thDot1.*thDot3.*1.59412654153658e-1;
t483 = t8.*t88.*t89.*thDot1.*thDot3.*1.59412654153658e-1;
t484 = t2.*t85.*t88.*thDot2.*thDot3.*1.59412654153658e-1;
t485 = t8.*t14.*5.164630050170653e-3;
t921 = t2.*t14.*1.25890039900759e-2;
t922 = t8.*t182.*thDot1.*thDot2.*3.812773007925995e1;
t506 = t213+t241+t245+t250+t259+t271+t272+t276+t277+t281+t283+t287+t291+t292+t293+t294+t295+t296+t297+t298+t299+t300+t301+t302+t303+t304+t305+t306+t307+t308+t402+t405+t406+t407+t408-t439+t442-t443-t444-t445+t446-t447-t448-t449-t450-t451-t452-t453-t454-t455-t456-t457-t458-t459-t460-t461-t462-t463-t921-t922;
t507 = t8.*t14.*3.807418306592183e-2;
t508 = t2.*t14.*t85.*5.971038255043736;
t509 = t2.*t84.*t85.*5.971038255043736;
t510 = t8.*t89.*thDot1.*thDot2.*1.194207651008747e1;
t511 = t2.*t4.*1.557550994534973e-1;
t512 = t3.*t7.*t8.*1.557550994534973e-1;
t513 = t511+t512;
t514 = t2.*t3.*1.557550994534973e-1;
t517 = t4.*t7.*t8.*1.557550994534973e-1;
t515 = t514-t517;
t516 = t7.*t8.*t12.*2.36837910197578e-2;
t518 = t8.*t14.*4.310799465649219e-3;
t519 = t2.*t14.*3.807418306592183e-2;
t520 = t2.*t89.*thDot1.*thDot2.*1.194207651008747e1;
t521 = t4.*t8.*1.557550994534973e-1;
t527 = t2.*t3.*t7.*1.557550994534973e-1;
t522 = t521-t527;
t523 = t3.*t8.*1.557550994534973e-1;
t524 = t2.*t4.*t7.*1.557550994534973e-1;
t525 = t523+t524;
t526 = t2.*t7.*t12.*2.36837910197578e-2;
t528 = t8.*t14.*2.219760847427988e-4;
t529 = t2.*t14.*1.960554684600962e-3;
t530 = t2.*t4.*t14.*6.784571152745185e-4;
t531 = t8.*t12.*t14.*3.436486650567527e-1;
t532 = t8.*t12.*t84.*3.436486650567527e-1;
t533 = t8.*t12.*t86.*3.436486650567527e-1;
t534 = t2.*t4.*t87.*t91.*6.784571152745185e-4;
t535 = t2.*t89.*thDot1.*thDot2.*6.149335891246189e-1;
t536 = t2.*t4.*t87.*t92.*6.784571152745185e-4;
t537 = t3.*t7.*t8.*t14.*6.784571152745185e-4;
t538 = t3.*t7.*t8.*t84.*6.784571152745185e-4;
t539 = t3.*t7.*t8.*t86.*6.784571152745185e-4;
t540 = t3.*t7.*t8.*t87.*6.784571152745185e-4;
t541 = t8.*t14.*t89.*t90.*7.970632707682899e-2;
t542 = t8.*t84.*t89.*t90.*7.970632707682899e-2;
t543 = t8.*t86.*t89.*t90.*7.970632707682899e-2;
t544 = t2.*t7.*thDot1.*thDot2.*6.872973301135055e-1;
t545 = t2.*t7.*thDot1.*thDot3.*6.872973301135055e-1;
t546 = t8.*t12.*thDot2.*thDot3.*6.872973301135055e-1;
t547 = t3.*t7.*t8.*thDot2.*thDot3.*1.356914230549037e-3;
t548 = t2.*t85.*t90.*thDot1.*thDot2.*1.59412654153658e-1;
t549 = t2.*t88.*t89.*thDot1.*thDot2.*1.59412654153658e-1;
t550 = t2.*t85.*t90.*thDot1.*thDot3.*1.59412654153658e-1;
t551 = t2.*t88.*t89.*thDot1.*thDot3.*1.59412654153658e-1;
t552 = t8.*t89.*t90.*thDot2.*thDot3.*1.59412654153658e-1;
t692 = t8.*t14.*t85.*3.074667945623095e-1;
t693 = t8.*t84.*t85.*3.074667945623095e-1;
t694 = t8.*t14.*t85.*t88.*7.970632707682899e-2;
t695 = t8.*t84.*t85.*t88.*7.970632707682899e-2;
t696 = t8.*t85.*t86.*t88.*7.970632707682899e-2;
t697 = t3.*t8.*t91.*thDot1.*thDot4.*1.356914230549037e-3;
t698 = t3.*t8.*t92.*thDot1.*thDot4.*1.356914230549037e-3;
t699 = t2.*t3.*t12.*thDot1.*thDot2.*1.356914230549037e-3;
t700 = t2.*t3.*t12.*thDot1.*thDot3.*1.356914230549037e-3;
t701 = t2.*t4.*t7.*thDot1.*thDot4.*1.356914230549037e-3;
t702 = t4.*t8.*t12.*thDot2.*thDot4.*1.356914230549037e-3;
t703 = t4.*t8.*t12.*thDot3.*thDot4.*1.356914230549037e-3;
t704 = t8.*t85.*t88.*thDot2.*thDot3.*1.59412654153658e-1;
t553 = t340+t342+t347+t348+t363-t434-t435-t436+t528+t529+t530+t531+t532+t533+t534+t535+t536+t537+t538+t539+t540+t541+t542+t543+t544+t545+t546+t547+t548+t549+t550+t551+t552-t692-t693-t694-t695-t696-t697-t698-t699-t700-t701-t702-t703-t704;
t554 = t10.*t11.*2.923071757101621e-3;
t561 = t8.*t12.*t13.*2.923071757101621e-3;
t555 = t554-t561;
t556 = t10.*t13.*2.923071757101621e-3;
t557 = t8.*t11.*t12.*2.923071757101621e-3;
t558 = t556+t557;
t559 = t2.*t3.*6.280147091832467e-4;
t562 = t4.*t7.*t8.*6.280147091832467e-4;
t560 = t559-t562;
t563 = t8.*t14.*6.104217881481557e-4;
t564 = t2.*t14.*5.391415465873457e-3;
t565 = t2.*t89.*thDot1.*thDot2.*1.691032894380261;
t566 = t8.*t14.*t89.*t90.*2.191879307959464e-1;
t567 = t8.*t84.*t89.*t90.*2.191879307959464e-1;
t568 = t8.*t86.*t89.*t90.*2.191879307959464e-1;
t569 = t2.*t85.*t90.*thDot1.*thDot2.*4.383758615918928e-1;
t570 = t2.*t88.*t89.*thDot1.*thDot2.*4.383758615918928e-1;
t571 = t2.*t85.*t90.*thDot1.*thDot3.*4.383758615918928e-1;
t572 = t2.*t88.*t89.*thDot1.*thDot3.*4.383758615918928e-1;
t573 = t8.*t89.*t90.*thDot2.*thDot3.*4.383758615918928e-1;
t574 = t8.*t14.*5.391415465873457e-3;
t575 = t2.*t14.*t85.*8.455164471901305e-1;
t576 = t2.*t84.*t85.*8.455164471901305e-1;
t577 = t8.*t89.*thDot1.*thDot2.*1.691032894380261;
t578 = t2.*t14.*t85.*t88.*2.191879307959464e-1;
t579 = t2.*t84.*t85.*t88.*2.191879307959464e-1;
t580 = t2.*t85.*t86.*t88.*2.191879307959464e-1;
t581 = t8.*t85.*t90.*thDot1.*thDot2.*4.383758615918928e-1;
t582 = t8.*t88.*t89.*thDot1.*thDot2.*4.383758615918928e-1;
t583 = t8.*t85.*t90.*thDot1.*thDot3.*4.383758615918928e-1;
t584 = t8.*t88.*t89.*thDot1.*thDot3.*4.383758615918928e-1;
t585 = t2.*t85.*t88.*thDot2.*thDot3.*4.383758615918928e-1;
t586 = t2.^2;
t587 = t8.^2;
t588 = t85.^2;
t589 = t89.^2;
t590 = t2.*t8.*t588.*1.065602502591819e-1;
t591 = t2.*t8.*t589.*2.844235507266242e-1;
t688 = t2.*t8.*2.844235507266242e-1;
t592 = t590+t591-t688;
t593 = t2.*t8.*t91.*5.436562614985332e-3;
t594 = t2.*t8.*t92.*4.50469717884937e-3;
t850 = t2.*t8.*4.50469717884937e-3;
t595 = t593+t594-t850;
t596 = t4.^2;
t717 = t8.*t14.*t85.*8.455164471901305e-1;
t718 = t8.*t84.*t85.*8.455164471901305e-1;
t719 = t8.*t14.*t85.*t88.*2.191879307959464e-1;
t720 = t8.*t84.*t85.*t88.*2.191879307959464e-1;
t721 = t8.*t85.*t86.*t88.*2.191879307959464e-1;
t722 = t8.*t85.*t88.*thDot2.*thDot3.*4.383758615918928e-1;
t597 = t340+t342+t347+t348+t349+t363+t364+t365+t366+t367+t368+t369+t370+t371+t372+t373+t377+t378+t379+t380-t434-t435-t436-t487-t488-t490-t497-t498-t499-t500-t501-t502-t503+t563+t564+t565+t566+t567+t568+t569+t570+t571+t572+t573-t717-t718-t719-t720-t721-t722;
t598 = t92.*t586.*2.36837910197578e-2;
t599 = t31.*t525;
t600 = t39.*t522;
t601 = t598+t599+t600;
t603 = th2+th3+th4;
t604 = sin(t603);
t605 = th2+th3-th4;
t606 = sin(t605);
t607 = thDot5.^2;
t608 = t107.*t394.*1.994855465224146;
t609 = t33.*t280.*1.900321864457165e1;
t610 = t113.*t397.*1.900321864457165e1;
t611 = t7.*t84.*6.013658974882553e-1;
t612 = t7.*t86.*6.013658974882553e-1;
t613 = t12.*t84.*1.468199126656079;
t614 = t12.*t86.*1.468199126656079;
t615 = t12.*thDot2.*thDot3.*2.936398253312157;
t616 = t606.*thDot2.*thDot4.*1.187261914627176e-3;
t617 = t606.*thDot3.*thDot4.*1.187261914627176e-3;
t618 = t84.*t85.*t88.*3.436486650567527e-1;
t619 = t85.*t86.*t88.*3.436486650567527e-1;
t620 = t84.*t85.*t90.*7.970632707682899e-2;
t621 = t84.*t88.*t89.*7.970632707682899e-2;
t622 = t85.*t86.*t90.*7.970632707682899e-2;
t623 = t86.*t88.*t89.*7.970632707682899e-2;
t624 = t7.*thDot2.*thDot3.*1.202731794976511;
t625 = t85.*t90.*thDot2.*thDot3.*1.59412654153658e-1;
t626 = t88.*t89.*thDot2.*thDot3.*1.59412654153658e-1;
t627 = t13.*t84.*t85.*t88.*1.199966622536514e-4;
t628 = t13.*t85.*t86.*t88.*1.199966622536514e-4;
t629 = t13.*t85.*t88.*t607.*1.199966622536514e-4;
t630 = t4.*t84.*t85.*t90.*2.265025256144936e-4;
t631 = t4.*t84.*t88.*t89.*2.265025256144936e-4;
t632 = t4.*t85.*t86.*t90.*2.265025256144936e-4;
t633 = t4.*t86.*t88.*t89.*2.265025256144936e-4;
t634 = t4.*t85.*t87.*t90.*2.265025256144936e-4;
t635 = t4.*t87.*t88.*t89.*2.265025256144936e-4;
t636 = t85.*t88.*thDot2.*thDot3.*6.872973301135055e-1;
t637 = t3.*t11.*t84.*t85.*t90.*1.199966622536514e-4;
t638 = t3.*t11.*t84.*t88.*t89.*1.199966622536514e-4;
t639 = t3.*t11.*t85.*t86.*t90.*1.199966622536514e-4;
t640 = t3.*t11.*t86.*t88.*t89.*1.199966622536514e-4;
t641 = t3.*t11.*t85.*t87.*t90.*1.199966622536514e-4;
t642 = t3.*t11.*t87.*t88.*t89.*1.199966622536514e-4;
t643 = t3.*t11.*t85.*t90.*t607.*1.199966622536514e-4;
t644 = t3.*t11.*t88.*t89.*t607.*1.199966622536514e-4;
t645 = t13.*t85.*t88.*thDot2.*thDot3.*2.399933245073028e-4;
t646 = t11.*t85.*t90.*thDot2.*thDot5.*2.399933245073028e-4;
t647 = t11.*t88.*t89.*thDot2.*thDot5.*2.399933245073028e-4;
t648 = t11.*t85.*t90.*thDot3.*thDot5.*2.399933245073028e-4;
t649 = t11.*t88.*t89.*thDot3.*thDot5.*2.399933245073028e-4;
t650 = t4.*t85.*t90.*thDot2.*thDot3.*4.530050512289873e-4;
t651 = t4.*t88.*t89.*thDot2.*thDot3.*4.530050512289873e-4;
t652 = t3.*t89.*t90.*thDot2.*thDot4.*4.530050512289873e-4;
t653 = t3.*t89.*t90.*thDot3.*thDot4.*4.530050512289873e-4;
t654 = t4.*t89.*t90.*thDot2.*thDot4.*1.356914230549037e-3;
t655 = t4.*t89.*t90.*thDot3.*thDot4.*1.356914230549037e-3;
t656 = t3.*t11.*t85.*t90.*thDot2.*thDot3.*2.399933245073028e-4;
t657 = t3.*t11.*t88.*t89.*thDot2.*thDot3.*2.399933245073028e-4;
t658 = t4.*t11.*t85.*t88.*thDot2.*thDot4.*2.399933245073028e-4;
t659 = t3.*t13.*t85.*t88.*thDot2.*thDot5.*2.399933245073028e-4;
t660 = t4.*t11.*t85.*t88.*thDot3.*thDot4.*2.399933245073028e-4;
t661 = t3.*t13.*t85.*t88.*thDot3.*thDot5.*2.399933245073028e-4;
t662 = t108.*t339.*1.994855465224146;
t663 = t197.*t412;
t664 = t189.*t416;
t956 = t64.*t195;
t665 = t663+t664-t956;
t666 = t189.*t192;
t667 = t58.*t195;
t668 = t197.*t199;
t669 = t666+t667+t668;
t670 = t62.*t669;
t671 = t189.*t335;
t672 = t41.*t195;
t911 = t197.*t330;
t673 = t671+t672-t911;
t674 = t73.*t673;
t1007 = t66.*t665;
t675 = t670+t674-t1007;
t861 = t8.*t14.*t85.*5.971038255043736;
t862 = t8.*t84.*t85.*5.971038255043736;
t676 = t340+t342+t347+t348+t349+t363+t364+t365+t366+t367+t368+t369+t370+t371+t372+t373+t374+t375+t376+t377+t378+t379+t380+t381+t382+t383+t384+t385+t398-t434-t435-t436-t486-t487-t488-t489-t490-t493-t494-t495-t496-t497-t498-t499-t500-t501-t502-t503-t504+t518+t519+t520-t861-t862;
t677 = t31.*t317;
t678 = t54.*t320;
t679 = t41.*t322;
t680 = t677+t678+t679;
t681 = t4.*t7.*t8.*1.244265463592368e-3;
t682 = t8.*t12.*t13.*1.37348971869607e-3;
t1010 = t2.*t3.*1.244265463592368e-3;
t1011 = t10.*t11.*1.37348971869607e-3;
t683 = t93+t94+t681+t682-t1010-t1011;
t684 = t586.*2.844235507266242e-1;
t685 = t587.*t588.*1.065602502591819e-1;
t686 = t587.*t589.*2.844235507266242e-1;
t687 = t684+t685+t686;
t689 = t8.*t592.*thDot2;
t690 = t8.*t85.*t89.*thDot1.*1.778633004674423e-1;
t691 = t689+t690-t2.*t687.*thDot2;
t705 = t91.*2.36837910197578e-2;
t706 = t3.^2;
t707 = t92.*t706.*1.557550994534973e-1;
t708 = t92.*t596.*1.557550994534973e-1;
t709 = t705+t707+t708;
t710 = t4.*t12.*t17.*1.557550994534973e-1;
t893 = t3.*t10.*t12.*1.557550994534973e-1;
t711 = t516+t710-t893;
t712 = t3.*t12.*t39.*1.557550994534973e-1;
t894 = t4.*t12.*t31.*1.557550994534973e-1;
t713 = t526+t712-t894;
t714 = t10.*t522;
t715 = t17.*t525;
t829 = t2.*t8.*t92.*2.36837910197578e-2;
t716 = t714+t715-t829;
t723 = t66.*(t341-t392).*1.139953928995173;
t724 = t192.*t420;
t725 = t58.*t422;
t951 = t199.*t425;
t726 = t724+t725-t951;
t727 = t26.*t313;
t728 = t64.*t310;
t729 = t92.*t596.*6.280147091832467e-4;
t730 = t727+t728+t729;
t731 = t58.*t310;
t732 = t4.*t12.*t17.*6.280147091832467e-4;
t906 = t20.*t313;
t733 = t731+t732-t906;
t734 = t41.*t310;
t735 = t4.*t12.*t31.*6.280147091832467e-4;
t908 = t54.*t313;
t736 = t734+t735-t908;
t737 = t340+t347+t348+t349+t363+t364+t365+t366+t367+t368+t369+t370+t371+t372+t373+t374+t375+t376+t377+t378+t379+t380+t381+t382+t383+t384+t385+t386+t391+t398+t399+t400+t401-t434-t435-t436+t485-t486-t487-t488-t489-t490-t491-t492-t493-t494-t495-t496-t497-t498-t499-t500-t501-t502-t503-t504+t723;
t741 = t2.*3.899910832955465e-3;
t742 = t169+t170+t741;
t743 = t84.*t89.*5.971038255043736;
t747 = t140.*t314.*1.994855465224146;
t749 = t62.*t602.*1.139953928995173;
t750 = t84.*t604.*5.936309573135882e-4;
t751 = t86.*t604.*5.936309573135882e-4;
t752 = t87.*t604.*5.936309573135882e-4;
t753 = t114.*t344.*1.900321864457165e1;
t754 = t179.*t290.*1.900321864457165e1;
t755 = t73.*t244.*1.139953928995173;
t756 = t104.*t275.*1.994855465224146;
t757 = t50.*t337.*1.139953928995173;
t758 = t84.*t606.*5.936309573135882e-4;
t759 = t86.*t606.*5.936309573135882e-4;
t760 = t87.*t606.*5.936309573135882e-4;
t761 = t71.*t231.*1.139953928995173;
t762 = t84.*t89.*t90.*3.436486650567527e-1;
t763 = t86.*t89.*t90.*3.436486650567527e-1;
t765 = t604.*thDot2.*thDot3.*1.187261914627176e-3;
t766 = t604.*thDot2.*thDot4.*1.187261914627176e-3;
t767 = t604.*thDot3.*thDot4.*1.187261914627176e-3;
t768 = t606.*thDot2.*thDot3.*1.187261914627176e-3;
t769 = t89.*t90.*thDot2.*thDot3.*6.872973301135055e-1;
t771 = t3.*t84.*t85.*t90.*6.784571152745185e-4;
t772 = t3.*t84.*t88.*t89.*6.784571152745185e-4;
t773 = t3.*t85.*t86.*t90.*6.784571152745185e-4;
t774 = t3.*t86.*t88.*t89.*6.784571152745185e-4;
t775 = t3.*t85.*t87.*t90.*6.784571152745185e-4;
t776 = t3.*t87.*t88.*t89.*6.784571152745185e-4;
t777 = t13.*t84.*t89.*t90.*1.199966622536514e-4;
t778 = t13.*t86.*t89.*t90.*1.199966622536514e-4;
t779 = t13.*t89.*t90.*t607.*1.199966622536514e-4;
t780 = t3.*t85.*t88.*thDot2.*thDot4.*4.530050512289873e-4;
t781 = t3.*t85.*t88.*thDot3.*thDot4.*4.530050512289873e-4;
t782 = t3.*t85.*t90.*thDot2.*thDot3.*1.356914230549037e-3;
t783 = t3.*t88.*t89.*thDot2.*thDot3.*1.356914230549037e-3;
t784 = t4.*t85.*t88.*thDot2.*thDot4.*1.356914230549037e-3;
t785 = t4.*t85.*t88.*thDot3.*thDot4.*1.356914230549037e-3;
t786 = t13.*t89.*t90.*thDot2.*thDot3.*2.399933245073028e-4;
t787 = t4.*t11.*t89.*t90.*thDot2.*thDot4.*2.399933245073028e-4;
t788 = t3.*t13.*t89.*t90.*thDot2.*thDot5.*2.399933245073028e-4;
t789 = t4.*t11.*t89.*t90.*thDot3.*thDot4.*2.399933245073028e-4;
t790 = t3.*t13.*t89.*t90.*thDot3.*thDot5.*2.399933245073028e-4;
t791 = t4.*t13.*t85.*t90.*thDot4.*thDot5.*2.399933245073028e-4;
t792 = t4.*t13.*t88.*t89.*thDot4.*thDot5.*2.399933245073028e-4;
t744 = t608+t609+t610+t611+t612+t613+t614+t615+t616+t617+t618+t619+t620+t621+t622+t623+t624+t625+t626+t627+t628+t629+t630+t631+t632+t633+t634+t635+t636+t637+t638+t639+t640+t641+t642+t643+t644+t645+t646+t647+t648+t649+t650+t651+t652+t653+t654+t655+t656+t657+t658+t659+t660+t661+t662+t743-t747-t749-t750-t751-t752-t753-t754-t755-t756-t757-t758-t759-t760-t761-t762-t763-t765-t766-t767-t768-t769-t771-t772-t773-t774-t775-t776-t777-t778-t779-t780-t781-t782-t783-t784-t785-t786-t787-t788-t789-t790-t791-t792+2.169526747801515e2;
t745 = t2.*3.540643940569388e-4;
t746 = t166+t745-t8.*t85.*1.301446134121834e-1;
t748 = t84.*t89.*7.153708691033507;
t764 = t2.*t27.*t390.*4.38483060303202;
t770 = t8.*t27.*t230.*thDot1.*4.38483060303202;
t793 = t328.*t412;
t794 = t64.*t325;
t795 = t332.*t416;
t796 = t793+t794+t795;
t797 = t199.*t328;
t798 = t192.*t332;
t947 = t58.*t325;
t799 = t797+t798-t947;
t800 = t41.*t325;
t801 = t328.*t330;
t948 = t332.*t335;
t802 = t800+t801-t948;
t803 = t31.*t560;
t804 = t54.*t555;
t805 = t41.*t558;
t806 = t803+t804+t805;
t807 = t104.*t806;
t808 = t64.*t558;
t809 = t4.*t12.*t560;
t940 = t26.*t555;
t810 = t808+t809-t940;
t811 = t36.*t810;
t812 = t58.*t558;
t813 = t20.*t555;
t814 = t17.*t560;
t815 = t812+t813+t814;
t816 = t108.*t815;
t817 = t807+t811+t816;
t818 = t335.*t420;
t819 = t41.*t422;
t820 = t330.*t425;
t821 = t818+t819+t820;
t822 = t64.*t322;
t823 = t4.*t12.*t317;
t875 = t26.*t320;
t824 = t822+t823-t875;
t825 = t108.*(t338-t387).*1.994855465224146;
t883 = t8.*t27.*t404.*4.38483060303202;
t886 = t2.*t27.*t172.*thDot1.*4.38483060303202;
t826 = t608+t609+t610+t611+t612+t613+t614+t615+t616+t617+t618+t619+t620+t621+t622+t623+t624+t625+t626+t627+t628+t629+t630+t631+t632+t633+t634+t635+t636+t637+t638+t639+t640+t641+t642+t643+t644+t645+t646+t647+t648+t649+t650+t651+t652+t653+t654+t655+t656+t657+t658+t659+t660+t661-t747+t748-t749-t750-t751-t752-t753-t754-t755-t756-t757-t758-t759-t760-t761-t762-t763+t764-t765-t766-t767-t768-t769+t770-t771-t772-t773-t774-t775-t776-t777-t778-t779-t780-t781-t782-t783-t784-t785-t786-t787-t788-t789-t790-t791-t792+t825-t883-t886+2.599240146898653e2;
t827 = t31.*t515;
t828 = t39.*t513;
t830 = t4.*t12.*t515;
t974 = t3.*t12.*t513;
t831 = t516+t830-t974;
t832 = t92.*t587.*2.36837910197578e-2;
t833 = t10.*t513;
t834 = t17.*t515;
t835 = t832+t833+t834;
t836 = t114.*t835;
t837 = t2.*t4.*1.889179028920907e-3;
t838 = t8.*t12.*1.51663096460419e-1;
t839 = t3.*t7.*t8.*1.889179028920907e-3;
t840 = t112-t205+t837+t838+t839;
t841 = t84.*t89.*8.455164471901305e-1;
t842 = t12.*t84.*1.394816037191174e-1;
t843 = t12.*t86.*1.394816037191174e-1;
t844 = t12.*thDot2.*thDot3.*2.789632074382348e-1;
t845 = t586.*4.50469717884937e-3;
t846 = t91.*t587.*5.436562614985332e-3;
t847 = t92.*t587.*4.50469717884937e-3;
t848 = t845+t846+t847;
t849 = t2.*t27.*t848;
t851 = t7.*t8.*t12.*thDot1.*9.31865436135962e-4;
t1027 = t8.*t27.*t595;
t852 = t849+t851-t1027;
t853 = t64.*t422;
t854 = t412.*t425;
t950 = t416.*t420;
t855 = t853+t854-t950;
t856 = t84.*t89.*3.074667945623095e-1;
t857 = t17.*t317;
t858 = t58.*t322;
t859 = t20.*t320;
t860 = t857+t858+t859;
t863 = t3.*t12.*t522;
t961 = t4.*t12.*t525;
t864 = t526+t863-t961;
t865 = t587.*4.50469717884937e-3;
t866 = t91.*t586.*5.436562614985332e-3;
t867 = t92.*t586.*4.50469717884937e-3;
t868 = t865+t866+t867;
t869 = t587.*2.844235507266242e-1;
t870 = t586.*t588.*1.065602502591819e-1;
t871 = t586.*t589.*2.844235507266242e-1;
t872 = t869+t870+t871;
t873 = t108.*t860;
t874 = t104.*t680;
t876 = t36.*t824;
t877 = t873+t874+t876;
t878 = t7.*t13.*1.37348971869607e-3;
t879 = t3.*t11.*t12.*1.37348971869607e-3;
t978 = t4.*t12.*1.244265463592368e-3;
t880 = t128-t215+t878+t879-t978;
t923 = t2.*t14.*2.219760847427988e-4;
t924 = t2.*t12.*t14.*3.436486650567527e-1;
t925 = t2.*t12.*t84.*3.436486650567527e-1;
t926 = t2.*t12.*t86.*3.436486650567527e-1;
t927 = t2.*t3.*t7.*t14.*6.784571152745185e-4;
t928 = t2.*t3.*t7.*t84.*6.784571152745185e-4;
t929 = t2.*t3.*t7.*t86.*6.784571152745185e-4;
t930 = t2.*t3.*t7.*t87.*6.784571152745185e-4;
t931 = t2.*t14.*t89.*t90.*7.970632707682899e-2;
t932 = t2.*t84.*t89.*t90.*7.970632707682899e-2;
t933 = t2.*t86.*t89.*t90.*7.970632707682899e-2;
t934 = t2.*t12.*thDot2.*thDot3.*6.872973301135055e-1;
t935 = t3.*t8.*t12.*thDot1.*thDot2.*1.356914230549037e-3;
t936 = t3.*t8.*t12.*thDot1.*thDot3.*1.356914230549037e-3;
t937 = t4.*t7.*t8.*thDot1.*thDot4.*1.356914230549037e-3;
t938 = t2.*t3.*t7.*thDot2.*thDot3.*1.356914230549037e-3;
t939 = t2.*t89.*t90.*thDot2.*thDot3.*1.59412654153658e-1;
t881 = t213+t241+t245+t250+t259+t271+t283-t444+t464+t465+t466+t467+t468+t469+t470+t471+t472+t473+t474+t475+t476+t477+t478+t479+t480+t481+t482+t483+t484-t923-t924-t925-t926-t927-t928-t929-t930-t931-t932-t933-t934-t935-t936-t937-t938-t939;
t882 = t618+t619+t620+t621+t622+t623+t625+t626+t627+t628+t629+t630+t631+t632+t633+t634+t635+t636+t637+t638+t639+t640+t641+t642+t643+t644+t645+t646+t647+t648+t649+t650+t651+t652+t653+t654+t655+t656+t657+t658+t659+t660+t661-t749-t755-t757-t761-t762-t763-t769-t771-t772-t773-t774-t775-t776-t777-t778-t779-t780-t781-t782-t783-t784-t785-t786-t787-t788-t789-t790-t791-t792+t856+1.11715485041527e1;
t884 = t8.*t441.*thDot2.*3.812773007925995e1;
t885 = t2.*t167.*thDot1.*thDot2.*3.812773007925995e1;
t970 = t2.*t14.*4.310799465649219e-3;
t887 = t213+t241+t245+t250+t259+t271+t272+t276+t277+t281+t283+t287+t291+t292+t293+t294+t295+t296+t297+t298+t299+t300+t301+t302+t303+t304+t305+t306+t307+t308-t439-t444-t447-t448-t449-t450-t451-t452-t453-t454-t455-t456-t457-t458-t459-t460-t461-t462-t463+t507+t508+t509+t510-t970;
t888 = t3.*t12.*1.889179028920907e-3;
t982 = t7.*1.51663096460419e-1;
t889 = t162+t888-t982;
t913 = t2.*t14.*6.104217881481557e-4;
t914 = t2.*t14.*t89.*t90.*2.191879307959464e-1;
t915 = t2.*t84.*t89.*t90.*2.191879307959464e-1;
t916 = t2.*t86.*t89.*t90.*2.191879307959464e-1;
t917 = t2.*t89.*t90.*thDot2.*thDot3.*4.383758615918928e-1;
t890 = t213+t241+t245+t250+t259+t271+t276+t277+t283+t287+t292+t293+t297+t298+t299+t300+t301+t302+t303-t439-t444-t447-t448-t449-t450-t451-t452-t453-t458-t459-t460-t461-t462+t574+t575+t576+t577+t578+t579+t580+t581+t582+t583+t584+t585-t913-t914-t915-t916-t917;
t891 = t608+t611+t612+t616+t617+t618+t619+t620+t621+t622+t623+t624+t625+t626+t627+t628+t629+t630+t631+t632+t633+t634+t635+t636+t637+t638+t639+t640+t641+t642+t643+t644+t645+t646+t647+t648+t649+t650+t651+t652+t653+t654+t655+t656+t657+t658+t659+t660+t661-t747-t749-t750-t751-t752-t755-t756-t757-t758-t759-t760-t761-t762-t763-t765-t766-t767-t768-t769-t771-t772-t773-t774-t775-t776-t777-t778-t779-t780-t781-t782-t783-t784-t785-t786-t787-t788-t789-t790-t791-t792+t825+t841+t842+t843+t844+3.072113206334932e1;
t892 = t109.*t709;
t895 = t33.*t713;
t984 = t114.*t711;
t896 = t892+t895-t984;
t897 = t3.*t8.*1.244265463592368e-3;
t898 = t11.*t39.*1.37348971869607e-3;
t899 = t2.*t4.*t7.*1.244265463592368e-3;
t900 = t2.*t12.*t13.*1.37348971869607e-3;
t901 = t138-t216+t897+t898+t899+t900;
t902 = t8.*t872.*thDot2;
t903 = t2.*t85.*t89.*thDot1.*1.778633004674423e-1;
t904 = t902+t903-t2.*t592.*thDot2;
t905 = t36.*t730;
t907 = t108.*t733;
t909 = t104.*t736;
t910 = t905+t907+t909;
t912 = t827+t828-t829;
t919 = t89.*1.301446134121834e-1;
t920 = t180+t919;
t991 = t8.*3.899910832955465e-3;
t941 = t227+t228-t991;
t942 = t608+t609+t610+t611+t612+t613+t614+t615+t616+t617+t618+t619+t620+t621+t622+t623+t624+t625+t626+t627+t628+t629+t630+t631+t632+t633+t634+t635+t636+t637+t638+t639+t640+t641+t642+t643+t644+t645+t646+t647+t648+t649+t650+t651+t652+t653+t654+t655+t656+t657+t658+t659+t660+t661+t743-t747-t749-t750-t751-t752-t753-t754-t755-t756-t757-t758-t759-t760-t761-t762-t763-t765-t766-t767-t768-t769-t771-t772-t773-t774-t775-t776-t777-t778-t779-t780-t781-t782-t783-t784-t785-t786-t787-t788-t789-t790-t791-t792+t825+2.169526747801515e2;
t943 = t8.*3.540643940569388e-4;
t944 = t2.*t85.*1.301446134121834e-1;
t945 = -t225+t943+t944;
t946 = t66.*t796;
t949 = t73.*t802;
t952 = t62.*t726;
t953 = t73.*t821;
t954 = t66.*t855;
t955 = t952+t953+t954;
t957 = t2.*t12.*1.51663096460419e-1;
t958 = t2.*t3.*t7.*1.889179028920907e-3;
t997 = t4.*t8.*1.889179028920907e-3;
t959 = t176+t178+t957+t958-t997;
t960 = t114.*t716;
t962 = t109.*t864;
t963 = t33.*t601;
t964 = t960+t962+t963;
t965 = t2.*t27.*t595;
t966 = t2.*t7.*t12.*thDot1.*9.31865436135962e-4;
t1001 = t8.*t27.*t868;
t967 = t965+t966-t1001;
t968 = t12.*3.689996292735745e-2;
t969 = t173-t968;
t971 = t91.*4.50469717884937e-3;
t972 = t92.*5.436562614985332e-3;
t973 = t971+t972;
t975 = t588.*2.844235507266242e-1;
t976 = t589.*1.065602502591819e-1;
t977 = t975+t976;
t979 = t880.*t881;
t980 = t17.*thDot5.*(1.0./1.0e1);
t981 = t164.*t887;
t983 = t231.*t669;
t985 = t882.*t901;
t986 = t104.*t910;
t987 = t175.*t438;
t988 = t58.*thDot6.*(1.0./2.0e1);
t989 = t78.*t881;
t990 = t134.*t810;
t1017 = t62.*t799;
t1018 = t946+t949-t1017;
t992 = t73.*t1018;
t993 = t123.*t665;
t994 = t2.*thDot3.*3.0;
t995 = t314.*t815;
t996 = t290.*t835;
t998 = t891.*t959;
t999 = t109.*t964;
t1000 = t230.*t826;
t1002 = t8.*t12.*thDot4.*(1.0./1.0e1);
t1003 = t2.*t27.*t595.*thDot1;
t1004 = t8.*t27.*t848.*thDot1;
t1005 = t340+t347+t348+t349+t363+t364+t365+t366+t367+t368+t369+t370+t371+t372+t373+t377+t378+t379+t380-t434-t435-t436-t487-t488-t490-t497-t498-t499-t500-t501-t502-t503+t563+t564+t565+t566+t567+t568+t569+t570+t571+t572+t573-t717-t718-t719-t720-t721-t722+t723;
t1006 = t31.*thDot5.*(1.0./1.0e1);
t1008 = t66.*t675;
t1009 = t340+t347+t348+t349+t363+t364+t365+t366+t367+t368+t369+t370+t371+t372+t373+t374+t375+t376+t377+t378+t379+t380+t381+t382+t383+t384+t385+t398-t434-t435-t436-t486-t487-t488-t489-t490-t493-t494-t495-t496-t497-t498-t499-t500-t501-t502-t503-t504+t518+t519+t520+t723-t861-t862;
t1012 = t340+t347+t348+t363-t434-t435-t436+t528+t529+t530+t531+t532+t533+t534+t535+t536+t537+t538+t539+t540+t541+t542+t543+t544+t545+t546+t547+t548+t549+t550+t551+t552-t692-t693-t694-t695-t696-t697-t698-t699-t700-t701-t702-t703-t704+t723;
t1013 = t114.*t896;
t1014 = t290.*t716;
t1015 = t131.*t1005;
t1016 = t231.*t726;
t1019 = t41.*thDot6.*(1.0./2.0e1);
t1020 = t36.*t817;
t1021 = t8.*thDot3.*3.0;
t1022 = t134.*t824;
t1023 = t172.*t826;
t1024 = t33.*t912;
t1039 = t109.*t831;
t1025 = t836+t1024-t1039;
t1026 = t840.*t891;
t1028 = t50.*t882;
t1029 = t314.*t860;
t1030 = t969.*t1009;
t1031 = t2.*t27.*t973.*thDot1;
t1032 = t12.*t27.*t864.*thDot4;
t1033 = t231.*t799;
t1034 = t73.*t675;
t1035 = t337.*t802;
t1036 = t394.*t736;
t1037 = t123.*t796;
t1038 = t50.*t881;
t1040 = t104.*t817;
t1041 = t12.*t27.*t709.*thDot4;
t1042 = t889.*t1005;
t1043 = t683.*t882;
t1044 = (t329-t427).*(t423-t426);
t1045 = t818+t819+t1044;
t1046 = t66.*(t853+t854-t950);
t1047 = t73.*t1045;
t1048 = t952+t1046+t1047;
t1049 = t73.*(t946+t949-t1017);
t1050 = t134.*t730;
t1051 = t314.*t733;
t1052 = t108.*t877;
t1053 = t62.*t1048;
t1054 = t71.*t1012;
t1055 = t64.*thDot6.*(1.0./2.0e1);
t1056 = t140.*t1005;
t1057 = t107.*t890;
t1058 = t4.*t12.*thDot5.*(1.0./1.0e1);
